simulink model "ModeAdjust"  (R2018b)
settings: Solver=FixedStepDiscrete  StartTime=0.0  StopTime=inf  FixedStep=0.01  RelTol=1e-3
undefined symbols (not defined in the file or in its folder): IfKeSMSbSeatMovBkRclnEnable_Val, IfKeSMSbSeatMovFrwdBkwdEnable_Val, IfKeSMSbSeatMovFtrstEnable_Val, IfKeSMSbSeatMovHdrstFrwdBkwdEnable_Val, IfKeSMSbSeatMovHdUpwdDnwdEnable_Val, IfKeSMSbSeatMovLgrstEnable_Val, IfKeSMSbSeatMovLtwdRtwdEnable_Val, IfVeSMSeStNumConfig, KeSMSbArmscreenMovEnable_Val, KeSMSbSeatMovLgrstExpdEnable_Val, KeSMSuFirstRwStBackPosDelta_Val, KeSMSuFirstRwStBackPosTolr_Val, KeSMSuFirstRwStCushFrntPosDelta_Val, KeSMSuFirstRwStCushFrntPosTolr_Val, KeSMSuFirstRwStCushRePosDelta_Val, KeSMSuFirstRwStCushRePosTolr_Val, KeSMSuFirstRwStFootrestPosDelta_Val, KeSMSuFirstRwStFootrestPosTolr_Val, KeSMSuFirstRwStFwdBkwdPosDelta_Val, KeSMSuFirstRwStFwdBkwdPosTolr_Val, KeSMSuMdMotFinshdTm_Val, KeSMSuMdRetryTm1_Val, KeSMSuModeReqDurgTm_Val, KeSMSuSecRwStArmTochPosDelta_Val, KeSMSuSecRwStArmTochPosTolr_Val, KeSMSuSecRwStBackPosDelta_Val, KeSMSuSecRwStBackPosTolr_Val, KeSMSuSecRwStFtrstUpwdDnwdPosDelta_Val, KeSMSuSecRwStFtrstUpwdDnwdPosTolr_Val, KeSMSuSecRwStFwdBkwdPosDelta_Val, KeSMSuSecRwStFwdBkwdPosTolr_Val, KeSMSuSecRwStHeadrestFwdBkwdPosDelta_Val, KeSMSuSecRwStHeadrestFwdBkwdPosTolr_Val, KeSMSuSecRwStHeadrestUpwdDwnwdPosDelta_Val, KeSMSuSecRwStHeadrestUpwdDwnwdPosTolr_Val, KeSMSuSecRwStLegrestInOutPosDelta_Val, KeSMSuSecRwStLegrestInOutPosTolr_Val, KeSMSuSecRwStLegrestUpwdDwnwdPosDelta_Val, KeSMSuSecRwStLegrestUpwdDwnwdPosTolr_Val, KeSMSuSecRwStLwdRwdPosDelta_Val, KeSMSuSecRwStLwdRwdPosTolr_Val, KeSMSuSecRwStVIPFtrstRefAngle_Val, KeSMSuThirdRwStFwdBkwdPosDelta_Val, KeSMSuThirdRwStFwdBkwdPosTolr_Val, KeSMSuThrdRwCushFoldPosDelta_Val, KeSMSuThrdRwCushFoldPosTolr_Val, KeSMSuThrdRwStBackPosDelta_Val, KeSMSuThrdRwStBackPosTolr_Val, KeSMSw4SLegrstCloseMdSecRwLtStFtrstUpwdDnwdPos_Val, KeSMSw4SLegrstCloseMdSecRwLtStFtrstUpwdDnwdPosMax_Val, KeSMSw4SLegrstCloseMdSecRwLtStFtrstUpwdDnwdPosMin_Val, KeSMSw4SLegrstCloseMdSecRwLtStLgrstOtwdInwdPos_Val, KeSMSw4SLegrstCloseMdSecRwLtStLgrstOtwdInwdPosMax_Val, KeSMSw4SLegrstCloseMdSecRwLtStLgrstOtwdInwdPosMin_Val, KeSMSw4SLegrstCloseMdSecRwLtStLgrstUpwdDnwdPos_Val, KeSMSw4SLegrstCloseMdSecRwLtStLgrstUpwdDnwdPosMax_Val, KeSMSw4SLegrstCloseMdSecRwLtStLgrstUpwdDnwdPosMin_Val, KeSMSw4SLegrstCloseMdSecRwRtStFtrstUpwdDnwdPos_Val, KeSMSw4SLegrstCloseMdSecRwRtStFtrstUpwdDnwdPosMax_Val, KeSMSw4SLegrstCloseMdSecRwRtStFtrstUpwdDnwdPosMin_Val ... (+1138)
libraries: Lib x401
(part 5 of 35)

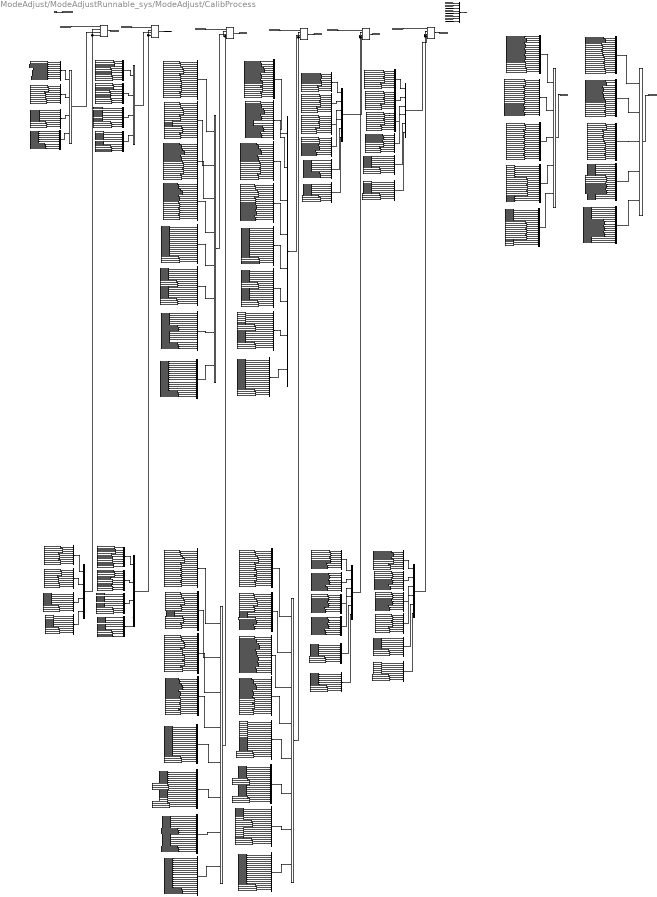
== system ModeAdjust/ModeAdjustRunnable_sys/ModeAdjust/CalibProcess ==
  note: 7S
  StNumConfig : Inport
  Bus Creator{,2..4,16..18,20..24,27..28,30..31,43..46,48..51,53..56,63..64,71..72,81..88} (40 alike) : BusCreator  Inputs=9
  Bus Creator{1,5,29,32} (4 alike) : BusCreator  Inputs=4
  Bus Creator{6..13,33..36,38..41,57..62,65..66,73..78,89..100} (42 alike) : BusCreator  Inputs=18
  Bus Creator{14..15,26,37,42} (5 alike) : BusCreator  Inputs=8
  Bus Creator{19,25,47,52} (4 alike) : BusCreator  Inputs=6
  Bus Creator79 : BusCreator  Inputs=5
  Bus Creator80 : BusCreator  Inputs=5
  Multiport Switch{1..4,6..7} (6 alike) : MultiPortSwitch  DataPortOrder=Specify indices  DataPortIndices={IfVeSMSeStNumConfig.SeatNum4Config,IfVeSMSeStNumConfig.SeatNum6Config,IfVeSMSeStNumConfig.SeatNum7Config}  DiagnosticForDefault=None
  PA_KeSMSw4SLegrstCloseMdSecRwLtStFtrstUpwdDnwdPosMax_Val : Constant  Value=KeSMSw4SLegrstCloseMdSecRwLtStFtrstUpwdDnwdPosMax_Val
  PA_KeSMSw4SLegrstCloseMdSecRwLtStFtrstUpwdDnwdPosMin_Val : Constant  Value=KeSMSw4SLegrstCloseMdSecRwLtStFtrstUpwdDnwdPosMin_Val
  PA_KeSMSw4SLegrstCloseMdSecRwLtStFtrstUpwdDnwdPos_Val : Constant  Value=KeSMSw4SLegrstCloseMdSecRwLtStFtrstUpwdDnwdPos_Val
  PA_KeSMSw4SLegrstCloseMdSecRwLtStLgrstOtwdInwdPosMax_Val : Constant  Value=KeSMSw4SLegrstCloseMdSecRwLtStLgrstOtwdInwdPosMax_Val
  PA_KeSMSw4SLegrstCloseMdSecRwLtStLgrstOtwdInwdPosMin_Val : Constant  Value=KeSMSw4SLegrstCloseMdSecRwLtStLgrstOtwdInwdPosMin_Val
  PA_KeSMSw4SLegrstCloseMdSecRwLtStLgrstOtwdInwdPos_Val : Constant  Value=KeSMSw4SLegrstCloseMdSecRwLtStLgrstOtwdInwdPos_Val
  PA_KeSMSw4SLegrstCloseMdSecRwLtStLgrstUpwdDnwdPosMax_Val : Constant  Value=KeSMSw4SLegrstCloseMdSecRwLtStLgrstUpwdDnwdPosMax_Val
  PA_KeSMSw4SLegrstCloseMdSecRwLtStLgrstUpwdDnwdPosMin_Val : Constant  Value=KeSMSw4SLegrstCloseMdSecRwLtStLgrstUpwdDnwdPosMin_Val
  PA_KeSMSw4SLegrstCloseMdSecRwLtStLgrstUpwdDnwdPos_Val : Constant  Value=KeSMSw4SLegrstCloseMdSecRwLtStLgrstUpwdDnwdPos_Val
  PA_KeSMSw4SLegrstCloseMdSecRwRtStFtrstUpwdDnwdPosMax_Val : Constant  Value=KeSMSw4SLegrstCloseMdSecRwRtStFtrstUpwdDnwdPosMax_Val
  PA_KeSMSw4SLegrstCloseMdSecRwRtStFtrstUpwdDnwdPosMin_Val : Constant  Value=KeSMSw4SLegrstCloseMdSecRwRtStFtrstUpwdDnwdPosMin_Val
  PA_KeSMSw4SLegrstCloseMdSecRwRtStFtrstUpwdDnwdPos_Val : Constant  Value=KeSMSw4SLegrstCloseMdSecRwRtStFtrstUpwdDnwdPos_Val
  PA_KeSMSw4SLegrstCloseMdSecRwRtStLgrstOtwdInwdPosMax_Val : Constant  Value=KeSMSw4SLegrstCloseMdSecRwRtStLgrstOtwdInwdPosMax_Val
  PA_KeSMSw4SLegrstCloseMdSecRwRtStLgrstOtwdInwdPosMin_Val : Constant  Value=KeSMSw4SLegrstCloseMdSecRwRtStLgrstOtwdInwdPosMin_Val
  PA_KeSMSw4SLegrstCloseMdSecRwRtStLgrstOtwdInwdPos_Val : Constant  Value=KeSMSw4SLegrstCloseMdSecRwRtStLgrstOtwdInwdPos_Val
  PA_KeSMSw4SLegrstCloseMdSecRwRtStLgrstUpwdDnwdPosMax_Val : Constant  Value=KeSMSw4SLegrstCloseMdSecRwRtStLgrstUpwdDnwdPosMax_Val
  PA_KeSMSw4SLegrstCloseMdSecRwRtStLgrstUpwdDnwdPosMin_Val : Constant  Value=KeSMSw4SLegrstCloseMdSecRwRtStLgrstUpwdDnwdPosMin_Val
  PA_KeSMSw4SLegrstCloseMdSecRwRtStLgrstUpwdDnwdPos_Val : Constant  Value=KeSMSw4SLegrstCloseMdSecRwRtStLgrstUpwdDnwdPos_Val
  PA_KeSMSw4SLegrstOpenMdSecRwLtStFtrstUpwdDnwdPosMax_Val : Constant  Value=KeSMSw4SLegrstOpenMdSecRwLtStFtrstUpwdDnwdPosMax_Val
  PA_KeSMSw4SLegrstOpenMdSecRwLtStFtrstUpwdDnwdPosMin_Val : Constant  Value=KeSMSw4SLegrstOpenMdSecRwLtStFtrstUpwdDnwdPosMin_Val
  PA_KeSMSw4SLegrstOpenMdSecRwLtStFtrstUpwdDnwdPos_Val : Constant  Value=KeSMSw4SLegrstOpenMdSecRwLtStFtrstUpwdDnwdPos_Val
  PA_KeSMSw4SLegrstOpenMdSecRwLtStLgrstOtwdInwdPosMax_Val : Constant  Value=KeSMSw4SLegrstOpenMdSecRwLtStLgrstOtwdInwdPosMax_Val
  PA_KeSMSw4SLegrstOpenMdSecRwLtStLgrstOtwdInwdPosMin_Val : Constant  Value=KeSMSw4SLegrstOpenMdSecRwLtStLgrstOtwdInwdPosMin_Val
  PA_KeSMSw4SLegrstOpenMdSecRwLtStLgrstOtwdInwdPos_Val : Constant  Value=KeSMSw4SLegrstOpenMdSecRwLtStLgrstOtwdInwdPos_Val
  PA_KeSMSw4SLegrstOpenMdSecRwLtStLgrstUpwdDnwdPosMax_Val : Constant  Value=KeSMSw4SLegrstOpenMdSecRwLtStLgrstUpwdDnwdPosMax_Val
  PA_KeSMSw4SLegrstOpenMdSecRwLtStLgrstUpwdDnwdPosMin_Val : Constant  Value=KeSMSw4SLegrstOpenMdSecRwLtStLgrstUpwdDnwdPosMin_Val
  PA_KeSMSw4SLegrstOpenMdSecRwLtStLgrstUpwdDnwdPos_Val : Constant  Value=KeSMSw4SLegrstOpenMdSecRwLtStLgrstUpwdDnwdPos_Val
  PA_KeSMSw4SLegrstOpenMdSecRwRtStFtrstUpwdDnwdPosMax_Val : Constant  Value=KeSMSw4SLegrstOpenMdSecRwRtStFtrstUpwdDnwdPosMax_Val
  PA_KeSMSw4SLegrstOpenMdSecRwRtStFtrstUpwdDnwdPosMin_Val : Constant  Value=KeSMSw4SLegrstOpenMdSecRwRtStFtrstUpwdDnwdPosMin_Val
  PA_KeSMSw4SLegrstOpenMdSecRwRtStFtrstUpwdDnwdPos_Val : Constant  Value=KeSMSw4SLegrstOpenMdSecRwRtStFtrstUpwdDnwdPos_Val
  PA_KeSMSw4SLegrstOpenMdSecRwRtStLgrstOtwdInwdPosMax_Val : Constant  Value=KeSMSw4SLegrstOpenMdSecRwRtStLgrstOtwdInwdPosMax_Val
  PA_KeSMSw4SLegrstOpenMdSecRwRtStLgrstOtwdInwdPosMin_Val : Constant  Value=KeSMSw4SLegrstOpenMdSecRwRtStLgrstOtwdInwdPosMin_Val
  PA_KeSMSw4SLegrstOpenMdSecRwRtStLgrstOtwdInwdPos_Val : Constant  Value=KeSMSw4SLegrstOpenMdSecRwRtStLgrstOtwdInwdPos_Val
  PA_KeSMSw4SLegrstOpenMdSecRwRtStLgrstUpwdDnwdPosMax_Val : Constant  Value=KeSMSw4SLegrstOpenMdSecRwRtStLgrstUpwdDnwdPosMax_Val
  PA_KeSMSw4SLegrstOpenMdSecRwRtStLgrstUpwdDnwdPosMin_Val : Constant  Value=KeSMSw4SLegrstOpenMdSecRwRtStLgrstUpwdDnwdPosMin_Val
  PA_KeSMSw4SLegrstOpenMdSecRwRtStLgrstUpwdDnwdPos_Val : Constant  Value=KeSMSw4SLegrstOpenMdSecRwRtStLgrstUpwdDnwdPos_Val
  PA_KeSMSw4sLyingMDSecRwLtStBkReclnUpwdDnwdPosMax_Val : Constant  Value=KeSMSw4sLyingMDSecRwLtStBkReclnUpwdDnwdPosMax_Val
  PA_KeSMSw4sLyingMDSecRwLtStBkReclnUpwdDnwdPosMin_Val : Constant  Value=KeSMSw4sLyingMDSecRwLtStBkReclnUpwdDnwdPosMin_Val
  PA_KeSMSw4sLyingMDSecRwLtStBkReclnUpwdDnwdPos_Val : Constant  Value=KeSMSw4sLyingMDSecRwLtStBkReclnUpwdDnwdPos_Val
  PA_KeSMSw4sLyingMDSecRwLtStFtrstUpwdDnwdPosMax_Val : Constant  Value=KeSMSw4sLyingMDSecRwLtStFtrstUpwdDnwdPosMax_Val
  PA_KeSMSw4sLyingMDSecRwLtStFtrstUpwdDnwdPosMin_Val : Constant  Value=KeSMSw4sLyingMDSecRwLtStFtrstUpwdDnwdPosMin_Val
  PA_KeSMSw4sLyingMDSecRwLtStFtrstUpwdDnwdPos_Val : Constant  Value=KeSMSw4sLyingMDSecRwLtStFtrstUpwdDnwdPos_Val
  PA_KeSMSw4sLyingMDSecRwLtStHdrstFrwdBkwdnwdPosMax_Val : Constant  Value=KeSMSw4sLyingMDSecRwLtStHdrstFrwdBkwdnwdPosMax_Val
  PA_KeSMSw4sLyingMDSecRwLtStHdrstFrwdBkwdnwdPosMin_Val : Constant  Value=KeSMSw4sLyingMDSecRwLtStHdrstFrwdBkwdnwdPosMin_Val
  PA_KeSMSw4sLyingMDSecRwLtStHdrstFrwdBkwdnwdPos_Val : Constant  Value=KeSMSw4sLyingMDSecRwLtStHdrstFrwdBkwdnwdPos_Val
  PA_KeSMSw4sLyingMDSecRwLtStHdrstUpwdDnwdPosMax_Val : Constant  Value=KeSMSw4sLyingMDSecRwLtStHdrstUpwdDnwdPosMax_Val
  PA_KeSMSw4sLyingMDSecRwLtStHdrstUpwdDnwdPosMin_Val : Constant  Value=KeSMSw4sLyingMDSecRwLtStHdrstUpwdDnwdPosMin_Val
  PA_KeSMSw4sLyingMDSecRwLtStHdrstUpwdDnwdPos_Val : Constant  Value=KeSMSw4sLyingMDSecRwLtStHdrstUpwdDnwdPos_Val
  PA_KeSMSw4sLyingMDSecRwLtStLgrstOtwdInwdPosMax_Val : Constant  Value=KeSMSw4sLyingMDSecRwLtStLgrstOtwdInwdPosMax_Val
  PA_KeSMSw4sLyingMDSecRwLtStLgrstOtwdInwdPosMin_Val : Constant  Value=KeSMSw4sLyingMDSecRwLtStLgrstOtwdInwdPosMin_Val
  PA_KeSMSw4sLyingMDSecRwLtStLgrstOtwdInwdPos_Val : Constant  Value=KeSMSw4sLyingMDSecRwLtStLgrstOtwdInwdPos_Val
  PA_KeSMSw4sLyingMDSecRwLtStLgrstUpwdDnwdPosMax_Val : Constant  Value=KeSMSw4sLyingMDSecRwLtStLgrstUpwdDnwdPosMax_Val
  PA_KeSMSw4sLyingMDSecRwLtStLgrstUpwdDnwdPosMin_Val : Constant  Value=KeSMSw4sLyingMDSecRwLtStLgrstUpwdDnwdPosMin_Val
  PA_KeSMSw4sLyingMDSecRwLtStLgrstUpwdDnwdPos_Val : Constant  Value=KeSMSw4sLyingMDSecRwLtStLgrstUpwdDnwdPos_Val
  PA_KeSMSw4sLyingMDSecRwRtStBkReclnUpwdDnwdPosMax_Val : Constant  Value=KeSMSw4sLyingMDSecRwRtStBkReclnUpwdDnwdPosMax_Val
  PA_KeSMSw4sLyingMDSecRwRtStBkReclnUpwdDnwdPosMin_Val : Constant  Value=KeSMSw4sLyingMDSecRwRtStBkReclnUpwdDnwdPosMin_Val
  PA_KeSMSw4sLyingMDSecRwRtStBkReclnUpwdDnwdPos_Val : Constant  Value=KeSMSw4sLyingMDSecRwRtStBkReclnUpwdDnwdPos_Val
  PA_KeSMSw4sLyingMDSecRwRtStFtrstUpwdDnwdPosMax_Val : Constant  Value=KeSMSw4sLyingMDSecRwRtStFtrstUpwdDnwdPosMax_Val
  PA_KeSMSw4sLyingMDSecRwRtStFtrstUpwdDnwdPosMin_Val : Constant  Value=KeSMSw4sLyingMDSecRwRtStFtrstUpwdDnwdPosMin_Val
  PA_KeSMSw4sLyingMDSecRwRtStFtrstUpwdDnwdPos_Val : Constant  Value=KeSMSw4sLyingMDSecRwRtStFtrstUpwdDnwdPos_Val
  PA_KeSMSw4sLyingMDSecRwRtStHdrstFrwdBkwdnwdPosMax_Val : Constant  Value=KeSMSw4sLyingMDSecRwRtStHdrstFrwdBkwdnwdPosMax_Val
  PA_KeSMSw4sLyingMDSecRwRtStHdrstFrwdBkwdnwdPosMin_Val : Constant  Value=KeSMSw4sLyingMDSecRwRtStHdrstFrwdBkwdnwdPosMin_Val
  PA_KeSMSw4sLyingMDSecRwRtStHdrstFrwdBkwdnwdPos_Val : Constant  Value=KeSMSw4sLyingMDSecRwRtStHdrstFrwdBkwdnwdPos_Val
  PA_KeSMSw4sLyingMDSecRwRtStHdrstUpwdPosMax_Val : Constant  Value=KeSMSw4sLyingMDSecRwRtStHdrstUpwdPosMax_Val
  PA_KeSMSw4sLyingMDSecRwRtStHdrstUpwdPosMin_Val : Constant  Value=KeSMSw4sLyingMDSecRwRtStHdrstUpwdPosMin_Val
  PA_KeSMSw4sLyingMDSecRwRtStHdrstUpwdPos_Val : Constant  Value=KeSMSw4sLyingMDSecRwRtStHdrstUpwdPos_Val
  PA_KeSMSw4sLyingMDSecRwRtStLgrstOtwdInwdPosMax_Val : Constant  Value=KeSMSw4sLyingMDSecRwRtStLgrstOtwdInwdPosMax_Val
  PA_KeSMSw4sLyingMDSecRwRtStLgrstOtwdInwdPosMin_Val : Constant  Value=KeSMSw4sLyingMDSecRwRtStLgrstOtwdInwdPosMin_Val
  PA_KeSMSw4sLyingMDSecRwRtStLgrstOtwdInwdPos_Val : Constant  Value=KeSMSw4sLyingMDSecRwRtStLgrstOtwdInwdPos_Val
  PA_KeSMSw4sLyingMDSecRwRtStLgrstUpwdPosMax_Val : Constant  Value=KeSMSw4sLyingMDSecRwRtStLgrstUpwdPosMax_Val
  PA_KeSMSw4sLyingMDSecRwRtStLgrstUpwdPosMin_Val : Constant  Value=KeSMSw4sLyingMDSecRwRtStLgrstUpwdPosMin_Val
  PA_KeSMSw4sLyingMDSecRwRtStLgrstUpwdPos_Val : Constant  Value=KeSMSw4sLyingMDSecRwRtStLgrstUpwdPos_Val
  PA_KeSMSw4sRecoveryMDSecRwLtStBkReclnUpwdDnwdPosMax_Val : Constant  Value=KeSMSw4sRecoveryMDSecRwLtStBkReclnUpwdDnwdPosMax_Val
  PA_KeSMSw4sRecoveryMDSecRwLtStBkReclnUpwdDnwdPosMin_Val : Constant  Value=KeSMSw4sRecoveryMDSecRwLtStBkReclnUpwdDnwdPosMin_Val
  PA_KeSMSw4sRecoveryMDSecRwLtStBkReclnUpwdDnwdPos_Val : Constant  Value=KeSMSw4sRecoveryMDSecRwLtStBkReclnUpwdDnwdPos_Val
  PA_KeSMSw4sRecoveryMDSecRwLtStFtrstUpwdDnwdPosMax_Val : Constant  Value=KeSMSw4sRecoveryMDSecRwLtStFtrstUpwdDnwdPosMax_Val
  PA_KeSMSw4sRecoveryMDSecRwLtStFtrstUpwdDnwdPosMin_Val : Constant  Value=KeSMSw4sRecoveryMDSecRwLtStFtrstUpwdDnwdPosMin_Val
  PA_KeSMSw4sRecoveryMDSecRwLtStFtrstUpwdDnwdPos_Val : Constant  Value=KeSMSw4sRecoveryMDSecRwLtStFtrstUpwdDnwdPos_Val
  PA_KeSMSw4sRecoveryMDSecRwLtStHdrstFrwdBkwdPosMax_Val : Constant  Value=KeSMSw4sRecoveryMDSecRwLtStHdrstFrwdBkwdPosMax_Val
  PA_KeSMSw4sRecoveryMDSecRwLtStHdrstFrwdBkwdPosMin_Val : Constant  Value=KeSMSw4sRecoveryMDSecRwLtStHdrstFrwdBkwdPosMin_Val
  PA_KeSMSw4sRecoveryMDSecRwLtStHdrstFrwdBkwdPos_Val : Constant  Value=KeSMSw4sRecoveryMDSecRwLtStHdrstFrwdBkwdPos_Val
  PA_KeSMSw4sRecoveryMDSecRwLtStHdrstUpwdDnwdPosMax_Val : Constant  Value=KeSMSw4sRecoveryMDSecRwLtStHdrstUpwdDnwdPosMax_Val
  PA_KeSMSw4sRecoveryMDSecRwLtStHdrstUpwdDnwdPosMin_Val : Constant  Value=KeSMSw4sRecoveryMDSecRwLtStHdrstUpwdDnwdPosMin_Val
  PA_KeSMSw4sRecoveryMDSecRwLtStHdrstUpwdDnwdPos_Val : Constant  Value=KeSMSw4sRecoveryMDSecRwLtStHdrstUpwdDnwdPos_Val
  PA_KeSMSw4sRecoveryMDSecRwLtStLgrstOtwdInwdPosMax_Val : Constant  Value=KeSMSw4sRecoveryMDSecRwLtStLgrstOtwdInwdPosMax_Val
  PA_KeSMSw4sRecoveryMDSecRwLtStLgrstOtwdInwdPosMin_Val : Constant  Value=KeSMSw4sRecoveryMDSecRwLtStLgrstOtwdInwdPosMin_Val
  PA_KeSMSw4sRecoveryMDSecRwLtStLgrstOtwdInwdPos_Val : Constant  Value=KeSMSw4sRecoveryMDSecRwLtStLgrstOtwdInwdPos_Val
  PA_KeSMSw4sRecoveryMDSecRwLtStLgrstUpwdDnwdPosMax_Val : Constant  Value=KeSMSw4sRecoveryMDSecRwLtStLgrstUpwdDnwdPosMax_Val
  PA_KeSMSw4sRecoveryMDSecRwLtStLgrstUpwdDnwdPosMin_Val : Constant  Value=KeSMSw4sRecoveryMDSecRwLtStLgrstUpwdDnwdPosMin_Val
  PA_KeSMSw4sRecoveryMDSecRwLtStLgrstUpwdDnwdPos_Val : Constant  Value=KeSMSw4sRecoveryMDSecRwLtStLgrstUpwdDnwdPos_Val
  PA_KeSMSw4sRecoveryMDSecRwRtStBkReclnUpwdDnwdPosMax_Val : Constant  Value=KeSMSw4sRecoveryMDSecRwRtStBkReclnUpwdDnwdPosMax_Val
  PA_KeSMSw4sRecoveryMDSecRwRtStBkReclnUpwdDnwdPosMin_Val : Constant  Value=KeSMSw4sRecoveryMDSecRwRtStBkReclnUpwdDnwdPosMin_Val
  PA_KeSMSw4sRecoveryMDSecRwRtStBkReclnUpwdDnwdPos_Val : Constant  Value=KeSMSw4sRecoveryMDSecRwRtStBkReclnUpwdDnwdPos_Val
  PA_KeSMSw4sRecoveryMDSecRwRtStFtrstUpwdDnwdPosMax_Val : Constant  Value=KeSMSw4sRecoveryMDSecRwRtStFtrstUpwdDnwdPosMax_Val
  PA_KeSMSw4sRecoveryMDSecRwRtStFtrstUpwdDnwdPosMin_Val : Constant  Value=KeSMSw4sRecoveryMDSecRwRtStFtrstUpwdDnwdPosMin_Val
  PA_KeSMSw4sRecoveryMDSecRwRtStFtrstUpwdDnwdPos_Val : Constant  Value=KeSMSw4sRecoveryMDSecRwRtStFtrstUpwdDnwdPos_Val
  PA_KeSMSw4sRecoveryMDSecRwRtStHdrstFrwdBkwdPosMax_Val : Constant  Value=KeSMSw4sRecoveryMDSecRwRtStHdrstFrwdBkwdPosMax_Val
  PA_KeSMSw4sRecoveryMDSecRwRtStHdrstFrwdBkwdPosMin_Val : Constant  Value=KeSMSw4sRecoveryMDSecRwRtStHdrstFrwdBkwdPosMin_Val
  PA_KeSMSw4sRecoveryMDSecRwRtStHdrstFrwdBkwdPos_Val : Constant  Value=KeSMSw4sRecoveryMDSecRwRtStHdrstFrwdBkwdPos_Val
  PA_KeSMSw4sRecoveryMDSecRwRtStHdrstUpwdPosMax_Val : Constant  Value=KeSMSw4sRecoveryMDSecRwRtStHdrstUpwdPosMax_Val
  PA_KeSMSw4sRecoveryMDSecRwRtStHdrstUpwdPosMin_Val : Constant  Value=KeSMSw4sRecoveryMDSecRwRtStHdrstUpwdPosMin_Val
  PA_KeSMSw4sRecoveryMDSecRwRtStHdrstUpwdPos_Val : Constant  Value=KeSMSw4sRecoveryMDSecRwRtStHdrstUpwdPos_Val
  PA_KeSMSw4sRecoveryMDSecRwRtStLgrstOtwdInwdPosMax_Val : Constant  Value=KeSMSw4sRecoveryMDSecRwRtStLgrstOtwdInwdPosMax_Val
  PA_KeSMSw4sRecoveryMDSecRwRtStLgrstOtwdInwdPosMin_Val : Constant  Value=KeSMSw4sRecoveryMDSecRwRtStLgrstOtwdInwdPosMin_Val
  PA_KeSMSw4sRecoveryMDSecRwRtStLgrstOtwdInwdPos_Val : Constant  Value=KeSMSw4sRecoveryMDSecRwRtStLgrstOtwdInwdPos_Val
  PA_KeSMSw4sRecoveryMDSecRwRtStLgrstUpwdPosMax_Val : Constant  Value=KeSMSw4sRecoveryMDSecRwRtStLgrstUpwdPosMax_Val
  PA_KeSMSw4sRecoveryMDSecRwRtStLgrstUpwdPosMin_Val : Constant  Value=KeSMSw4sRecoveryMDSecRwRtStLgrstUpwdPosMin_Val
  PA_KeSMSw4sRecoveryMDSecRwRtStLgrstUpwdPos_Val : Constant  Value=KeSMSw4sRecoveryMDSecRwRtStLgrstUpwdPos_Val
  PA_KeSMSw4sVIPMDSecRwLtStBkReclnUpwdDnwdPosMax_Val : Constant  Value=KeSMSw4sVIPMDSecRwLtStBkReclnUpwdDnwdPosMax_Val
  PA_KeSMSw4sVIPMDSecRwLtStBkReclnUpwdDnwdPosMin_Val : Constant  Value=KeSMSw4sVIPMDSecRwLtStBkReclnUpwdDnwdPosMin_Val
  PA_KeSMSw4sVIPMDSecRwLtStBkReclnUpwdDnwdPos_Val : Constant  Value=KeSMSw4sVIPMDSecRwLtStBkReclnUpwdDnwdPos_Val
  PA_KeSMSw4sVIPMDSecRwLtStFtrstUpwdDnwdPosMax_Val : Constant  Value=KeSMSw4sVIPMDSecRwLtStFtrstUpwdDnwdPosMax_Val
  PA_KeSMSw4sVIPMDSecRwLtStFtrstUpwdDnwdPosMin_Val : Constant  Value=KeSMSw4sVIPMDSecRwLtStFtrstUpwdDnwdPosMin_Val
  PA_KeSMSw4sVIPMDSecRwLtStFtrstUpwdDnwdPos_Val : Constant  Value=KeSMSw4sVIPMDSecRwLtStFtrstUpwdDnwdPos_Val
  PA_KeSMSw4sVIPMDSecRwLtStHdrstFrwdBkwdPosMax_Val : Constant  Value=KeSMSw4sVIPMDSecRwLtStHdrstFrwdBkwdPosMax_Val
  PA_KeSMSw4sVIPMDSecRwLtStHdrstFrwdBkwdPosMin_Val : Constant  Value=KeSMSw4sVIPMDSecRwLtStHdrstFrwdBkwdPosMin_Val
  PA_KeSMSw4sVIPMDSecRwLtStHdrstFrwdBkwdPos_Val : Constant  Value=KeSMSw4sVIPMDSecRwLtStHdrstFrwdBkwdPos_Val
  PA_KeSMSw4sVIPMDSecRwLtStHdrstUpwdDnwdPosMax_Val : Constant  Value=KeSMSw4sVIPMDSecRwLtStHdrstUpwdDnwdPosMax_Val
  PA_KeSMSw4sVIPMDSecRwLtStHdrstUpwdDnwdPosMin_Val : Constant  Value=KeSMSw4sVIPMDSecRwLtStHdrstUpwdDnwdPosMin_Val
  PA_KeSMSw4sVIPMDSecRwLtStHdrstUpwdDnwdPos_Val : Constant  Value=KeSMSw4sVIPMDSecRwLtStHdrstUpwdDnwdPos_Val
  PA_KeSMSw4sVIPMDSecRwLtStLgrstOtwdInwdPosMax_Val : Constant  Value=KeSMSw4sVIPMDSecRwLtStLgrstOtwdInwdPosMax_Val
  PA_KeSMSw4sVIPMDSecRwLtStLgrstOtwdInwdPosMin_Val : Constant  Value=KeSMSw4sVIPMDSecRwLtStLgrstOtwdInwdPosMin_Val
  PA_KeSMSw4sVIPMDSecRwLtStLgrstOtwdInwdPos_Val : Constant  Value=KeSMSw4sVIPMDSecRwLtStLgrstOtwdInwdPos_Val
  PA_KeSMSw4sVIPMDSecRwLtStLgrstUpwdDnwdPosMax_Val : Constant  Value=KeSMSw4sVIPMDSecRwLtStLgrstUpwdDnwdPosMax_Val
  PA_KeSMSw4sVIPMDSecRwLtStLgrstUpwdDnwdPosMin_Val : Constant  Value=KeSMSw4sVIPMDSecRwLtStLgrstUpwdDnwdPosMin_Val
  PA_KeSMSw4sVIPMDSecRwLtStLgrstUpwdDnwdPos_Val : Constant  Value=KeSMSw4sVIPMDSecRwLtStLgrstUpwdDnwdPos_Val
  PA_KeSMSw4sVIPMDSecRwRtStBkReclnUpwdDnwdPosMax_Val : Constant  Value=KeSMSw4sVIPMDSecRwRtStBkReclnUpwdDnwdPosMax_Val
  PA_KeSMSw4sVIPMDSecRwRtStBkReclnUpwdDnwdPosMin_Val : Constant  Value=KeSMSw4sVIPMDSecRwRtStBkReclnUpwdDnwdPosMin_Val
  PA_KeSMSw4sVIPMDSecRwRtStBkReclnUpwdDnwdPos_Val : Constant  Value=KeSMSw4sVIPMDSecRwRtStBkReclnUpwdDnwdPos_Val
  PA_KeSMSw4sVIPMDSecRwRtStFtrstUpwdDnwdPosMax_Val : Constant  Value=KeSMSw4sVIPMDSecRwRtStFtrstUpwdDnwdPosMax_Val
  PA_KeSMSw4sVIPMDSecRwRtStFtrstUpwdDnwdPosMin_Val : Constant  Value=KeSMSw4sVIPMDSecRwRtStFtrstUpwdDnwdPosMin_Val
  PA_KeSMSw4sVIPMDSecRwRtStFtrstUpwdDnwdPos_Val : Constant  Value=KeSMSw4sVIPMDSecRwRtStFtrstUpwdDnwdPos_Val
  PA_KeSMSw4sVIPMDSecRwRtStHdrstFrwdBkwdPosMax_Val : Constant  Value=KeSMSw4sVIPMDSecRwRtStHdrstFrwdBkwdPosMax_Val
  PA_KeSMSw4sVIPMDSecRwRtStHdrstFrwdBkwdPosMin_Val : Constant  Value=KeSMSw4sVIPMDSecRwRtStHdrstFrwdBkwdPosMin_Val
  PA_KeSMSw4sVIPMDSecRwRtStHdrstFrwdBkwdPos_Val : Constant  Value=KeSMSw4sVIPMDSecRwRtStHdrstFrwdBkwdPos_Val
  PA_KeSMSw4sVIPMDSecRwRtStHdrstUpwdPosMax_Val : Constant  Value=KeSMSw4sVIPMDSecRwRtStHdrstUpwdPosMax_Val
  PA_KeSMSw4sVIPMDSecRwRtStHdrstUpwdPosMin_Val : Constant  Value=KeSMSw4sVIPMDSecRwRtStHdrstUpwdPosMin_Val
  PA_KeSMSw4sVIPMDSecRwRtStHdrstUpwdPos_Val : Constant  Value=KeSMSw4sVIPMDSecRwRtStHdrstUpwdPos_Val
  PA_KeSMSw4sVIPMDSecRwRtStLgrstOtwdInwdPosMax_Val : Constant  Value=KeSMSw4sVIPMDSecRwRtStLgrstOtwdInwdPosMax_Val
  PA_KeSMSw4sVIPMDSecRwRtStLgrstOtwdInwdPosMin_Val : Constant  Value=KeSMSw4sVIPMDSecRwRtStLgrstOtwdInwdPosMin_Val
  PA_KeSMSw4sVIPMDSecRwRtStLgrstOtwdInwdPos_Val : Constant  Value=KeSMSw4sVIPMDSecRwRtStLgrstOtwdInwdPos_Val
  PA_KeSMSw4sVIPMDSecRwRtStLgrstUpwdPosMax_Val : Constant  Value=KeSMSw4sVIPMDSecRwRtStLgrstUpwdPosMax_Val
  PA_KeSMSw4sVIPMDSecRwRtStLgrstUpwdPosMin_Val : Constant  Value=KeSMSw4sVIPMDSecRwRtStLgrstUpwdPosMin_Val
  PA_KeSMSw4sVIPMDSecRwRtStLgrstUpwdPos_Val : Constant  Value=KeSMSw4sVIPMDSecRwRtStLgrstUpwdPos_Val
  PA_KeSMSw6sAcsEntryDrvStBkReclnUpwdDnwdPosMax_Val : Constant  Value=KeSMSw6sAcsEntryDrvStBkReclnUpwdDnwdPosMax_Val
  PA_KeSMSw6sAcsEntryDrvStBkReclnUpwdDnwdPosMin_Val : Constant  Value=KeSMSw6sAcsEntryDrvStBkReclnUpwdDnwdPosMin_Val
  PA_KeSMSw6sAcsEntryDrvStBkReclnUpwdDnwdPos_Val : Constant  Value=KeSMSw6sAcsEntryDrvStBkReclnUpwdDnwdPos_Val
  PA_KeSMSw6sAcsEntryDrvStFrwdBkwdPosMax_Val : Constant  Value=KeSMSw6sAcsEntryDrvStFrwdBkwdPosMax_Val
  PA_KeSMSw6sAcsEntryDrvStFrwdBkwdPosMin_Val : Constant  Value=KeSMSw6sAcsEntryDrvStFrwdBkwdPosMin_Val
  PA_KeSMSw6sAcsEntryDrvStFrwdBkwdPos_Val : Constant  Value=KeSMSw6sAcsEntryDrvStFrwdBkwdPos_Val
  PA_KeSMSw6sAcsEntryDrvStFtUpwdDnwdPosMax_Val : Constant  Value=KeSMSw6sAcsEntryDrvStFtUpwdDnwdPosMax_Val
  PA_KeSMSw6sAcsEntryDrvStFtUpwdDnwdPosMin_Val : Constant  Value=KeSMSw6sAcsEntryDrvStFtUpwdDnwdPosMin_Val
  PA_KeSMSw6sAcsEntryDrvStFtUpwdDnwdPos_Val : Constant  Value=KeSMSw6sAcsEntryDrvStFtUpwdDnwdPos_Val
  PA_KeSMSw6sAcsEntryPassStBkReclnUpwdDnwdPosMax_Val : Constant  Value=KeSMSw6sAcsEntryPassStBkReclnUpwdDnwdPosMax_Val
  PA_KeSMSw6sAcsEntryPassStBkReclnUpwdDnwdPosMin_Val : Constant  Value=KeSMSw6sAcsEntryPassStBkReclnUpwdDnwdPosMin_Val
  PA_KeSMSw6sAcsEntryPassStBkReclnUpwdDnwdPos_Val : Constant  Value=KeSMSw6sAcsEntryPassStBkReclnUpwdDnwdPos_Val
  PA_KeSMSw6sAcsEntryPassStFrwdBkwdPosMax_Val : Constant  Value=KeSMSw6sAcsEntryPassStFrwdBkwdPosMax_Val
  PA_KeSMSw6sAcsEntryPassStFrwdBkwdPosMin_Val : Constant  Value=KeSMSw6sAcsEntryPassStFrwdBkwdPosMin_Val
  PA_KeSMSw6sAcsEntryPassStFrwdBkwdPos_Val : Constant  Value=KeSMSw6sAcsEntryPassStFrwdBkwdPos_Val
  PA_KeSMSw6sAcsEntryPassStFtUpwdDnwdPosMiax_Val : Constant  Value=KeSMSw6sAcsEntryPassStFtUpwdDnwdPosMiax_Val
  PA_KeSMSw6sAcsEntryPassStFtUpwdDnwdPosMin_Val : Constant  Value=KeSMSw6sAcsEntryPassStFtUpwdDnwdPosMin_Val
  PA_KeSMSw6sAcsEntryPassStFtUpwdDnwdPos_Val : Constant  Value=KeSMSw6sAcsEntryPassStFtUpwdDnwdPos_Val
  PA_KeSMSw6sAcsEntrySecRwLtStArmScrnPosMax_Val : Constant  Value=KeSMSw6sAcsEntrySecRwLtStArmScrnPosMax_Val
  PA_KeSMSw6sAcsEntrySecRwLtStArmScrnPosMin_Val : Constant  Value=KeSMSw6sAcsEntrySecRwLtStArmScrnPosMin_Val
  PA_KeSMSw6sAcsEntrySecRwLtStArmScrnPos_Val : Constant  Value=KeSMSw6sAcsEntrySecRwLtStArmScrnPos_Val
  PA_KeSMSw6sAcsEntrySecRwLtStBkReclnUpwdDnwdPosMax_Val : Constant  Value=KeSMSw6sAcsEntrySecRwLtStBkReclnUpwdDnwdPosMax_Val
  PA_KeSMSw6sAcsEntrySecRwLtStBkReclnUpwdDnwdPosMin_Val : Constant  Value=KeSMSw6sAcsEntrySecRwLtStBkReclnUpwdDnwdPosMin_Val
  PA_KeSMSw6sAcsEntrySecRwLtStBkReclnUpwdDnwdPos_Val : Constant  Value=KeSMSw6sAcsEntrySecRwLtStBkReclnUpwdDnwdPos_Val
  PA_KeSMSw6sAcsEntrySecRwLtStFrwdBkwdPosMax_Val : Constant  Value=KeSMSw6sAcsEntrySecRwLtStFrwdBkwdPosMax_Val
  PA_KeSMSw6sAcsEntrySecRwLtStFrwdBkwdPosMin_Val : Constant  Value=KeSMSw6sAcsEntrySecRwLtStFrwdBkwdPosMin_Val
  PA_KeSMSw6sAcsEntrySecRwLtStFrwdBkwdPos_Val : Constant  Value=KeSMSw6sAcsEntrySecRwLtStFrwdBkwdPos_Val
  PA_KeSMSw6sAcsEntrySecRwLtStHdrstUpwdPosMax_Val : Constant  Value=KeSMSw6sAcsEntrySecRwLtStHdrstUpwdPosMax_Val
  PA_KeSMSw6sAcsEntrySecRwLtStHdrstUpwdPosMin_Val : Constant  Value=KeSMSw6sAcsEntrySecRwLtStHdrstUpwdPosMin_Val
  PA_KeSMSw6sAcsEntrySecRwLtStHdrstUpwdPos_Val : Constant  Value=KeSMSw6sAcsEntrySecRwLtStHdrstUpwdPos_Val
  PA_KeSMSw6sAcsEntrySecRwLtStLgrstUpwdPosMax_Val : Constant  Value=KeSMSw6sAcsEntrySecRwLtStLgrstUpwdPosMax_Val
  PA_KeSMSw6sAcsEntrySecRwLtStLgrstUpwdPosMin_Val : Constant  Value=KeSMSw6sAcsEntrySecRwLtStLgrstUpwdPosMin_Val
  PA_KeSMSw6sAcsEntrySecRwLtStLgrstUpwdPos_Val : Constant  Value=KeSMSw6sAcsEntrySecRwLtStLgrstUpwdPos_Val
  PA_KeSMSw6sAcsEntrySecRwLtStLtwdRtwdPosMax_Val : Constant  Value=KeSMSw6sAcsEntrySecRwLtStLtwdRtwdPosMax_Val
  PA_KeSMSw6sAcsEntrySecRwLtStLtwdRtwdPosMin_Val : Constant  Value=KeSMSw6sAcsEntrySecRwLtStLtwdRtwdPosMin_Val
  PA_KeSMSw6sAcsEntrySecRwLtStLtwdRtwdPos_Val : Constant  Value=KeSMSw6sAcsEntrySecRwLtStLtwdRtwdPos_Val
  PA_KeSMSw6sAcsEntrySecRwRtStArmScrnPosMax_Val : Constant  Value=KeSMSw6sAcsEntrySecRwRtStArmScrnPosMax_Val
  PA_KeSMSw6sAcsEntrySecRwRtStArmScrnPosMin_Val : Constant  Value=KeSMSw6sAcsEntrySecRwRtStArmScrnPosMin_Val
  PA_KeSMSw6sAcsEntrySecRwRtStArmScrnPos_Val : Constant  Value=KeSMSw6sAcsEntrySecRwRtStArmScrnPos_Val
  PA_KeSMSw6sAcsEntrySecRwRtStBkReclnUpwdDnwdPosMax_Val : Constant  Value=KeSMSw6sAcsEntrySecRwRtStBkReclnUpwdDnwdPosMax_Val
  PA_KeSMSw6sAcsEntrySecRwRtStBkReclnUpwdDnwdPosMin_Val : Constant  Value=KeSMSw6sAcsEntrySecRwRtStBkReclnUpwdDnwdPosMin_Val
  PA_KeSMSw6sAcsEntrySecRwRtStBkReclnUpwdDnwdPos_Val : Constant  Value=KeSMSw6sAcsEntrySecRwRtStBkReclnUpwdDnwdPos_Val
  PA_KeSMSw6sAcsEntrySecRwRtStFrwdBkwdPosMax_Val : Constant  Value=KeSMSw6sAcsEntrySecRwRtStFrwdBkwdPosMax_Val
  PA_KeSMSw6sAcsEntrySecRwRtStFrwdBkwdPosMin_Val : Constant  Value=KeSMSw6sAcsEntrySecRwRtStFrwdBkwdPosMin_Val
  PA_KeSMSw6sAcsEntrySecRwRtStFrwdBkwdPos_Val : Constant  Value=KeSMSw6sAcsEntrySecRwRtStFrwdBkwdPos_Val
  PA_KeSMSw6sAcsEntrySecRwRtStHdrstUpwdPosMax_Val : Constant  Value=KeSMSw6sAcsEntrySecRwRtStHdrstUpwdPosMax_Val
  PA_KeSMSw6sAcsEntrySecRwRtStHdrstUpwdPosMin_Val : Constant  Value=KeSMSw6sAcsEntrySecRwRtStHdrstUpwdPosMin_Val
  PA_KeSMSw6sAcsEntrySecRwRtStHdrstUpwdPos_Val : Constant  Value=KeSMSw6sAcsEntrySecRwRtStHdrstUpwdPos_Val
  PA_KeSMSw6sAcsEntrySecRwRtStLgrstUpwdPosMax_Val : Constant  Value=KeSMSw6sAcsEntrySecRwRtStLgrstUpwdPosMax_Val
  PA_KeSMSw6sAcsEntrySecRwRtStLgrstUpwdPosMin_Val : Constant  Value=KeSMSw6sAcsEntrySecRwRtStLgrstUpwdPosMin_Val
  PA_KeSMSw6sAcsEntrySecRwRtStLgrstUpwdPos_Val : Constant  Value=KeSMSw6sAcsEntrySecRwRtStLgrstUpwdPos_Val
  PA_KeSMSw6sAcsEntrySecRwRtStLtwdRtwdPosMax_Val : Constant  Value=KeSMSw6sAcsEntrySecRwRtStLtwdRtwdPosMax_Val
  PA_KeSMSw6sAcsEntrySecRwRtStLtwdRtwdPosMin_Val : Constant  Value=KeSMSw6sAcsEntrySecRwRtStLtwdRtwdPosMin_Val
  PA_KeSMSw6sAcsEntrySecRwRtStLtwdRtwdPos_Val : Constant  Value=KeSMSw6sAcsEntrySecRwRtStLtwdRtwdPos_Val
  PA_KeSMSw6sAcsEntryThdRwLtStBkReclnUpwdDnwdPosMax_Val : Constant  Value=KeSMSw6sAcsEntryThdRwLtStBkReclnUpwdDnwdPosMax_Val
  PA_KeSMSw6sAcsEntryThdRwLtStBkReclnUpwdDnwdPosMin_Val : Constant  Value=KeSMSw6sAcsEntryThdRwLtStBkReclnUpwdDnwdPosMin_Val
  PA_KeSMSw6sAcsEntryThdRwLtStBkReclnUpwdDnwdPos_Val : Constant  Value=KeSMSw6sAcsEntryThdRwLtStBkReclnUpwdDnwdPos_Val
  PA_KeSMSw6sAcsEntryThdRwLtStCshnFldUpwdDnwdPosMax_Val : Constant  Value=KeSMSw6sAcsEntryThdRwLtStCshnFldUpwdDnwdPosMax_Val
  PA_KeSMSw6sAcsEntryThdRwLtStCshnFldUpwdDnwdPosMin_Val : Constant  Value=KeSMSw6sAcsEntryThdRwLtStCshnFldUpwdDnwdPosMin_Val
  PA_KeSMSw6sAcsEntryThdRwLtStCshnFldUpwdDnwdPos_Val : Constant  Value=KeSMSw6sAcsEntryThdRwLtStCshnFldUpwdDnwdPos_Val
  PA_KeSMSw6sAcsEntryThdRwLtStFrwdBkwdPosMax_Val : Constant  Value=KeSMSw6sAcsEntryThdRwLtStFrwdBkwdPosMax_Val
  PA_KeSMSw6sAcsEntryThdRwLtStFrwdBkwdPosMin_Val : Constant  Value=KeSMSw6sAcsEntryThdRwLtStFrwdBkwdPosMin_Val
  PA_KeSMSw6sAcsEntryThdRwLtStFrwdBkwdPos_Val : Constant  Value=KeSMSw6sAcsEntryThdRwLtStFrwdBkwdPos_Val
  PA_KeSMSw6sAcsEntryThdRwRtStBkReclnUpwdDnwdPosMax_Val : Constant  Value=KeSMSw6sAcsEntryThdRwRtStBkReclnUpwdDnwdPosMax_Val
  PA_KeSMSw6sAcsEntryThdRwRtStBkReclnUpwdDnwdPosMin_Val : Constant  Value=KeSMSw6sAcsEntryThdRwRtStBkReclnUpwdDnwdPosMin_Val
  PA_KeSMSw6sAcsEntryThdRwRtStBkReclnUpwdDnwdPos_Val : Constant  Value=KeSMSw6sAcsEntryThdRwRtStBkReclnUpwdDnwdPos_Val
  PA_KeSMSw6sAcsEntryThdRwRtStCshnFldUpwdDnwdPosMax_Val : Constant  Value=KeSMSw6sAcsEntryThdRwRtStCshnFldUpwdDnwdPosMax_Val
  PA_KeSMSw6sAcsEntryThdRwRtStCshnFldUpwdDnwdPosMin_Val : Constant  Value=KeSMSw6sAcsEntryThdRwRtStCshnFldUpwdDnwdPosMin_Val
  PA_KeSMSw6sAcsEntryThdRwRtStCshnFldUpwdDnwdPos_Val : Constant  Value=KeSMSw6sAcsEntryThdRwRtStCshnFldUpwdDnwdPos_Val
  PA_KeSMSw6sAcsEntryThdRwRtStFrwdBkwdPosMax_Val : Constant  Value=KeSMSw6sAcsEntryThdRwRtStFrwdBkwdPosMax_Val
  PA_KeSMSw6sAcsEntryThdRwRtStFrwdBkwdPosMin_Val : Constant  Value=KeSMSw6sAcsEntryThdRwRtStFrwdBkwdPosMin_Val
  PA_KeSMSw6sAcsEntryThdRwRtStFrwdBkwdPos_Val : Constant  Value=KeSMSw6sAcsEntryThdRwRtStFrwdBkwdPos_Val
  PA_KeSMSw6sAcsExtDrvStBkReclnUpwdDnwdPosMax_Val : Constant  Value=KeSMSw6sAcsExtDrvStBkReclnUpwdDnwdPosMax_Val
  PA_KeSMSw6sAcsExtDrvStBkReclnUpwdDnwdPosMin_Val : Constant  Value=KeSMSw6sAcsExtDrvStBkReclnUpwdDnwdPosMin_Val
  PA_KeSMSw6sAcsExtDrvStBkReclnUpwdDnwdPos_Val : Constant  Value=KeSMSw6sAcsExtDrvStBkReclnUpwdDnwdPos_Val
  PA_KeSMSw6sAcsExtDrvStFrwdBkwdPosMax_Val : Constant  Value=KeSMSw6sAcsExtDrvStFrwdBkwdPosMax_Val
  PA_KeSMSw6sAcsExtDrvStFrwdBkwdPosMin_Val : Constant  Value=KeSMSw6sAcsExtDrvStFrwdBkwdPosMin_Val
  PA_KeSMSw6sAcsExtDrvStFrwdBkwdPos_Val : Constant  Value=KeSMSw6sAcsExtDrvStFrwdBkwdPos_Val
  PA_KeSMSw6sAcsExtDrvStFtUpwdDnwdPosMax_Val : Constant  Value=KeSMSw6sAcsExtDrvStFtUpwdDnwdPosMax_Val
  PA_KeSMSw6sAcsExtDrvStFtUpwdDnwdPosMin_Val : Constant  Value=KeSMSw6sAcsExtDrvStFtUpwdDnwdPosMin_Val
  PA_KeSMSw6sAcsExtDrvStFtUpwdDnwdPos_Val : Constant  Value=KeSMSw6sAcsExtDrvStFtUpwdDnwdPos_Val
  PA_KeSMSw6sAcsExtPassStBkReclnUpwdDnwdPosMax_Val : Constant  Value=KeSMSw6sAcsExtPassStBkReclnUpwdDnwdPosMax_Val
  PA_KeSMSw6sAcsExtPassStBkReclnUpwdDnwdPosMin_Val : Constant  Value=KeSMSw6sAcsExtPassStBkReclnUpwdDnwdPosMin_Val
  PA_KeSMSw6sAcsExtPassStBkReclnUpwdDnwdPos_Val : Constant  Value=KeSMSw6sAcsExtPassStBkReclnUpwdDnwdPos_Val
  PA_KeSMSw6sAcsExtPassStFrwdBkwdPosMax_Val : Constant  Value=KeSMSw6sAcsExtPassStFrwdBkwdPosMax_Val
  PA_KeSMSw6sAcsExtPassStFrwdBkwdPosMin_Val : Constant  Value=KeSMSw6sAcsExtPassStFrwdBkwdPosMin_Val
  PA_KeSMSw6sAcsExtPassStFrwdBkwdPos_Val : Constant  Value=KeSMSw6sAcsExtPassStFrwdBkwdPos_Val
  PA_KeSMSw6sAcsExtPassStFtUpwdDnwdPosMax_Val : Constant  Value=KeSMSw6sAcsExtPassStFtUpwdDnwdPosMax_Val
  PA_KeSMSw6sAcsExtPassStFtUpwdDnwdPosMin_Val : Constant  Value=KeSMSw6sAcsExtPassStFtUpwdDnwdPosMin_Val
  PA_KeSMSw6sAcsExtPassStFtUpwdDnwdPos_Val : Constant  Value=KeSMSw6sAcsExtPassStFtUpwdDnwdPos_Val
  PA_KeSMSw6sAcsExtSecRwLtStArmScrnPosMax_Val : Constant  Value=KeSMSw6sAcsExtSecRwLtStArmScrnPosMax_Val
  PA_KeSMSw6sAcsExtSecRwLtStArmScrnPosMin_Val : Constant  Value=KeSMSw6sAcsExtSecRwLtStArmScrnPosMin_Val
  PA_KeSMSw6sAcsExtSecRwLtStArmScrnPos_Val : Constant  Value=KeSMSw6sAcsExtSecRwLtStArmScrnPos_Val
  PA_KeSMSw6sAcsExtSecRwLtStBkReclnUpwdDnwdPosMax_Val : Constant  Value=KeSMSw6sAcsExtSecRwLtStBkReclnUpwdDnwdPosMax_Val
  PA_KeSMSw6sAcsExtSecRwLtStBkReclnUpwdDnwdPosMin_Val : Constant  Value=KeSMSw6sAcsExtSecRwLtStBkReclnUpwdDnwdPosMin_Val
  PA_KeSMSw6sAcsExtSecRwLtStBkReclnUpwdDnwdPos_Val : Constant  Value=KeSMSw6sAcsExtSecRwLtStBkReclnUpwdDnwdPos_Val
  PA_KeSMSw6sAcsExtSecRwLtStFrwdBkwdPosMax_Val : Constant  Value=KeSMSw6sAcsExtSecRwLtStFrwdBkwdPosMax_Val
  PA_KeSMSw6sAcsExtSecRwLtStFrwdBkwdPosMin_Val : Constant  Value=KeSMSw6sAcsExtSecRwLtStFrwdBkwdPosMin_Val
  PA_KeSMSw6sAcsExtSecRwLtStFrwdBkwdPos_Val : Constant  Value=KeSMSw6sAcsExtSecRwLtStFrwdBkwdPos_Val
  PA_KeSMSw6sAcsExtSecRwLtStLgrstUpwdDnwdPosMax_Val : Constant  Value=KeSMSw6sAcsExtSecRwLtStLgrstUpwdDnwdPosMax_Val
  PA_KeSMSw6sAcsExtSecRwLtStLgrstUpwdDnwdPosMin_Val : Constant  Value=KeSMSw6sAcsExtSecRwLtStLgrstUpwdDnwdPosMin_Val
  PA_KeSMSw6sAcsExtSecRwLtStLgrstUpwdDnwdPos_Val : Constant  Value=KeSMSw6sAcsExtSecRwLtStLgrstUpwdDnwdPos_Val
  PA_KeSMSw6sAcsExtSecRwLtStLtwdRtwdPosMax_Val : Constant  Value=KeSMSw6sAcsExtSecRwLtStLtwdRtwdPosMax_Val
  PA_KeSMSw6sAcsExtSecRwLtStLtwdRtwdPosMin_Val : Constant  Value=KeSMSw6sAcsExtSecRwLtStLtwdRtwdPosMin_Val
  PA_KeSMSw6sAcsExtSecRwLtStLtwdRtwdPos_Val : Constant  Value=KeSMSw6sAcsExtSecRwLtStLtwdRtwdPos_Val
  PA_KeSMSw6sAcsExtSecRwRtStArmScrnPosMax_Val : Constant  Value=KeSMSw6sAcsExtSecRwRtStArmScrnPosMax_Val
  PA_KeSMSw6sAcsExtSecRwRtStArmScrnPosMin_Val : Constant  Value=KeSMSw6sAcsExtSecRwRtStArmScrnPosMin_Val
  PA_KeSMSw6sAcsExtSecRwRtStArmScrnPos_Val : Constant  Value=KeSMSw6sAcsExtSecRwRtStArmScrnPos_Val
  PA_KeSMSw6sAcsExtSecRwRtStBkReclnUpwdDnwdPosMax_Val : Constant  Value=KeSMSw6sAcsExtSecRwRtStBkReclnUpwdDnwdPosMax_Val
  PA_KeSMSw6sAcsExtSecRwRtStBkReclnUpwdDnwdPosMin_Val : Constant  Value=KeSMSw6sAcsExtSecRwRtStBkReclnUpwdDnwdPosMin_Val
  PA_KeSMSw6sAcsExtSecRwRtStBkReclnUpwdDnwdPos_Val : Constant  Value=KeSMSw6sAcsExtSecRwRtStBkReclnUpwdDnwdPos_Val
  PA_KeSMSw6sAcsExtSecRwRtStFrwdBkwdPosMax_Val : Constant  Value=KeSMSw6sAcsExtSecRwRtStFrwdBkwdPosMax_Val
  PA_KeSMSw6sAcsExtSecRwRtStFrwdBkwdPosMin_Val : Constant  Value=KeSMSw6sAcsExtSecRwRtStFrwdBkwdPosMin_Val
  PA_KeSMSw6sAcsExtSecRwRtStFrwdBkwdPos_Val : Constant  Value=KeSMSw6sAcsExtSecRwRtStFrwdBkwdPos_Val
  PA_KeSMSw6sAcsExtSecRwRtStLgrstUpwdDnwdPosMax_Val : Constant  Value=KeSMSw6sAcsExtSecRwRtStLgrstUpwdDnwdPosMax_Val
  PA_KeSMSw6sAcsExtSecRwRtStLgrstUpwdDnwdPosMin_Val : Constant  Value=KeSMSw6sAcsExtSecRwRtStLgrstUpwdDnwdPosMin_Val
  PA_KeSMSw6sAcsExtSecRwRtStLgrstUpwdDnwdPos_Val : Constant  Value=KeSMSw6sAcsExtSecRwRtStLgrstUpwdDnwdPos_Val
  PA_KeSMSw6sAcsExtSecRwRtStLtwdRtwdPosMax_Val : Constant  Value=KeSMSw6sAcsExtSecRwRtStLtwdRtwdPosMax_Val
  PA_KeSMSw6sAcsExtSecRwRtStLtwdRtwdPosMin_Val : Constant  Value=KeSMSw6sAcsExtSecRwRtStLtwdRtwdPosMin_Val
  PA_KeSMSw6sAcsExtSecRwRtStLtwdRtwdPos_Val : Constant  Value=KeSMSw6sAcsExtSecRwRtStLtwdRtwdPos_Val
  PA_KeSMSw6sAcsExtThdRwLtStBkReclnUpwdDnwdPosMax_Val : Constant  Value=KeSMSw6sAcsExtThdRwLtStBkReclnUpwdDnwdPosMax_Val
  PA_KeSMSw6sAcsExtThdRwLtStBkReclnUpwdDnwdPosMin_Val : Constant  Value=KeSMSw6sAcsExtThdRwLtStBkReclnUpwdDnwdPosMin_Val
  PA_KeSMSw6sAcsExtThdRwLtStBkReclnUpwdDnwdPos_Val : Constant  Value=KeSMSw6sAcsExtThdRwLtStBkReclnUpwdDnwdPos_Val
  PA_KeSMSw6sAcsExtThdRwLtStCshnFldUpwdDnwdPosMax_Val : Constant  Value=KeSMSw6sAcsExtThdRwLtStCshnFldUpwdDnwdPosMax_Val
  PA_KeSMSw6sAcsExtThdRwLtStCshnFldUpwdDnwdPosMin_Val : Constant  Value=KeSMSw6sAcsExtThdRwLtStCshnFldUpwdDnwdPosMin_Val
  PA_KeSMSw6sAcsExtThdRwLtStCshnFldUpwdDnwdPos_Val : Constant  Value=KeSMSw6sAcsExtThdRwLtStCshnFldUpwdDnwdPos_Val
  PA_KeSMSw6sAcsExtThdRwLtStFrwdBkwdPosMax_Val : Constant  Value=KeSMSw6sAcsExtThdRwLtStFrwdBkwdPosMax_Val
  PA_KeSMSw6sAcsExtThdRwLtStFrwdBkwdPosMin_Val : Constant  Value=KeSMSw6sAcsExtThdRwLtStFrwdBkwdPosMin_Val
  PA_KeSMSw6sAcsExtThdRwLtStFrwdBkwdPos_Val : Constant  Value=KeSMSw6sAcsExtThdRwLtStFrwdBkwdPos_Val
  PA_KeSMSw6sAcsExtThdRwRtStBkReclnUpwdDnwdPosMax_Val : Constant  Value=KeSMSw6sAcsExtThdRwRtStBkReclnUpwdDnwdPosMax_Val
  PA_KeSMSw6sAcsExtThdRwRtStBkReclnUpwdDnwdPosMin_Val : Constant  Value=KeSMSw6sAcsExtThdRwRtStBkReclnUpwdDnwdPosMin_Val
  PA_KeSMSw6sAcsExtThdRwRtStBkReclnUpwdDnwdPos_Val : Constant  Value=KeSMSw6sAcsExtThdRwRtStBkReclnUpwdDnwdPos_Val
  PA_KeSMSw6sAcsExtThdRwRtStCshnFldUpwdDnwdPosMax_Val : Constant  Value=KeSMSw6sAcsExtThdRwRtStCshnFldUpwdDnwdPosMax_Val
  PA_KeSMSw6sAcsExtThdRwRtStCshnFldUpwdDnwdPosMin_Val : Constant  Value=KeSMSw6sAcsExtThdRwRtStCshnFldUpwdDnwdPosMin_Val
  PA_KeSMSw6sAcsExtThdRwRtStCshnFldUpwdDnwdPos_Val : Constant  Value=KeSMSw6sAcsExtThdRwRtStCshnFldUpwdDnwdPos_Val
  PA_KeSMSw6sAcsExtThdRwRtStFrwdBkwdPosMax_Val : Constant  Value=KeSMSw6sAcsExtThdRwRtStFrwdBkwdPosMax_Val
  PA_KeSMSw6sAcsExtThdRwRtStFrwdBkwdPosMin_Val : Constant  Value=KeSMSw6sAcsExtThdRwRtStFrwdBkwdPosMin_Val
  PA_KeSMSw6sAcsExtThdRwRtStFrwdBkwdPos_Val : Constant  Value=KeSMSw6sAcsExtThdRwRtStFrwdBkwdPos_Val
  PA_KeSMSw6sFamilyLMdThdRwLtStFrwdBkwdPosMax_Val : Constant  Value=KeSMSw6sFamilyLMdThdRwLtStFrwdBkwdPosMax_Val
  PA_KeSMSw6sFamilyLMdThdRwLtStFrwdBkwdPosMin_Val : Constant  Value=KeSMSw6sFamilyLMdThdRwLtStFrwdBkwdPosMin_Val
  PA_KeSMSw6sFamilyLMdThdRwLtStFrwdBkwdPos_Val : Constant  Value=KeSMSw6sFamilyLMdThdRwLtStFrwdBkwdPos_Val
  PA_KeSMSw6sFamilyMdSecRwLtStFrwdBkwdPosMax_Val : Constant  Value=KeSMSw6sFamilyMdSecRwLtStFrwdBkwdPosMax_Val
  PA_KeSMSw6sFamilyMdSecRwLtStFrwdBkwdPosMin_Val : Constant  Value=KeSMSw6sFamilyMdSecRwLtStFrwdBkwdPosMin_Val
  PA_KeSMSw6sFamilyMdSecRwLtStFrwdBkwdPos_Val : Constant  Value=KeSMSw6sFamilyMdSecRwLtStFrwdBkwdPos_Val
  PA_KeSMSw6sFamilyMdSecRwLtStLtwdRtwdPosMax_Val : Constant  Value=KeSMSw6sFamilyMdSecRwLtStLtwdRtwdPosMax_Val
  PA_KeSMSw6sFamilyMdSecRwLtStLtwdRtwdPosMin_Val : Constant  Value=KeSMSw6sFamilyMdSecRwLtStLtwdRtwdPosMin_Val
  PA_KeSMSw6sFamilyMdSecRwLtStLtwdRtwdPos_Val : Constant  Value=KeSMSw6sFamilyMdSecRwLtStLtwdRtwdPos_Val
  PA_KeSMSw6sFamilyMdSecRwRtStFrwdBkwdPosMax_Val : Constant  Value=KeSMSw6sFamilyMdSecRwRtStFrwdBkwdPosMax_Val
  PA_KeSMSw6sFamilyMdSecRwRtStFrwdBkwdPosMin_Val : Constant  Value=KeSMSw6sFamilyMdSecRwRtStFrwdBkwdPosMin_Val
  PA_KeSMSw6sFamilyMdSecRwRtStFrwdBkwdPos_Val : Constant  Value=KeSMSw6sFamilyMdSecRwRtStFrwdBkwdPos_Val
  PA_KeSMSw6sFamilyMdSecRwRtStLtwdRtwdPosMax_Val : Constant  Value=KeSMSw6sFamilyMdSecRwRtStLtwdRtwdPosMax_Val
  PA_KeSMSw6sFamilyMdSecRwRtStLtwdRtwdPosMin_Val : Constant  Value=KeSMSw6sFamilyMdSecRwRtStLtwdRtwdPosMin_Val
  PA_KeSMSw6sFamilyMdSecRwRtStLtwdRtwdPos_Val : Constant  Value=KeSMSw6sFamilyMdSecRwRtStLtwdRtwdPos_Val
  PA_KeSMSw6sFamilyMdThdRwLtStFrwdBkwdPosMax_Val : Constant  Value=KeSMSw6sFamilyMdThdRwLtStFrwdBkwdPosMax_Val
  PA_KeSMSw6sFamilyMdThdRwLtStFrwdBkwdPosMin_Val : Constant  Value=KeSMSw6sFamilyMdThdRwLtStFrwdBkwdPosMin_Val
  PA_KeSMSw6sFamilyMdThdRwLtStFrwdBkwdPos_Val : Constant  Value=KeSMSw6sFamilyMdThdRwLtStFrwdBkwdPos_Val
  PA_KeSMSw6sFamilyMdThdRwRtStFrwdBkwdPosMax_Val : Constant  Value=KeSMSw6sFamilyMdThdRwRtStFrwdBkwdPosMax_Val
  PA_KeSMSw6sFamilyMdThdRwRtStFrwdBkwdPosMin_Val : Constant  Value=KeSMSw6sFamilyMdThdRwRtStFrwdBkwdPosMin_Val
  PA_KeSMSw6sFamilyMdThdRwRtStFrwdBkwdPos_Val : Constant  Value=KeSMSw6sFamilyMdThdRwRtStFrwdBkwdPos_Val
  PA_KeSMSw6sFamilyRMdSecRwLtStFrwdBkwdPosMax_Val : Constant  Value=KeSMSw6sFamilyRMdSecRwLtStFrwdBkwdPosMax_Val
  PA_KeSMSw6sFamilyRMdSecRwLtStFrwdBkwdPosMin_Val : Constant  Value=KeSMSw6sFamilyRMdSecRwLtStFrwdBkwdPosMin_Val
  PA_KeSMSw6sFamilyRMdSecRwLtStFrwdBkwdPos_Val : Constant  Value=KeSMSw6sFamilyRMdSecRwLtStFrwdBkwdPos_Val
  PA_KeSMSw6sFamilyRMdSecRwLtStLtwdRtwdPosMax_Val : Constant  Value=KeSMSw6sFamilyRMdSecRwLtStLtwdRtwdPosMax_Val
  PA_KeSMSw6sFamilyRMdSecRwLtStLtwdRtwdPosMin_Val : Constant  Value=KeSMSw6sFamilyRMdSecRwLtStLtwdRtwdPosMin_Val
  PA_KeSMSw6sFamilyRMdSecRwLtStLtwdRtwdPos_Val : Constant  Value=KeSMSw6sFamilyRMdSecRwLtStLtwdRtwdPos_Val
  PA_KeSMSw6sFamilyRMdSecRwRtStFrwdBkwdPosMax_Val : Constant  Value=KeSMSw6sFamilyRMdSecRwRtStFrwdBkwdPosMax_Val
  PA_KeSMSw6sFamilyRMdSecRwRtStFrwdBkwdPosMin_Val : Constant  Value=KeSMSw6sFamilyRMdSecRwRtStFrwdBkwdPosMin_Val
  PA_KeSMSw6sFamilyRMdSecRwRtStFrwdBkwdPos_Val : Constant  Value=KeSMSw6sFamilyRMdSecRwRtStFrwdBkwdPos_Val
  PA_KeSMSw6sFamilyRMdSecRwRtStLtwdRtwdPosMax_Val : Constant  Value=KeSMSw6sFamilyRMdSecRwRtStLtwdRtwdPosMax_Val
  PA_KeSMSw6sFamilyRMdSecRwRtStLtwdRtwdPosMin_Val : Constant  Value=KeSMSw6sFamilyRMdSecRwRtStLtwdRtwdPosMin_Val
  PA_KeSMSw6sFamilyRMdSecRwRtStLtwdRtwdPos_Val : Constant  Value=KeSMSw6sFamilyRMdSecRwRtStLtwdRtwdPos_Val
  PA_KeSMSw6sFamilyRMdThdRwRtStFrwdBkwdPosMax_Val : Constant  Value=KeSMSw6sFamilyRMdThdRwRtStFrwdBkwdPosMax_Val
  PA_KeSMSw6sFamilyRMdThdRwRtStFrwdBkwdPosMin_Val : Constant  Value=KeSMSw6sFamilyRMdThdRwRtStFrwdBkwdPosMin_Val
  PA_KeSMSw6sFamilyRMdThdRwRtStFrwdBkwdPos_Val : Constant  Value=KeSMSw6sFamilyRMdThdRwRtStFrwdBkwdPos_Val
  PA_KeSMSw6sIntimacyMdSecRwLtStLtwdRtwdPosMax_Val : Constant  Value=KeSMSw6sIntimacyMdSecRwLtStLtwdRtwdPosMax_Val
  PA_KeSMSw6sIntimacyMdSecRwLtStLtwdRtwdPosMin_Val : Constant  Value=KeSMSw6sIntimacyMdSecRwLtStLtwdRtwdPosMin_Val
  PA_KeSMSw6sIntimacyMdSecRwLtStLtwdRtwdPos_Val : Constant  Value=KeSMSw6sIntimacyMdSecRwLtStLtwdRtwdPos_Val
  PA_KeSMSw6sIntimacyMdSecRwRtStLtwdRtwdPosMax_Val : Constant  Value=KeSMSw6sIntimacyMdSecRwRtStLtwdRtwdPosMax_Val
  PA_KeSMSw6sIntimacyMdSecRwRtStLtwdRtwdPosMin_Val : Constant  Value=KeSMSw6sIntimacyMdSecRwRtStLtwdRtwdPosMin_Val
  PA_KeSMSw6sIntimacyMdSecRwRtStLtwdRtwdPos_Val : Constant  Value=KeSMSw6sIntimacyMdSecRwRtStLtwdRtwdPos_Val
  PA_KeSMSw6sIntimacyRMdSecRwLtStLtwdRtwdPosMax_Val : Constant  Value=KeSMSw6sIntimacyRMdSecRwLtStLtwdRtwdPosMax_Val
  PA_KeSMSw6sIntimacyRMdSecRwLtStLtwdRtwdPosMin_Val : Constant  Value=KeSMSw6sIntimacyRMdSecRwLtStLtwdRtwdPosMin_Val
  PA_KeSMSw6sIntimacyRMdSecRwLtStLtwdRtwdPos_Val : Constant  Value=KeSMSw6sIntimacyRMdSecRwLtStLtwdRtwdPos_Val
  PA_KeSMSw6sIntimacyRMdSecRwRtStLtwdRtwdPosMax_Val : Constant  Value=KeSMSw6sIntimacyRMdSecRwRtStLtwdRtwdPosMax_Val
  PA_KeSMSw6sIntimacyRMdSecRwRtStLtwdRtwdPosMin_Val : Constant  Value=KeSMSw6sIntimacyRMdSecRwRtStLtwdRtwdPosMin_Val
  PA_KeSMSw6sIntimacyRMdSecRwRtStLtwdRtwdPos_Val : Constant  Value=KeSMSw6sIntimacyRMdSecRwRtStLtwdRtwdPos_Val
  PA_KeSMSw6sLugThdRwLtStBkReclnUpwdDnwdPosMax_Val : Constant  Value=KeSMSw6sLugThdRwLtStBkReclnUpwdDnwdPosMax_Val
  PA_KeSMSw6sLugThdRwLtStBkReclnUpwdDnwdPosMin_Val : Constant  Value=KeSMSw6sLugThdRwLtStBkReclnUpwdDnwdPosMin_Val
  PA_KeSMSw6sLugThdRwLtStBkReclnUpwdDnwdPos_Val : Constant  Value=KeSMSw6sLugThdRwLtStBkReclnUpwdDnwdPos_Val
  PA_KeSMSw6sLugThdRwLtStCshnFldUpwdDnwdPosMax_Val : Constant  Value=KeSMSw6sLugThdRwLtStCshnFldUpwdDnwdPosMax_Val
  PA_KeSMSw6sLugThdRwLtStCshnFldUpwdDnwdPosMin_Val : Constant  Value=KeSMSw6sLugThdRwLtStCshnFldUpwdDnwdPosMin_Val
  PA_KeSMSw6sLugThdRwLtStCshnFldUpwdDnwdPos_Val : Constant  Value=KeSMSw6sLugThdRwLtStCshnFldUpwdDnwdPos_Val
  PA_KeSMSw6sLugThdRwLtStFrwdBkwdPosMax_Val : Constant  Value=KeSMSw6sLugThdRwLtStFrwdBkwdPosMax_Val
  PA_KeSMSw6sLugThdRwLtStFrwdBkwdPosMin_Val : Constant  Value=KeSMSw6sLugThdRwLtStFrwdBkwdPosMin_Val
  PA_KeSMSw6sLugThdRwLtStFrwdBkwdPos_Val : Constant  Value=KeSMSw6sLugThdRwLtStFrwdBkwdPos_Val
  PA_KeSMSw6sLugThdRwRtStBkReclnUpwdDnwdPosMax_Val : Constant  Value=KeSMSw6sLugThdRwRtStBkReclnUpwdDnwdPosMax_Val
  PA_KeSMSw6sLugThdRwRtStBkReclnUpwdDnwdPosMin_Val : Constant  Value=KeSMSw6sLugThdRwRtStBkReclnUpwdDnwdPosMin_Val
  PA_KeSMSw6sLugThdRwRtStBkReclnUpwdDnwdPos_Val : Constant  Value=KeSMSw6sLugThdRwRtStBkReclnUpwdDnwdPos_Val
  PA_KeSMSw6sLugThdRwRtStCshnFldUpwdDnwdPosMax_Val : Constant  Value=KeSMSw6sLugThdRwRtStCshnFldUpwdDnwdPosMax_Val
  PA_KeSMSw6sLugThdRwRtStCshnFldUpwdDnwdPosMin_Val : Constant  Value=KeSMSw6sLugThdRwRtStCshnFldUpwdDnwdPosMin_Val
  PA_KeSMSw6sLugThdRwRtStCshnFldUpwdDnwdPos_Val : Constant  Value=KeSMSw6sLugThdRwRtStCshnFldUpwdDnwdPos_Val
  PA_KeSMSw6sLugThdRwRtStFrwdBkwdPosMax_Val : Constant  Value=KeSMSw6sLugThdRwRtStFrwdBkwdPosMax_Val
  PA_KeSMSw6sLugThdRwRtStFrwdBkwdPosMin_Val : Constant  Value=KeSMSw6sLugThdRwRtStFrwdBkwdPosMin_Val
  PA_KeSMSw6sLugThdRwRtStFrwdBkwdPos_Val : Constant  Value=KeSMSw6sLugThdRwRtStFrwdBkwdPos_Val
  PA_KeSMSw6sRecoveryDrvStFtUpwdDnwdPosMax_Val : Constant  Value=KeSMSw6sRecoveryDrvStFtUpwdDnwdPosMax_Val
  PA_KeSMSw6sRecoveryDrvStFtUpwdDnwdPosMin_Val : Constant  Value=KeSMSw6sRecoveryDrvStFtUpwdDnwdPosMin_Val
  PA_KeSMSw6sRecoveryDrvStFtUpwdDnwdPos_Val : Constant  Value=KeSMSw6sRecoveryDrvStFtUpwdDnwdPos_Val
  PA_KeSMSw6sRecoveryMdSecRwLtStArmScrnPosMax_Val : Constant  Value=KeSMSw6sRecoveryMdSecRwLtStArmScrnPosMax_Val
  PA_KeSMSw6sRecoveryMdSecRwLtStArmScrnPosMin_Val : Constant  Value=KeSMSw6sRecoveryMdSecRwLtStArmScrnPosMin_Val
  PA_KeSMSw6sRecoveryMdSecRwLtStArmScrnPos_Val : Constant  Value=KeSMSw6sRecoveryMdSecRwLtStArmScrnPos_Val
  PA_KeSMSw6sRecoveryMdSecRwLtStBkReclnUpwdDnwdPosMax_Val : Constant  Value=KeSMSw6sRecoveryMdSecRwLtStBkReclnUpwdDnwdPosMax_Val
  PA_KeSMSw6sRecoveryMdSecRwLtStBkReclnUpwdDnwdPosMin_Val : Constant  Value=KeSMSw6sRecoveryMdSecRwLtStBkReclnUpwdDnwdPosMin_Val
  PA_KeSMSw6sRecoveryMdSecRwLtStBkReclnUpwdDnwdPos_Val : Constant  Value=KeSMSw6sRecoveryMdSecRwLtStBkReclnUpwdDnwdPos_Val
  PA_KeSMSw6sRecoveryMdSecRwLtStFrwdBkwdPosMax_Val : Constant  Value=KeSMSw6sRecoveryMdSecRwLtStFrwdBkwdPosMax_Val
  PA_KeSMSw6sRecoveryMdSecRwLtStFrwdBkwdPosMin_Val : Constant  Value=KeSMSw6sRecoveryMdSecRwLtStFrwdBkwdPosMin_Val
  PA_KeSMSw6sRecoveryMdSecRwLtStFrwdBkwdPos_Val : Constant  Value=KeSMSw6sRecoveryMdSecRwLtStFrwdBkwdPos_Val
  PA_KeSMSw6sRecoveryMdSecRwLtStHdrstUpwdDnwdPosMax_Val : Constant  Value=KeSMSw6sRecoveryMdSecRwLtStHdrstUpwdDnwdPosMax_Val
  PA_KeSMSw6sRecoveryMdSecRwLtStHdrstUpwdDnwdPosMin_Val : Constant  Value=KeSMSw6sRecoveryMdSecRwLtStHdrstUpwdDnwdPosMin_Val
  PA_KeSMSw6sRecoveryMdSecRwLtStHdrstUpwdDnwdPos_Val : Constant  Value=KeSMSw6sRecoveryMdSecRwLtStHdrstUpwdDnwdPos_Val
  PA_KeSMSw6sRecoveryMdSecRwLtStLgrstUpwdDnwdPosMax_Val : Constant  Value=KeSMSw6sRecoveryMdSecRwLtStLgrstUpwdDnwdPosMax_Val
  PA_KeSMSw6sRecoveryMdSecRwLtStLgrstUpwdDnwdPosMin_Val : Constant  Value=KeSMSw6sRecoveryMdSecRwLtStLgrstUpwdDnwdPosMin_Val
  PA_KeSMSw6sRecoveryMdSecRwLtStLgrstUpwdDnwdPos_Val : Constant  Value=KeSMSw6sRecoveryMdSecRwLtStLgrstUpwdDnwdPos_Val
  PA_KeSMSw6sRecoveryMdSecRwLtStLtwdRtwdPosMax_Val : Constant  Value=KeSMSw6sRecoveryMdSecRwLtStLtwdRtwdPosMax_Val
  PA_KeSMSw6sRecoveryMdSecRwLtStLtwdRtwdPosMin_Val : Constant  Value=KeSMSw6sRecoveryMdSecRwLtStLtwdRtwdPosMin_Val
  PA_KeSMSw6sRecoveryMdSecRwLtStLtwdRtwdPos_Val : Constant  Value=KeSMSw6sRecoveryMdSecRwLtStLtwdRtwdPos_Val
  PA_KeSMSw6sRecoveryMdSecRwRtStArmScrnPosMax_Val : Constant  Value=KeSMSw6sRecoveryMdSecRwRtStArmScrnPosMax_Val
  PA_KeSMSw6sRecoveryMdSecRwRtStArmScrnPosMin_Val : Constant  Value=KeSMSw6sRecoveryMdSecRwRtStArmScrnPosMin_Val
  PA_KeSMSw6sRecoveryMdSecRwRtStArmScrnPos_Val : Constant  Value=KeSMSw6sRecoveryMdSecRwRtStArmScrnPos_Val
  PA_KeSMSw6sRecoveryMdSecRwRtStBkReclnUpwdDnwdPosMax_Val : Constant  Value=KeSMSw6sRecoveryMdSecRwRtStBkReclnUpwdDnwdPosMax_Val
  PA_KeSMSw6sRecoveryMdSecRwRtStBkReclnUpwdDnwdPosMin_Val : Constant  Value=KeSMSw6sRecoveryMdSecRwRtStBkReclnUpwdDnwdPosMin_Val
  PA_KeSMSw6sRecoveryMdSecRwRtStBkReclnUpwdDnwdPos_Val : Constant  Value=KeSMSw6sRecoveryMdSecRwRtStBkReclnUpwdDnwdPos_Val
  PA_KeSMSw6sRecoveryMdSecRwRtStFrwdBkwdPosMax_Val : Constant  Value=KeSMSw6sRecoveryMdSecRwRtStFrwdBkwdPosMax_Val
  PA_KeSMSw6sRecoveryMdSecRwRtStFrwdBkwdPosMin_Val : Constant  Value=KeSMSw6sRecoveryMdSecRwRtStFrwdBkwdPosMin_Val
  PA_KeSMSw6sRecoveryMdSecRwRtStFrwdBkwdPos_Val : Constant  Value=KeSMSw6sRecoveryMdSecRwRtStFrwdBkwdPos_Val
  PA_KeSMSw6sRecoveryMdSecRwRtStHdrstUpwdDnwdPosMax_Val : Constant  Value=KeSMSw6sRecoveryMdSecRwRtStHdrstUpwdDnwdPosMax_Val
  PA_KeSMSw6sRecoveryMdSecRwRtStHdrstUpwdDnwdPosMin_Val : Constant  Value=KeSMSw6sRecoveryMdSecRwRtStHdrstUpwdDnwdPosMin_Val
  PA_KeSMSw6sRecoveryMdSecRwRtStHdrstUpwdDnwdPos_Val : Constant  Value=KeSMSw6sRecoveryMdSecRwRtStHdrstUpwdDnwdPos_Val
  PA_KeSMSw6sRecoveryMdSecRwRtStLgrstUpwdDnwdPosMax_Val : Constant  Value=KeSMSw6sRecoveryMdSecRwRtStLgrstUpwdDnwdPosMax_Val
  PA_KeSMSw6sRecoveryMdSecRwRtStLgrstUpwdDnwdPosMin_Val : Constant  Value=KeSMSw6sRecoveryMdSecRwRtStLgrstUpwdDnwdPosMin_Val
  PA_KeSMSw6sRecoveryMdSecRwRtStLgrstUpwdDnwdPos_Val : Constant  Value=KeSMSw6sRecoveryMdSecRwRtStLgrstUpwdDnwdPos_Val
  PA_KeSMSw6sRecoveryMdSecRwRtStLtwdRtwdPosMax_Val : Constant  Value=KeSMSw6sRecoveryMdSecRwRtStLtwdRtwdPosMax_Val
  PA_KeSMSw6sRecoveryMdSecRwRtStLtwdRtwdPosMin_Val : Constant  Value=KeSMSw6sRecoveryMdSecRwRtStLtwdRtwdPosMin_Val
  PA_KeSMSw6sRecoveryMdSecRwRtStLtwdRtwdPos_Val : Constant  Value=KeSMSw6sRecoveryMdSecRwRtStLtwdRtwdPos_Val
  PA_KeSMSw6sRecoveryPassStStFtUpwdDnwdPosMax_Val : Constant  Value=KeSMSw6sRecoveryPassStStFtUpwdDnwdPosMax_Val
  PA_KeSMSw6sRecoveryPassStStFtUpwdDnwdPosMin_Val : Constant  Value=KeSMSw6sRecoveryPassStStFtUpwdDnwdPosMin_Val
  PA_KeSMSw6sRecoveryPassStStFtUpwdDnwdPos_Val : Constant  Value=KeSMSw6sRecoveryPassStStFtUpwdDnwdPos_Val
  PA_KeSMSw6sVIPMDDrvStFtUpwdDnwdPosMax_Val : Constant  Value=KeSMSw6sVIPMDDrvStFtUpwdDnwdPosMax_Val
  PA_KeSMSw6sVIPMDDrvStFtUpwdDnwdPosMin_Val : Constant  Value=KeSMSw6sVIPMDDrvStFtUpwdDnwdPosMin_Val
  PA_KeSMSw6sVIPMDDrvStFtUpwdDnwdPos_Val : Constant  Value=KeSMSw6sVIPMDDrvStFtUpwdDnwdPos_Val
  PA_KeSMSw6sVIPMDPassStStFtUpwdDnwdPosMax_Val : Constant  Value=KeSMSw6sVIPMDPassStStFtUpwdDnwdPosMax_Val
  PA_KeSMSw6sVIPMDPassStStFtUpwdDnwdPosMin_Val : Constant  Value=KeSMSw6sVIPMDPassStStFtUpwdDnwdPosMin_Val
  PA_KeSMSw6sVIPMDPassStStFtUpwdDnwdPos_Val : Constant  Value=KeSMSw6sVIPMDPassStStFtUpwdDnwdPos_Val
  PA_KeSMSw6sVIPSecRwLtStArmScrnPosMax_Val : Constant  Value=KeSMSw6sVIPSecRwLtStArmScrnPosMax_Val
  PA_KeSMSw6sVIPSecRwLtStArmScrnPosMin_Val : Constant  Value=KeSMSw6sVIPSecRwLtStArmScrnPosMin_Val
  PA_KeSMSw6sVIPSecRwLtStArmScrnPos_Val : Constant  Value=KeSMSw6sVIPSecRwLtStArmScrnPos_Val
  PA_KeSMSw6sVIPSecRwLtStBkReclnUpwdDnwdPosMax_Val : Constant  Value=KeSMSw6sVIPSecRwLtStBkReclnUpwdDnwdPosMax_Val
  PA_KeSMSw6sVIPSecRwLtStBkReclnUpwdDnwdPosMin_Val : Constant  Value=KeSMSw6sVIPSecRwLtStBkReclnUpwdDnwdPosMin_Val
  PA_KeSMSw6sVIPSecRwLtStBkReclnUpwdDnwdPos_Val : Constant  Value=KeSMSw6sVIPSecRwLtStBkReclnUpwdDnwdPos_Val
  PA_KeSMSw6sVIPSecRwLtStFrwdBkwdPosMax_Val : Constant  Value=KeSMSw6sVIPSecRwLtStFrwdBkwdPosMax_Val
  PA_KeSMSw6sVIPSecRwLtStFrwdBkwdPosMin_Val : Constant  Value=KeSMSw6sVIPSecRwLtStFrwdBkwdPosMin_Val
  PA_KeSMSw6sVIPSecRwLtStFrwdBkwdPos_Val : Constant  Value=KeSMSw6sVIPSecRwLtStFrwdBkwdPos_Val
  PA_KeSMSw6sVIPSecRwLtStHdrstUpwdPosMax_Val : Constant  Value=KeSMSw6sVIPSecRwLtStHdrstUpwdPosMax_Val
  PA_KeSMSw6sVIPSecRwLtStHdrstUpwdPosMin_Val : Constant  Value=KeSMSw6sVIPSecRwLtStHdrstUpwdPosMin_Val
  PA_KeSMSw6sVIPSecRwLtStHdrstUpwdPos_Val : Constant  Value=KeSMSw6sVIPSecRwLtStHdrstUpwdPos_Val
  PA_KeSMSw6sVIPSecRwLtStLgrstUpwdPosMax_Val : Constant  Value=KeSMSw6sVIPSecRwLtStLgrstUpwdPosMax_Val
  PA_KeSMSw6sVIPSecRwLtStLgrstUpwdPosMin_Val : Constant  Value=KeSMSw6sVIPSecRwLtStLgrstUpwdPosMin_Val
  PA_KeSMSw6sVIPSecRwLtStLgrstUpwdPos_Val : Constant  Value=KeSMSw6sVIPSecRwLtStLgrstUpwdPos_Val
  PA_KeSMSw6sVIPSecRwLtStLtwdRtwdPosMax_Val : Constant  Value=KeSMSw6sVIPSecRwLtStLtwdRtwdPosMax_Val
  PA_KeSMSw6sVIPSecRwLtStLtwdRtwdPosMin_Val : Constant  Value=KeSMSw6sVIPSecRwLtStLtwdRtwdPosMin_Val
  PA_KeSMSw6sVIPSecRwLtStLtwdRtwdPos_Val : Constant  Value=KeSMSw6sVIPSecRwLtStLtwdRtwdPos_Val
  PA_KeSMSw6sVIPSecRwRtStArmScrnPosMax_Val : Constant  Value=KeSMSw6sVIPSecRwRtStArmScrnPosMax_Val
  PA_KeSMSw6sVIPSecRwRtStArmScrnPosMin_Val : Constant  Value=KeSMSw6sVIPSecRwRtStArmScrnPosMin_Val
  PA_KeSMSw6sVIPSecRwRtStArmScrnPos_Val : Constant  Value=KeSMSw6sVIPSecRwRtStArmScrnPos_Val
  PA_KeSMSw6sVIPSecRwRtStBkReclnUpwdDnwdPosMax_Val : Constant  Value=KeSMSw6sVIPSecRwRtStBkReclnUpwdDnwdPosMax_Val
  PA_KeSMSw6sVIPSecRwRtStBkReclnUpwdDnwdPosMin_Val : Constant  Value=KeSMSw6sVIPSecRwRtStBkReclnUpwdDnwdPosMin_Val
  PA_KeSMSw6sVIPSecRwRtStBkReclnUpwdDnwdPos_Val : Constant  Value=KeSMSw6sVIPSecRwRtStBkReclnUpwdDnwdPos_Val
  PA_KeSMSw6sVIPSecRwRtStFrwdBkwdPosMax_Val : Constant  Value=KeSMSw6sVIPSecRwRtStFrwdBkwdPosMax_Val
  PA_KeSMSw6sVIPSecRwRtStFrwdBkwdPosMin_Val : Constant  Value=KeSMSw6sVIPSecRwRtStFrwdBkwdPosMin_Val
  PA_KeSMSw6sVIPSecRwRtStFrwdBkwdPos_Val : Constant  Value=KeSMSw6sVIPSecRwRtStFrwdBkwdPos_Val
  PA_KeSMSw6sVIPSecRwRtStHdrstUpwdPosMax_Val : Constant  Value=KeSMSw6sVIPSecRwRtStHdrstUpwdPosMax_Val
  PA_KeSMSw6sVIPSecRwRtStHdrstUpwdPosMin_Val : Constant  Value=KeSMSw6sVIPSecRwRtStHdrstUpwdPosMin_Val
  PA_KeSMSw6sVIPSecRwRtStHdrstUpwdPos_Val : Constant  Value=KeSMSw6sVIPSecRwRtStHdrstUpwdPos_Val
  PA_KeSMSw6sVIPSecRwRtStLgrstUpwdPosMax_Val : Constant  Value=KeSMSw6sVIPSecRwRtStLgrstUpwdPosMax_Val
  PA_KeSMSw6sVIPSecRwRtStLgrstUpwdPosMin_Val : Constant  Value=KeSMSw6sVIPSecRwRtStLgrstUpwdPosMin_Val
  PA_KeSMSw6sVIPSecRwRtStLgrstUpwdPos_Val : Constant  Value=KeSMSw6sVIPSecRwRtStLgrstUpwdPos_Val
  PA_KeSMSw6sVIPSecRwRtStLtwdRtwdPosMax_Val : Constant  Value=KeSMSw6sVIPSecRwRtStLtwdRtwdPosMax_Val
  PA_KeSMSw6sVIPSecRwRtStLtwdRtwdPosMin_Val : Constant  Value=KeSMSw6sVIPSecRwRtStLtwdRtwdPosMin_Val
  PA_KeSMSw6sVIPSecRwRtStLtwdRtwdPos_Val : Constant  Value=KeSMSw6sVIPSecRwRtStLtwdRtwdPos_Val
  PA_KeSMSw6sVIPThdRwLtStBkReclnUpwdDnwdPosMax_Val : Constant  Value=KeSMSw6sVIPThdRwLtStBkReclnUpwdDnwdPosMax_Val
  PA_KeSMSw6sVIPThdRwLtStBkReclnUpwdDnwdPosMin_Val : Constant  Value=KeSMSw6sVIPThdRwLtStBkReclnUpwdDnwdPosMin_Val
  PA_KeSMSw6sVIPThdRwLtStBkReclnUpwdDnwdPos_Val : Constant  Value=KeSMSw6sVIPThdRwLtStBkReclnUpwdDnwdPos_Val
  PA_KeSMSw6sVIPThdRwLtStCshnFldUpwdDnwdPosMax_Val : Constant  Value=KeSMSw6sVIPThdRwLtStCshnFldUpwdDnwdPosMax_Val
  PA_KeSMSw6sVIPThdRwLtStCshnFldUpwdDnwdPosMin_Val : Constant  Value=KeSMSw6sVIPThdRwLtStCshnFldUpwdDnwdPosMin_Val
  PA_KeSMSw6sVIPThdRwLtStCshnFldUpwdDnwdPos_Val : Constant  Value=KeSMSw6sVIPThdRwLtStCshnFldUpwdDnwdPos_Val
  PA_KeSMSw6sVIPThdRwLtStFrwdBkwdPosMax_Val : Constant  Value=KeSMSw6sVIPThdRwLtStFrwdBkwdPosMax_Val
  PA_KeSMSw6sVIPThdRwLtStFrwdBkwdPosMin_Val : Constant  Value=KeSMSw6sVIPThdRwLtStFrwdBkwdPosMin_Val
  PA_KeSMSw6sVIPThdRwLtStFrwdBkwdPos_Val : Constant  Value=KeSMSw6sVIPThdRwLtStFrwdBkwdPos_Val
  PA_KeSMSw6sVIPThdRwRtStBkReclnUpwdDnwdPosMax_Val : Constant  Value=KeSMSw6sVIPThdRwRtStBkReclnUpwdDnwdPosMax_Val
  PA_KeSMSw6sVIPThdRwRtStBkReclnUpwdDnwdPosMin_Val : Constant  Value=KeSMSw6sVIPThdRwRtStBkReclnUpwdDnwdPosMin_Val
  PA_KeSMSw6sVIPThdRwRtStBkReclnUpwdDnwdPos_Val : Constant  Value=KeSMSw6sVIPThdRwRtStBkReclnUpwdDnwdPos_Val
  PA_KeSMSw6sVIPThdRwRtStCshnFldUpwdDnwdPosMax_Val : Constant  Value=KeSMSw6sVIPThdRwRtStCshnFldUpwdDnwdPosMax_Val
  PA_KeSMSw6sVIPThdRwRtStCshnFldUpwdDnwdPosMin_Val : Constant  Value=KeSMSw6sVIPThdRwRtStCshnFldUpwdDnwdPosMin_Val
  PA_KeSMSw6sVIPThdRwRtStCshnFldUpwdDnwdPos_Val : Constant  Value=KeSMSw6sVIPThdRwRtStCshnFldUpwdDnwdPos_Val
  PA_KeSMSw6sVIPThdRwRtStFrwdBkwdPosMax_Val : Constant  Value=KeSMSw6sVIPThdRwRtStFrwdBkwdPosMax_Val
  PA_KeSMSw6sVIPThdRwRtStFrwdBkwdPosMin_Val : Constant  Value=KeSMSw6sVIPThdRwRtStFrwdBkwdPosMin_Val
  PA_KeSMSw6sVIPThdRwRtStFrwdBkwdPos_Val : Constant  Value=KeSMSw6sVIPThdRwRtStFrwdBkwdPos_Val
  PA_KeSMSwAcsEntryDrvStBkReclnUpwdDnwdPosMax_Val : Constant  Value=KeSMSwAcsEntryDrvStBkReclnUpwdDnwdPosMax_Val
  PA_KeSMSwAcsEntryDrvStBkReclnUpwdDnwdPosMin_Val : Constant  Value=KeSMSwAcsEntryDrvStBkReclnUpwdDnwdPosMin_Val
  PA_KeSMSwAcsEntryDrvStBkReclnUpwdDnwdPos_Val : Constant  Value=KeSMSwAcsEntryDrvStBkReclnUpwdDnwdPos_Val
  PA_KeSMSwAcsEntryDrvStFrwdBkwdPosMax_Val : Constant  Value=KeSMSwAcsEntryDrvStFrwdBkwdPosMax_Val
  PA_KeSMSwAcsEntryDrvStFrwdBkwdPosMin_Val : Constant  Value=KeSMSwAcsEntryDrvStFrwdBkwdPosMin_Val
  PA_KeSMSwAcsEntryDrvStFrwdBkwdPos_Val : Constant  Value=KeSMSwAcsEntryDrvStFrwdBkwdPos_Val
  PA_KeSMSwAcsEntryDrvStFtUpwdDnwdPosMax_Val : Constant  Value=KeSMSwAcsEntryDrvStFtUpwdDnwdPosMax_Val
  PA_KeSMSwAcsEntryDrvStFtUpwdDnwdPosMin_Val : Constant  Value=KeSMSwAcsEntryDrvStFtUpwdDnwdPosMin_Val
  PA_KeSMSwAcsEntryDrvStFtUpwdDnwdPos_Val : Constant  Value=KeSMSwAcsEntryDrvStFtUpwdDnwdPos_Val
  PA_KeSMSwAcsEntryPassStBkReclnUpwdDnwdPosMax_Val : Constant  Value=KeSMSwAcsEntryPassStBkReclnUpwdDnwdPosMax_Val
  PA_KeSMSwAcsEntryPassStBkReclnUpwdDnwdPosMin_Val : Constant  Value=KeSMSwAcsEntryPassStBkReclnUpwdDnwdPosMin_Val
  PA_KeSMSwAcsEntryPassStBkReclnUpwdDnwdPos_Val : Constant  Value=KeSMSwAcsEntryPassStBkReclnUpwdDnwdPos_Val
  PA_KeSMSwAcsEntryPassStFrwdBkwdPosMax_Val : Constant  Value=KeSMSwAcsEntryPassStFrwdBkwdPosMax_Val
  PA_KeSMSwAcsEntryPassStFrwdBkwdPosMin_Val : Constant  Value=KeSMSwAcsEntryPassStFrwdBkwdPosMin_Val
  PA_KeSMSwAcsEntryPassStFrwdBkwdPos_Val : Constant  Value=KeSMSwAcsEntryPassStFrwdBkwdPos_Val
  PA_KeSMSwAcsEntryPassStFtUpwdDnwdPosMiax_Val : Constant  Value=KeSMSwAcsEntryPassStFtUpwdDnwdPosMiax_Val
  PA_KeSMSwAcsEntryPassStFtUpwdDnwdPosMin_Val : Constant  Value=KeSMSwAcsEntryPassStFtUpwdDnwdPosMin_Val
  PA_KeSMSwAcsEntryPassStFtUpwdDnwdPos_Val : Constant  Value=KeSMSwAcsEntryPassStFtUpwdDnwdPos_Val
  PA_KeSMSwAcsEntrySecRwLtStArmScrnPosMax_Val : Constant  Value=KeSMSwAcsEntrySecRwLtStArmScrnPosMax_Val
  PA_KeSMSwAcsEntrySecRwLtStArmScrnPosMin_Val : Constant  Value=KeSMSwAcsEntrySecRwLtStArmScrnPosMin_Val
  PA_KeSMSwAcsEntrySecRwLtStArmScrnPos_Val : Constant  Value=KeSMSwAcsEntrySecRwLtStArmScrnPos_Val
  PA_KeSMSwAcsEntrySecRwLtStBkReclnUpwdDnwdPosMax_Val : Constant  Value=KeSMSwAcsEntrySecRwLtStBkReclnUpwdDnwdPosMax_Val
  PA_KeSMSwAcsEntrySecRwLtStBkReclnUpwdDnwdPosMin_Val : Constant  Value=KeSMSwAcsEntrySecRwLtStBkReclnUpwdDnwdPosMin_Val
  PA_KeSMSwAcsEntrySecRwLtStBkReclnUpwdDnwdPos_Val : Constant  Value=KeSMSwAcsEntrySecRwLtStBkReclnUpwdDnwdPos_Val
  PA_KeSMSwAcsEntrySecRwLtStFrwdBkwdPosMax_Val : Constant  Value=KeSMSwAcsEntrySecRwLtStFrwdBkwdPosMax_Val
  PA_KeSMSwAcsEntrySecRwLtStFrwdBkwdPosMin_Val : Constant  Value=KeSMSwAcsEntrySecRwLtStFrwdBkwdPosMin_Val
  PA_KeSMSwAcsEntrySecRwLtStFrwdBkwdPos_Val : Constant  Value=KeSMSwAcsEntrySecRwLtStFrwdBkwdPos_Val
  PA_KeSMSwAcsEntrySecRwLtStHdrstUpwdPosMax_Val : Constant  Value=KeSMSwAcsEntrySecRwLtStHdrstUpwdPosMax_Val
  PA_KeSMSwAcsEntrySecRwLtStHdrstUpwdPosMin_Val : Constant  Value=KeSMSwAcsEntrySecRwLtStHdrstUpwdPosMin_Val
  PA_KeSMSwAcsEntrySecRwLtStHdrstUpwdPos_Val : Constant  Value=KeSMSwAcsEntrySecRwLtStHdrstUpwdPos_Val
  PA_KeSMSwAcsEntrySecRwLtStLgrstUpwdPosMax_Val : Constant  Value=KeSMSwAcsEntrySecRwLtStLgrstUpwdPosMax_Val
  PA_KeSMSwAcsEntrySecRwLtStLgrstUpwdPosMin_Val : Constant  Value=KeSMSwAcsEntrySecRwLtStLgrstUpwdPosMin_Val
  PA_KeSMSwAcsEntrySecRwLtStLgrstUpwdPos_Val : Constant  Value=KeSMSwAcsEntrySecRwLtStLgrstUpwdPos_Val
  PA_KeSMSwAcsEntrySecRwLtStLtwdRtwdPosMax_Val : Constant  Value=KeSMSwAcsEntrySecRwLtStLtwdRtwdPosMax_Val
  PA_KeSMSwAcsEntrySecRwLtStLtwdRtwdPosMin_Val : Constant  Value=KeSMSwAcsEntrySecRwLtStLtwdRtwdPosMin_Val
  PA_KeSMSwAcsEntrySecRwLtStLtwdRtwdPos_Val : Constant  Value=KeSMSwAcsEntrySecRwLtStLtwdRtwdPos_Val
  PA_KeSMSwAcsEntrySecRwRtStArmScrnPosMax_Val : Constant  Value=KeSMSwAcsEntrySecRwRtStArmScrnPosMax_Val
  PA_KeSMSwAcsEntrySecRwRtStArmScrnPosMin_Val : Constant  Value=KeSMSwAcsEntrySecRwRtStArmScrnPosMin_Val
  PA_KeSMSwAcsEntrySecRwRtStArmScrnPos_Val : Constant  Value=KeSMSwAcsEntrySecRwRtStArmScrnPos_Val
  PA_KeSMSwAcsEntrySecRwRtStBkReclnUpwdDnwdPosMax_Val : Constant  Value=KeSMSwAcsEntrySecRwRtStBkReclnUpwdDnwdPosMax_Val
  PA_KeSMSwAcsEntrySecRwRtStBkReclnUpwdDnwdPosMin_Val : Constant  Value=KeSMSwAcsEntrySecRwRtStBkReclnUpwdDnwdPosMin_Val
  PA_KeSMSwAcsEntrySecRwRtStBkReclnUpwdDnwdPos_Val : Constant  Value=KeSMSwAcsEntrySecRwRtStBkReclnUpwdDnwdPos_Val
  PA_KeSMSwAcsEntrySecRwRtStFrwdBkwdPosMax_Val : Constant  Value=KeSMSwAcsEntrySecRwRtStFrwdBkwdPosMax_Val
  PA_KeSMSwAcsEntrySecRwRtStFrwdBkwdPosMin_Val : Constant  Value=KeSMSwAcsEntrySecRwRtStFrwdBkwdPosMin_Val
  PA_KeSMSwAcsEntrySecRwRtStFrwdBkwdPos_Val : Constant  Value=KeSMSwAcsEntrySecRwRtStFrwdBkwdPos_Val
  PA_KeSMSwAcsEntrySecRwRtStHdrstUpwdPosMax_Val : Constant  Value=KeSMSwAcsEntrySecRwRtStHdrstUpwdPosMax_Val
  PA_KeSMSwAcsEntrySecRwRtStHdrstUpwdPosMin_Val : Constant  Value=KeSMSwAcsEntrySecRwRtStHdrstUpwdPosMin_Val
  PA_KeSMSwAcsEntrySecRwRtStHdrstUpwdPos_Val : Constant  Value=KeSMSwAcsEntrySecRwRtStHdrstUpwdPos_Val
  PA_KeSMSwAcsEntrySecRwRtStLgrstUpwdPosMax_Val : Constant  Value=KeSMSwAcsEntrySecRwRtStLgrstUpwdPosMax_Val
  PA_KeSMSwAcsEntrySecRwRtStLgrstUpwdPosMin_Val : Constant  Value=KeSMSwAcsEntrySecRwRtStLgrstUpwdPosMin_Val
  PA_KeSMSwAcsEntrySecRwRtStLgrstUpwdPos_Val : Constant  Value=KeSMSwAcsEntrySecRwRtStLgrstUpwdPos_Val
  PA_KeSMSwAcsEntrySecRwRtStLtwdRtwdPosMax_Val : Constant  Value=KeSMSwAcsEntrySecRwRtStLtwdRtwdPosMax_Val
  PA_KeSMSwAcsEntrySecRwRtStLtwdRtwdPosMin_Val : Constant  Value=KeSMSwAcsEntrySecRwRtStLtwdRtwdPosMin_Val
  PA_KeSMSwAcsEntrySecRwRtStLtwdRtwdPos_Val : Constant  Value=KeSMSwAcsEntrySecRwRtStLtwdRtwdPos_Val
  PA_KeSMSwAcsEntryThdRwLtStBkReclnUpwdDnwdPosMax_Val : Constant  Value=KeSMSwAcsEntryThdRwLtStBkReclnUpwdDnwdPosMax_Val
  PA_KeSMSwAcsEntryThdRwLtStBkReclnUpwdDnwdPosMin_Val : Constant  Value=KeSMSwAcsEntryThdRwLtStBkReclnUpwdDnwdPosMin_Val
  PA_KeSMSwAcsEntryThdRwLtStBkReclnUpwdDnwdPos_Val : Constant  Value=KeSMSwAcsEntryThdRwLtStBkReclnUpwdDnwdPos_Val
  PA_KeSMSwAcsEntryThdRwLtStCshnFldUpwdDnwdPosMax_Val : Constant  Value=KeSMSwAcsEntryThdRwLtStCshnFldUpwdDnwdPosMax_Val
  PA_KeSMSwAcsEntryThdRwLtStCshnFldUpwdDnwdPosMin_Val : Constant  Value=KeSMSwAcsEntryThdRwLtStCshnFldUpwdDnwdPosMin_Val
  PA_KeSMSwAcsEntryThdRwLtStCshnFldUpwdDnwdPos_Val : Constant  Value=KeSMSwAcsEntryThdRwLtStCshnFldUpwdDnwdPos_Val
  PA_KeSMSwAcsEntryThdRwLtStFrwdBkwdPosMax_Val : Constant  Value=KeSMSwAcsEntryThdRwLtStFrwdBkwdPosMax_Val
  PA_KeSMSwAcsEntryThdRwLtStFrwdBkwdPosMin_Val : Constant  Value=KeSMSwAcsEntryThdRwLtStFrwdBkwdPosMin_Val
  PA_KeSMSwAcsEntryThdRwLtStFrwdBkwdPos_Val : Constant  Value=KeSMSwAcsEntryThdRwLtStFrwdBkwdPos_Val
  PA_KeSMSwAcsEntryThdRwRtStBkReclnUpwdDnwdPosMax_Val : Constant  Value=KeSMSwAcsEntryThdRwRtStBkReclnUpwdDnwdPosMax_Val
  PA_KeSMSwAcsEntryThdRwRtStBkReclnUpwdDnwdPosMin_Val : Constant  Value=KeSMSwAcsEntryThdRwRtStBkReclnUpwdDnwdPosMin_Val
  PA_KeSMSwAcsEntryThdRwRtStBkReclnUpwdDnwdPos_Val : Constant  Value=KeSMSwAcsEntryThdRwRtStBkReclnUpwdDnwdPos_Val
  PA_KeSMSwAcsEntryThdRwRtStCshnFldUpwdDnwdPosMax_Val : Constant  Value=KeSMSwAcsEntryThdRwRtStCshnFldUpwdDnwdPosMax_Val
  PA_KeSMSwAcsEntryThdRwRtStCshnFldUpwdDnwdPosMin_Val : Constant  Value=KeSMSwAcsEntryThdRwRtStCshnFldUpwdDnwdPosMin_Val
  PA_KeSMSwAcsEntryThdRwRtStCshnFldUpwdDnwdPos_Val : Constant  Value=KeSMSwAcsEntryThdRwRtStCshnFldUpwdDnwdPos_Val
  PA_KeSMSwAcsEntryThdRwRtStFrwdBkwdPosMax_Val : Constant  Value=KeSMSwAcsEntryThdRwRtStFrwdBkwdPosMax_Val
  PA_KeSMSwAcsEntryThdRwRtStFrwdBkwdPosMin_Val : Constant  Value=KeSMSwAcsEntryThdRwRtStFrwdBkwdPosMin_Val
  PA_KeSMSwAcsEntryThdRwRtStFrwdBkwdPos_Val : Constant  Value=KeSMSwAcsEntryThdRwRtStFrwdBkwdPos_Val
  PA_KeSMSwAcsExtDrvStBkReclnUpwdDnwdPosMax_Val : Constant  Value=KeSMSwAcsExtDrvStBkReclnUpwdDnwdPosMax_Val
  PA_KeSMSwAcsExtDrvStBkReclnUpwdDnwdPosMin_Val : Constant  Value=KeSMSwAcsExtDrvStBkReclnUpwdDnwdPosMin_Val
  PA_KeSMSwAcsExtDrvStBkReclnUpwdDnwdPos_Val : Constant  Value=KeSMSwAcsExtDrvStBkReclnUpwdDnwdPos_Val
  PA_KeSMSwAcsExtDrvStFrwdBkwdPosMax_Val : Constant  Value=KeSMSwAcsExtDrvStFrwdBkwdPosMax_Val
  PA_KeSMSwAcsExtDrvStFrwdBkwdPosMin_Val : Constant  Value=KeSMSwAcsExtDrvStFrwdBkwdPosMin_Val
  PA_KeSMSwAcsExtDrvStFrwdBkwdPos_Val : Constant  Value=KeSMSwAcsExtDrvStFrwdBkwdPos_Val
  PA_KeSMSwAcsExtDrvStFtUpwdDnwdPosMax_Val : Constant  Value=KeSMSwAcsExtDrvStFtUpwdDnwdPosMax_Val
  PA_KeSMSwAcsExtDrvStFtUpwdDnwdPosMin_Val : Constant  Value=KeSMSwAcsExtDrvStFtUpwdDnwdPosMin_Val
  PA_KeSMSwAcsExtDrvStFtUpwdDnwdPos_Val : Constant  Value=KeSMSwAcsExtDrvStFtUpwdDnwdPos_Val
  PA_KeSMSwAcsExtPassStBkReclnUpwdDnwdPosMax_Val : Constant  Value=KeSMSwAcsExtPassStBkReclnUpwdDnwdPosMax_Val
  PA_KeSMSwAcsExtPassStBkReclnUpwdDnwdPosMin_Val : Constant  Value=KeSMSwAcsExtPassStBkReclnUpwdDnwdPosMin_Val
  PA_KeSMSwAcsExtPassStBkReclnUpwdDnwdPos_Val : Constant  Value=KeSMSwAcsExtPassStBkReclnUpwdDnwdPos_Val
  PA_KeSMSwAcsExtPassStFrwdBkwdPosMax_Val : Constant  Value=KeSMSwAcsExtPassStFrwdBkwdPosMax_Val
  PA_KeSMSwAcsExtPassStFrwdBkwdPosMin_Val : Constant  Value=KeSMSwAcsExtPassStFrwdBkwdPosMin_Val
  PA_KeSMSwAcsExtPassStFrwdBkwdPos_Val : Constant  Value=KeSMSwAcsExtPassStFrwdBkwdPos_Val
  PA_KeSMSwAcsExtPassStFtUpwdDnwdPosMax_Val : Constant  Value=KeSMSwAcsExtPassStFtUpwdDnwdPosMax_Val
  PA_KeSMSwAcsExtPassStFtUpwdDnwdPosMin_Val : Constant  Value=KeSMSwAcsExtPassStFtUpwdDnwdPosMin_Val
  PA_KeSMSwAcsExtPassStFtUpwdDnwdPos_Val : Constant  Value=KeSMSwAcsExtPassStFtUpwdDnwdPos_Val
  PA_KeSMSwAcsExtSecRwLtStArmScrnPosMax_Val : Constant  Value=KeSMSwAcsExtSecRwLtStArmScrnPosMax_Val
  PA_KeSMSwAcsExtSecRwLtStArmScrnPosMin_Val : Constant  Value=KeSMSwAcsExtSecRwLtStArmScrnPosMin_Val
  PA_KeSMSwAcsExtSecRwLtStArmScrnPos_Val : Constant  Value=KeSMSwAcsExtSecRwLtStArmScrnPos_Val
  PA_KeSMSwAcsExtSecRwLtStBkReclnUpwdDnwdPosMax_Val : Constant  Value=KeSMSwAcsExtSecRwLtStBkReclnUpwdDnwdPosMax_Val
  PA_KeSMSwAcsExtSecRwLtStBkReclnUpwdDnwdPosMin_Val : Constant  Value=KeSMSwAcsExtSecRwLtStBkReclnUpwdDnwdPosMin_Val
  PA_KeSMSwAcsExtSecRwLtStBkReclnUpwdDnwdPos_Val : Constant  Value=KeSMSwAcsExtSecRwLtStBkReclnUpwdDnwdPos_Val
  PA_KeSMSwAcsExtSecRwLtStFrwdBkwdPosMax_Val : Constant  Value=KeSMSwAcsExtSecRwLtStFrwdBkwdPosMax_Val
  PA_KeSMSwAcsExtSecRwLtStFrwdBkwdPosMin_Val : Constant  Value=KeSMSwAcsExtSecRwLtStFrwdBkwdPosMin_Val
  PA_KeSMSwAcsExtSecRwLtStFrwdBkwdPos_Val : Constant  Value=KeSMSwAcsExtSecRwLtStFrwdBkwdPos_Val
  PA_KeSMSwAcsExtSecRwLtStLgrstUpwdDnwdPosMax_Val : Constant  Value=KeSMSwAcsExtSecRwLtStLgrstUpwdDnwdPosMax_Val
  PA_KeSMSwAcsExtSecRwLtStLgrstUpwdDnwdPosMin_Val : Constant  Value=KeSMSwAcsExtSecRwLtStLgrstUpwdDnwdPosMin_Val
  PA_KeSMSwAcsExtSecRwLtStLgrstUpwdDnwdPos_Val : Constant  Value=KeSMSwAcsExtSecRwLtStLgrstUpwdDnwdPos_Val
  PA_KeSMSwAcsExtSecRwLtStLtwdRtwdPosMax_Val : Constant  Value=KeSMSwAcsExtSecRwLtStLtwdRtwdPosMax_Val
  PA_KeSMSwAcsExtSecRwLtStLtwdRtwdPosMin_Val : Constant  Value=KeSMSwAcsExtSecRwLtStLtwdRtwdPosMin_Val
  PA_KeSMSwAcsExtSecRwLtStLtwdRtwdPos_Val : Constant  Value=KeSMSwAcsExtSecRwLtStLtwdRtwdPos_Val
  PA_KeSMSwAcsExtSecRwRtStArmScrnPosMax_Val : Constant  Value=KeSMSwAcsExtSecRwRtStArmScrnPosMax_Val
  PA_KeSMSwAcsExtSecRwRtStArmScrnPosMin_Val : Constant  Value=KeSMSwAcsExtSecRwRtStArmScrnPosMin_Val
  PA_KeSMSwAcsExtSecRwRtStArmScrnPos_Val : Constant  Value=KeSMSwAcsExtSecRwRtStArmScrnPos_Val
  PA_KeSMSwAcsExtSecRwRtStBkReclnUpwdDnwdPosMax_Val : Constant  Value=KeSMSwAcsExtSecRwRtStBkReclnUpwdDnwdPosMax_Val
  PA_KeSMSwAcsExtSecRwRtStBkReclnUpwdDnwdPosMin_Val : Constant  Value=KeSMSwAcsExtSecRwRtStBkReclnUpwdDnwdPosMin_Val
  PA_KeSMSwAcsExtSecRwRtStBkReclnUpwdDnwdPos_Val : Constant  Value=KeSMSwAcsExtSecRwRtStBkReclnUpwdDnwdPos_Val
  PA_KeSMSwAcsExtSecRwRtStFrwdBkwdPosMax_Val : Constant  Value=KeSMSwAcsExtSecRwRtStFrwdBkwdPosMax_Val
  PA_KeSMSwAcsExtSecRwRtStFrwdBkwdPosMin_Val : Constant  Value=KeSMSwAcsExtSecRwRtStFrwdBkwdPosMin_Val
  PA_KeSMSwAcsExtSecRwRtStFrwdBkwdPos_Val : Constant  Value=KeSMSwAcsExtSecRwRtStFrwdBkwdPos_Val
  PA_KeSMSwAcsExtSecRwRtStLgrstUpwdDnwdPosMax_Val : Constant  Value=KeSMSwAcsExtSecRwRtStLgrstUpwdDnwdPosMax_Val
  PA_KeSMSwAcsExtSecRwRtStLgrstUpwdDnwdPosMin_Val : Constant  Value=KeSMSwAcsExtSecRwRtStLgrstUpwdDnwdPosMin_Val
  PA_KeSMSwAcsExtSecRwRtStLgrstUpwdDnwdPos_Val : Constant  Value=KeSMSwAcsExtSecRwRtStLgrstUpwdDnwdPos_Val
  PA_KeSMSwAcsExtSecRwRtStLtwdRtwdPosMax_Val : Constant  Value=KeSMSwAcsExtSecRwRtStLtwdRtwdPosMax_Val
  PA_KeSMSwAcsExtSecRwRtStLtwdRtwdPosMin_Val : Constant  Value=KeSMSwAcsExtSecRwRtStLtwdRtwdPosMin_Val
  PA_KeSMSwAcsExtSecRwRtStLtwdRtwdPos_Val : Constant  Value=KeSMSwAcsExtSecRwRtStLtwdRtwdPos_Val
  PA_KeSMSwAcsExtThdRwLtStBkReclnUpwdDnwdPosMax_Val : Constant  Value=KeSMSwAcsExtThdRwLtStBkReclnUpwdDnwdPosMax_Val
  PA_KeSMSwAcsExtThdRwLtStBkReclnUpwdDnwdPosMin_Val : Constant  Value=KeSMSwAcsExtThdRwLtStBkReclnUpwdDnwdPosMin_Val
  PA_KeSMSwAcsExtThdRwLtStBkReclnUpwdDnwdPos_Val : Constant  Value=KeSMSwAcsExtThdRwLtStBkReclnUpwdDnwdPos_Val
  PA_KeSMSwAcsExtThdRwLtStCshnFldUpwdDnwdPosMax_Val : Constant  Value=KeSMSwAcsExtThdRwLtStCshnFldUpwdDnwdPosMax_Val
  PA_KeSMSwAcsExtThdRwLtStCshnFldUpwdDnwdPosMin_Val : Constant  Value=KeSMSwAcsExtThdRwLtStCshnFldUpwdDnwdPosMin_Val
  PA_KeSMSwAcsExtThdRwLtStCshnFldUpwdDnwdPos_Val : Constant  Value=KeSMSwAcsExtThdRwLtStCshnFldUpwdDnwdPos_Val
  PA_KeSMSwAcsExtThdRwLtStFrwdBkwdPosMax_Val : Constant  Value=KeSMSwAcsExtThdRwLtStFrwdBkwdPosMax_Val
  PA_KeSMSwAcsExtThdRwLtStFrwdBkwdPosMin_Val : Constant  Value=KeSMSwAcsExtThdRwLtStFrwdBkwdPosMin_Val
  PA_KeSMSwAcsExtThdRwLtStFrwdBkwdPos_Val : Constant  Value=KeSMSwAcsExtThdRwLtStFrwdBkwdPos_Val
  PA_KeSMSwAcsExtThdRwRtStBkReclnUpwdDnwdPosMax_Val : Constant  Value=KeSMSwAcsExtThdRwRtStBkReclnUpwdDnwdPosMax_Val
  PA_KeSMSwAcsExtThdRwRtStBkReclnUpwdDnwdPosMin_Val : Constant  Value=KeSMSwAcsExtThdRwRtStBkReclnUpwdDnwdPosMin_Val
  PA_KeSMSwAcsExtThdRwRtStBkReclnUpwdDnwdPos_Val : Constant  Value=KeSMSwAcsExtThdRwRtStBkReclnUpwdDnwdPos_Val
  PA_KeSMSwAcsExtThdRwRtStCshnFldUpwdDnwdPosMax_Val : Constant  Value=KeSMSwAcsExtThdRwRtStCshnFldUpwdDnwdPosMax_Val
  PA_KeSMSwAcsExtThdRwRtStCshnFldUpwdDnwdPosMin_Val : Constant  Value=KeSMSwAcsExtThdRwRtStCshnFldUpwdDnwdPosMin_Val
  PA_KeSMSwAcsExtThdRwRtStCshnFldUpwdDnwdPos_Val : Constant  Value=KeSMSwAcsExtThdRwRtStCshnFldUpwdDnwdPos_Val
  PA_KeSMSwAcsExtThdRwRtStFrwdBkwdPosMax_Val : Constant  Value=KeSMSwAcsExtThdRwRtStFrwdBkwdPosMax_Val
  PA_KeSMSwAcsExtThdRwRtStFrwdBkwdPosMin_Val : Constant  Value=KeSMSwAcsExtThdRwRtStFrwdBkwdPosMin_Val
  PA_KeSMSwAcsExtThdRwRtStFrwdBkwdPos_Val : Constant  Value=KeSMSwAcsExtThdRwRtStFrwdBkwdPos_Val
  PA_KeSMSwDltTrgtPos_Val{1..360} (360 alike) : Constant  Value=KeSMSwPosInvalidVal_Val
  PA_KeSMSwFamilyLMdThdRwLtStFrwdBkwdPosMax_Val : Constant  Value=KeSMSwFamilyLMdThdRwLtStFrwdBkwdPosMax_Val
  PA_KeSMSwFamilyLMdThdRwLtStFrwdBkwdPosMin_Val : Constant  Value=KeSMSwFamilyLMdThdRwLtStFrwdBkwdPosMin_Val
  PA_KeSMSwFamilyLMdThdRwLtStFrwdBkwdPos_Val : Constant  Value=KeSMSwFamilyLMdThdRwLtStFrwdBkwdPos_Val
  PA_KeSMSwFamilyMdSecRwLtStFrwdBkwdPosMax_Val : Constant  Value=KeSMSwFamilyMdSecRwLtStFrwdBkwdPosMax_Val
  PA_KeSMSwFamilyMdSecRwLtStFrwdBkwdPosMin_Val : Constant  Value=KeSMSwFamilyMdSecRwLtStFrwdBkwdPosMin_Val
  PA_KeSMSwFamilyMdSecRwLtStFrwdBkwdPos_Val : Constant  Value=KeSMSwFamilyMdSecRwLtStFrwdBkwdPos_Val
  PA_KeSMSwFamilyMdSecRwLtStLtwdRtwdPosMax_Val : Constant  Value=KeSMSwFamilyMdSecRwLtStLtwdRtwdPosMax_Val
  PA_KeSMSwFamilyMdSecRwLtStLtwdRtwdPosMin_Val : Constant  Value=KeSMSwFamilyMdSecRwLtStLtwdRtwdPosMin_Val
  PA_KeSMSwFamilyMdSecRwLtStLtwdRtwdPos_Val : Constant  Value=KeSMSwFamilyMdSecRwLtStLtwdRtwdPos_Val
  PA_KeSMSwFamilyMdSecRwRtStFrwdBkwdPosMax_Val : Constant  Value=KeSMSwFamilyMdSecRwRtStFrwdBkwdPosMax_Val
  PA_KeSMSwFamilyMdSecRwRtStFrwdBkwdPosMin_Val : Constant  Value=KeSMSwFamilyMdSecRwRtStFrwdBkwdPosMin_Val
  PA_KeSMSwFamilyMdSecRwRtStFrwdBkwdPos_Val : Constant  Value=KeSMSwFamilyMdSecRwRtStFrwdBkwdPos_Val
  PA_KeSMSwFamilyMdSecRwRtStLtwdRtwdPosMax_Val : Constant  Value=KeSMSwFamilyMdSecRwRtStLtwdRtwdPosMax_Val
  PA_KeSMSwFamilyMdSecRwRtStLtwdRtwdPosMin_Val : Constant  Value=KeSMSwFamilyMdSecRwRtStLtwdRtwdPosMin_Val
  PA_KeSMSwFamilyMdSecRwRtStLtwdRtwdPos_Val : Constant  Value=KeSMSwFamilyMdSecRwRtStLtwdRtwdPos_Val
  PA_KeSMSwFamilyMdThdRwLtStFrwdBkwdPosMax_Val : Constant  Value=KeSMSwFamilyMdThdRwLtStFrwdBkwdPosMax_Val
  PA_KeSMSwFamilyMdThdRwLtStFrwdBkwdPosMin_Val : Constant  Value=KeSMSwFamilyMdThdRwLtStFrwdBkwdPosMin_Val
  PA_KeSMSwFamilyMdThdRwLtStFrwdBkwdPos_Val : Constant  Value=KeSMSwFamilyMdThdRwLtStFrwdBkwdPos_Val
  PA_KeSMSwFamilyMdThdRwRtStFrwdBkwdPosMax_Val : Constant  Value=KeSMSwFamilyMdThdRwRtStFrwdBkwdPosMax_Val
  PA_KeSMSwFamilyMdThdRwRtStFrwdBkwdPosMin_Val : Constant  Value=KeSMSwFamilyMdThdRwRtStFrwdBkwdPosMin_Val
  PA_KeSMSwFamilyMdThdRwRtStFrwdBkwdPos_Val : Constant  Value=KeSMSwFamilyMdThdRwRtStFrwdBkwdPos_Val
  PA_KeSMSwFamilyRMdSecRwLtStFrwdBkwdPosMax_Val : Constant  Value=KeSMSwFamilyRMdSecRwLtStFrwdBkwdPosMax_Val
  PA_KeSMSwFamilyRMdSecRwLtStFrwdBkwdPosMin_Val : Constant  Value=KeSMSwFamilyRMdSecRwLtStFrwdBkwdPosMin_Val
  PA_KeSMSwFamilyRMdSecRwLtStFrwdBkwdPos_Val : Constant  Value=KeSMSwFamilyRMdSecRwLtStFrwdBkwdPos_Val
  PA_KeSMSwFamilyRMdSecRwLtStLtwdRtwdPosMax_Val : Constant  Value=KeSMSwFamilyRMdSecRwLtStLtwdRtwdPosMax_Val
  PA_KeSMSwFamilyRMdSecRwLtStLtwdRtwdPosMin_Val : Constant  Value=KeSMSwFamilyRMdSecRwLtStLtwdRtwdPosMin_Val
  PA_KeSMSwFamilyRMdSecRwLtStLtwdRtwdPos_Val : Constant  Value=KeSMSwFamilyRMdSecRwLtStLtwdRtwdPos_Val
  PA_KeSMSwFamilyRMdSecRwRtStFrwdBkwdPosMax_Val : Constant  Value=KeSMSwFamilyRMdSecRwRtStFrwdBkwdPosMax_Val
  PA_KeSMSwFamilyRMdSecRwRtStFrwdBkwdPosMin_Val : Constant  Value=KeSMSwFamilyRMdSecRwRtStFrwdBkwdPosMin_Val
  PA_KeSMSwFamilyRMdSecRwRtStFrwdBkwdPos_Val : Constant  Value=KeSMSwFamilyRMdSecRwRtStFrwdBkwdPos_Val
  PA_KeSMSwFamilyRMdSecRwRtStLtwdRtwdPosMax_Val : Constant  Value=KeSMSwFamilyRMdSecRwRtStLtwdRtwdPosMax_Val
  PA_KeSMSwFamilyRMdSecRwRtStLtwdRtwdPosMin_Val : Constant  Value=KeSMSwFamilyRMdSecRwRtStLtwdRtwdPosMin_Val
  PA_KeSMSwFamilyRMdSecRwRtStLtwdRtwdPos_Val : Constant  Value=KeSMSwFamilyRMdSecRwRtStLtwdRtwdPos_Val
  PA_KeSMSwFamilyRMdThdRwRtStFrwdBkwdPosMax_Val : Constant  Value=KeSMSwFamilyRMdThdRwRtStFrwdBkwdPosMax_Val
  PA_KeSMSwFamilyRMdThdRwRtStFrwdBkwdPosMin_Val : Constant  Value=KeSMSwFamilyRMdThdRwRtStFrwdBkwdPosMin_Val
  PA_KeSMSwFamilyRMdThdRwRtStFrwdBkwdPos_Val : Constant  Value=KeSMSwFamilyRMdThdRwRtStFrwdBkwdPos_Val
  PA_KeSMSwIntimacyMdSecRwLtStLtwdRtwdPosMax_Val : Constant  Value=KeSMSwIntimacyMdSecRwLtStLtwdRtwdPosMax_Val
  PA_KeSMSwIntimacyMdSecRwLtStLtwdRtwdPosMin_Val : Constant  Value=KeSMSwIntimacyMdSecRwLtStLtwdRtwdPosMin_Val
  PA_KeSMSwIntimacyMdSecRwLtStLtwdRtwdPos_Val : Constant  Value=KeSMSwIntimacyMdSecRwLtStLtwdRtwdPos_Val
  PA_KeSMSwIntimacyMdSecRwRtStLtwdRtwdPosMax_Val : Constant  Value=KeSMSwIntimacyMdSecRwRtStLtwdRtwdPosMax_Val
  PA_KeSMSwIntimacyMdSecRwRtStLtwdRtwdPosMin_Val : Constant  Value=KeSMSwIntimacyMdSecRwRtStLtwdRtwdPosMin_Val
  PA_KeSMSwIntimacyMdSecRwRtStLtwdRtwdPos_Val : Constant  Value=KeSMSwIntimacyMdSecRwRtStLtwdRtwdPos_Val
  PA_KeSMSwIntimacyRMdSecRwLtStLtwdRtwdPosMax_Val : Constant  Value=KeSMSwIntimacyRMdSecRwLtStLtwdRtwdPosMax_Val
  PA_KeSMSwIntimacyRMdSecRwLtStLtwdRtwdPosMin_Val : Constant  Value=KeSMSwIntimacyRMdSecRwLtStLtwdRtwdPosMin_Val
  PA_KeSMSwIntimacyRMdSecRwLtStLtwdRtwdPos_Val : Constant  Value=KeSMSwIntimacyRMdSecRwLtStLtwdRtwdPos_Val
  PA_KeSMSwIntimacyRMdSecRwRtStLtwdRtwdPosMax_Val : Constant  Value=KeSMSwIntimacyRMdSecRwRtStLtwdRtwdPosMax_Val
  PA_KeSMSwIntimacyRMdSecRwRtStLtwdRtwdPosMin_Val : Constant  Value=KeSMSwIntimacyRMdSecRwRtStLtwdRtwdPosMin_Val
  PA_KeSMSwIntimacyRMdSecRwRtStLtwdRtwdPos_Val : Constant  Value=KeSMSwIntimacyRMdSecRwRtStLtwdRtwdPos_Val
  PA_KeSMSwLugThdRwLtStBkReclnUpwdDnwdPosMax_Val : Constant  Value=KeSMSwLugThdRwLtStBkReclnUpwdDnwdPosMax_Val
  PA_KeSMSwLugThdRwLtStBkReclnUpwdDnwdPosMin_Val : Constant  Value=KeSMSwLugThdRwLtStBkReclnUpwdDnwdPosMin_Val
  PA_KeSMSwLugThdRwLtStBkReclnUpwdDnwdPos_Val : Constant  Value=KeSMSwLugThdRwLtStBkReclnUpwdDnwdPos_Val
  PA_KeSMSwLugThdRwLtStCshnFldUpwdDnwdPosMax_Val : Constant  Value=KeSMSwLugThdRwLtStCshnFldUpwdDnwdPosMax_Val
  PA_KeSMSwLugThdRwLtStCshnFldUpwdDnwdPosMin_Val : Constant  Value=KeSMSwLugThdRwLtStCshnFldUpwdDnwdPosMin_Val
  PA_KeSMSwLugThdRwLtStCshnFldUpwdDnwdPos_Val : Constant  Value=KeSMSwLugThdRwLtStCshnFldUpwdDnwdPos_Val
  PA_KeSMSwLugThdRwLtStFrwdBkwdPosMax_Val : Constant  Value=KeSMSwLugThdRwLtStFrwdBkwdPosMax_Val
  PA_KeSMSwLugThdRwLtStFrwdBkwdPosMin_Val : Constant  Value=KeSMSwLugThdRwLtStFrwdBkwdPosMin_Val
  PA_KeSMSwLugThdRwLtStFrwdBkwdPos_Val : Constant  Value=KeSMSwLugThdRwLtStFrwdBkwdPos_Val
  PA_KeSMSwLugThdRwRtStBkReclnUpwdDnwdPosMax_Val : Constant  Value=KeSMSwLugThdRwRtStBkReclnUpwdDnwdPosMax_Val
  PA_KeSMSwLugThdRwRtStBkReclnUpwdDnwdPosMin_Val : Constant  Value=KeSMSwLugThdRwRtStBkReclnUpwdDnwdPosMin_Val
  PA_KeSMSwLugThdRwRtStBkReclnUpwdDnwdPos_Val : Constant  Value=KeSMSwLugThdRwRtStBkReclnUpwdDnwdPos_Val
  PA_KeSMSwLugThdRwRtStCshnFldUpwdDnwdPosMax_Val : Constant  Value=KeSMSwLugThdRwRtStCshnFldUpwdDnwdPosMax_Val
  PA_KeSMSwLugThdRwRtStCshnFldUpwdDnwdPosMin_Val : Constant  Value=KeSMSwLugThdRwRtStCshnFldUpwdDnwdPosMin_Val
  PA_KeSMSwLugThdRwRtStCshnFldUpwdDnwdPos_Val : Constant  Value=KeSMSwLugThdRwRtStCshnFldUpwdDnwdPos_Val
  PA_KeSMSwLugThdRwRtStFrwdBkwdPosMax_Val : Constant  Value=KeSMSwLugThdRwRtStFrwdBkwdPosMax_Val
  PA_KeSMSwLugThdRwRtStFrwdBkwdPosMin_Val : Constant  Value=KeSMSwLugThdRwRtStFrwdBkwdPosMin_Val
  PA_KeSMSwLugThdRwRtStFrwdBkwdPos_Val : Constant  Value=KeSMSwLugThdRwRtStFrwdBkwdPos_Val
  PA_KeSMSwRecoveryDrvStFtUpwdDnwdPosMax_Val : Constant  Value=KeSMSwRecoveryDrvStFtUpwdDnwdPosMax_Val
  PA_KeSMSwRecoveryDrvStFtUpwdDnwdPosMin_Val : Constant  Value=KeSMSwRecoveryDrvStFtUpwdDnwdPosMin_Val
  PA_KeSMSwRecoveryDrvStFtUpwdDnwdPos_Val : Constant  Value=KeSMSwRecoveryDrvStFtUpwdDnwdPos_Val
  PA_KeSMSwRecoveryMdSecRwLtStArmScrnPosMax_Val : Constant  Value=KeSMSwRecoveryMdSecRwLtStArmScrnPosMax_Val
  PA_KeSMSwRecoveryMdSecRwLtStArmScrnPosMin_Val : Constant  Value=KeSMSwRecoveryMdSecRwLtStArmScrnPosMin_Val
  PA_KeSMSwRecoveryMdSecRwLtStArmScrnPos_Val : Constant  Value=KeSMSwRecoveryMdSecRwLtStArmScrnPos_Val
  PA_KeSMSwRecoveryMdSecRwLtStBkReclnUpwdDnwdPosMax_Val : Constant  Value=KeSMSwRecoveryMdSecRwLtStBkReclnUpwdDnwdPosMax_Val
  PA_KeSMSwRecoveryMdSecRwLtStBkReclnUpwdDnwdPosMin_Val : Constant  Value=KeSMSwRecoveryMdSecRwLtStBkReclnUpwdDnwdPosMin_Val
  PA_KeSMSwRecoveryMdSecRwLtStBkReclnUpwdDnwdPos_Val : Constant  Value=KeSMSwRecoveryMdSecRwLtStBkReclnUpwdDnwdPos_Val
  PA_KeSMSwRecoveryMdSecRwLtStFrwdBkwdPosMax_Val : Constant  Value=KeSMSwRecoveryMdSecRwLtStFrwdBkwdPosMax_Val
  PA_KeSMSwRecoveryMdSecRwLtStFrwdBkwdPosMin_Val : Constant  Value=KeSMSwRecoveryMdSecRwLtStFrwdBkwdPosMin_Val
  PA_KeSMSwRecoveryMdSecRwLtStFrwdBkwdPos_Val : Constant  Value=KeSMSwRecoveryMdSecRwLtStFrwdBkwdPos_Val
  PA_KeSMSwRecoveryMdSecRwLtStHdrstUpwdDnwdPosMax_Val : Constant  Value=KeSMSwRecoveryMdSecRwLtStHdrstUpwdDnwdPosMax_Val
  PA_KeSMSwRecoveryMdSecRwLtStHdrstUpwdDnwdPosMin_Val : Constant  Value=KeSMSwRecoveryMdSecRwLtStHdrstUpwdDnwdPosMin_Val
  PA_KeSMSwRecoveryMdSecRwLtStHdrstUpwdDnwdPos_Val : Constant  Value=KeSMSwRecoveryMdSecRwLtStHdrstUpwdDnwdPos_Val
  PA_KeSMSwRecoveryMdSecRwLtStLgrstUpwdDnwdPosMax_Val : Constant  Value=KeSMSwRecoveryMdSecRwLtStLgrstUpwdDnwdPosMax_Val
  PA_KeSMSwRecoveryMdSecRwLtStLgrstUpwdDnwdPosMin_Val : Constant  Value=KeSMSwRecoveryMdSecRwLtStLgrstUpwdDnwdPosMin_Val
  PA_KeSMSwRecoveryMdSecRwLtStLgrstUpwdDnwdPos_Val : Constant  Value=KeSMSwRecoveryMdSecRwLtStLgrstUpwdDnwdPos_Val
  PA_KeSMSwRecoveryMdSecRwLtStLtwdRtwdPosMax_Val : Constant  Value=KeSMSwRecoveryMdSecRwLtStLtwdRtwdPosMax_Val
  PA_KeSMSwRecoveryMdSecRwLtStLtwdRtwdPosMin_Val : Constant  Value=KeSMSwRecoveryMdSecRwLtStLtwdRtwdPosMin_Val
  PA_KeSMSwRecoveryMdSecRwLtStLtwdRtwdPos_Val : Constant  Value=KeSMSwRecoveryMdSecRwLtStLtwdRtwdPos_Val
  PA_KeSMSwRecoveryMdSecRwRtStArmScrnPosMax_Val : Constant  Value=KeSMSwRecoveryMdSecRwRtStArmScrnPosMax_Val
  PA_KeSMSwRecoveryMdSecRwRtStArmScrnPosMin_Val : Constant  Value=KeSMSwRecoveryMdSecRwRtStArmScrnPosMin_Val
  PA_KeSMSwRecoveryMdSecRwRtStArmScrnPos_Val : Constant  Value=KeSMSwRecoveryMdSecRwRtStArmScrnPos_Val
  PA_KeSMSwRecoveryMdSecRwRtStBkReclnUpwdDnwdPosMax_Val : Constant  Value=KeSMSwRecoveryMdSecRwRtStBkReclnUpwdDnwdPosMax_Val
  PA_KeSMSwRecoveryMdSecRwRtStBkReclnUpwdDnwdPosMin_Val : Constant  Value=KeSMSwRecoveryMdSecRwRtStBkReclnUpwdDnwdPosMin_Val
  PA_KeSMSwRecoveryMdSecRwRtStBkReclnUpwdDnwdPos_Val : Constant  Value=KeSMSwRecoveryMdSecRwRtStBkReclnUpwdDnwdPos_Val
  PA_KeSMSwRecoveryMdSecRwRtStFrwdBkwdPosMax_Val : Constant  Value=KeSMSwRecoveryMdSecRwRtStFrwdBkwdPosMax_Val
  PA_KeSMSwRecoveryMdSecRwRtStFrwdBkwdPosMin_Val : Constant  Value=KeSMSwRecoveryMdSecRwRtStFrwdBkwdPosMin_Val
  PA_KeSMSwRecoveryMdSecRwRtStFrwdBkwdPos_Val : Constant  Value=KeSMSwRecoveryMdSecRwRtStFrwdBkwdPos_Val
  PA_KeSMSwRecoveryMdSecRwRtStHdrstUpwdDnwdPosMax_Val : Constant  Value=KeSMSwRecoveryMdSecRwRtStHdrstUpwdDnwdPosMax_Val
  PA_KeSMSwRecoveryMdSecRwRtStHdrstUpwdDnwdPosMin_Val : Constant  Value=KeSMSwRecoveryMdSecRwRtStHdrstUpwdDnwdPosMin_Val
  PA_KeSMSwRecoveryMdSecRwRtStHdrstUpwdDnwdPos_Val : Constant  Value=KeSMSwRecoveryMdSecRwRtStHdrstUpwdDnwdPos_Val
  PA_KeSMSwRecoveryMdSecRwRtStLgrstUpwdDnwdPosMax_Val : Constant  Value=KeSMSwRecoveryMdSecRwRtStLgrstUpwdDnwdPosMax_Val
  PA_KeSMSwRecoveryMdSecRwRtStLgrstUpwdDnwdPosMin_Val : Constant  Value=KeSMSwRecoveryMdSecRwRtStLgrstUpwdDnwdPosMin_Val
  PA_KeSMSwRecoveryMdSecRwRtStLgrstUpwdDnwdPos_Val : Constant  Value=KeSMSwRecoveryMdSecRwRtStLgrstUpwdDnwdPos_Val
  PA_KeSMSwRecoveryMdSecRwRtStLtwdRtwdPosMax_Val : Constant  Value=KeSMSwRecoveryMdSecRwRtStLtwdRtwdPosMax_Val
  PA_KeSMSwRecoveryMdSecRwRtStLtwdRtwdPosMin_Val : Constant  Value=KeSMSwRecoveryMdSecRwRtStLtwdRtwdPosMin_Val
  PA_KeSMSwRecoveryMdSecRwRtStLtwdRtwdPos_Val : Constant  Value=KeSMSwRecoveryMdSecRwRtStLtwdRtwdPos_Val
  PA_KeSMSwRecoveryPassStStFtUpwdDnwdPosMax_Val : Constant  Value=KeSMSwRecoveryPassStStFtUpwdDnwdPosMax_Val
  PA_KeSMSwRecoveryPassStStFtUpwdDnwdPosMin_Val : Constant  Value=KeSMSwRecoveryPassStStFtUpwdDnwdPosMin_Val
  PA_KeSMSwRecoveryPassStStFtUpwdDnwdPos_Val : Constant  Value=KeSMSwRecoveryPassStStFtUpwdDnwdPos_Val
  PA_KeSMSwVIPMDDrvStFtUpwdDnwdPosMax_Val : Constant  Value=KeSMSwVIPMDDrvStFtUpwdDnwdPosMax_Val
  PA_KeSMSwVIPMDDrvStFtUpwdDnwdPosMin_Val : Constant  Value=KeSMSwVIPMDDrvStFtUpwdDnwdPosMin_Val
  PA_KeSMSwVIPMDDrvStFtUpwdDnwdPos_Val : Constant  Value=KeSMSwVIPMDDrvStFtUpwdDnwdPos_Val
  PA_KeSMSwVIPMDPassStStFtUpwdDnwdPosMax_Val : Constant  Value=KeSMSwVIPMDPassStStFtUpwdDnwdPosMax_Val
  PA_KeSMSwVIPMDPassStStFtUpwdDnwdPosMin_Val : Constant  Value=KeSMSwVIPMDPassStStFtUpwdDnwdPosMin_Val
  PA_KeSMSwVIPMDPassStStFtUpwdDnwdPos_Val : Constant  Value=KeSMSwVIPMDPassStStFtUpwdDnwdPos_Val
  PA_KeSMSwVIPSecRwLtStArmScrnPosMax_Val : Constant  Value=KeSMSwVIPSecRwLtStArmScrnPosMax_Val
  PA_KeSMSwVIPSecRwLtStArmScrnPosMin_Val : Constant  Value=KeSMSwVIPSecRwLtStArmScrnPosMin_Val
  PA_KeSMSwVIPSecRwLtStArmScrnPos_Val : Constant  Value=KeSMSwVIPSecRwLtStArmScrnPos_Val
  PA_KeSMSwVIPSecRwLtStBkReclnUpwdDnwdPosMax_Val : Constant  Value=KeSMSwVIPSecRwLtStBkReclnUpwdDnwdPosMax_Val
  PA_KeSMSwVIPSecRwLtStBkReclnUpwdDnwdPosMin_Val : Constant  Value=KeSMSwVIPSecRwLtStBkReclnUpwdDnwdPosMin_Val
  PA_KeSMSwVIPSecRwLtStBkReclnUpwdDnwdPos_Val : Constant  Value=KeSMSwVIPSecRwLtStBkReclnUpwdDnwdPos_Val
  PA_KeSMSwVIPSecRwLtStFrwdBkwdPosMax_Val : Constant  Value=KeSMSwVIPSecRwLtStFrwdBkwdPosMax_Val
  PA_KeSMSwVIPSecRwLtStFrwdBkwdPosMin_Val : Constant  Value=KeSMSwVIPSecRwLtStFrwdBkwdPosMin_Val
  PA_KeSMSwVIPSecRwLtStFrwdBkwdPos_Val : Constant  Value=KeSMSwVIPSecRwLtStFrwdBkwdPos_Val
  PA_KeSMSwVIPSecRwLtStHdrstUpwdPosMax_Val : Constant  Value=KeSMSwVIPSecRwLtStHdrstUpwdPosMax_Val
  PA_KeSMSwVIPSecRwLtStHdrstUpwdPosMin_Val : Constant  Value=KeSMSwVIPSecRwLtStHdrstUpwdPosMin_Val
  PA_KeSMSwVIPSecRwLtStHdrstUpwdPos_Val : Constant  Value=KeSMSwVIPSecRwLtStHdrstUpwdPos_Val
  PA_KeSMSwVIPSecRwLtStLgrstUpwdPosMax_Val : Constant  Value=KeSMSwVIPSecRwLtStLgrstUpwdPosMax_Val
  PA_KeSMSwVIPSecRwLtStLgrstUpwdPosMin_Val : Constant  Value=KeSMSwVIPSecRwLtStLgrstUpwdPosMin_Val
  PA_KeSMSwVIPSecRwLtStLgrstUpwdPos_Val : Constant  Value=KeSMSwVIPSecRwLtStLgrstUpwdPos_Val
  PA_KeSMSwVIPSecRwLtStLtwdRtwdPosMax_Val : Constant  Value=KeSMSwVIPSecRwLtStLtwdRtwdPosMax_Val
  PA_KeSMSwVIPSecRwLtStLtwdRtwdPosMin_Val : Constant  Value=KeSMSwVIPSecRwLtStLtwdRtwdPosMin_Val
  PA_KeSMSwVIPSecRwLtStLtwdRtwdPos_Val : Constant  Value=KeSMSwVIPSecRwLtStLtwdRtwdPos_Val
  PA_KeSMSwVIPSecRwRtStArmScrnPosMax_Val : Constant  Value=KeSMSwVIPSecRwRtStArmScrnPosMax_Val
  PA_KeSMSwVIPSecRwRtStArmScrnPosMin_Val : Constant  Value=KeSMSwVIPSecRwRtStArmScrnPosMin_Val
  PA_KeSMSwVIPSecRwRtStArmScrnPos_Val : Constant  Value=KeSMSwVIPSecRwRtStArmScrnPos_Val
  PA_KeSMSwVIPSecRwRtStBkReclnUpwdDnwdPosMax_Val : Constant  Value=KeSMSwVIPSecRwRtStBkReclnUpwdDnwdPosMax_Val
  PA_KeSMSwVIPSecRwRtStBkReclnUpwdDnwdPosMin_Val : Constant  Value=KeSMSwVIPSecRwRtStBkReclnUpwdDnwdPosMin_Val
  PA_KeSMSwVIPSecRwRtStBkReclnUpwdDnwdPos_Val : Constant  Value=KeSMSwVIPSecRwRtStBkReclnUpwdDnwdPos_Val
  PA_KeSMSwVIPSecRwRtStFrwdBkwdPosMax_Val : Constant  Value=KeSMSwVIPSecRwRtStFrwdBkwdPosMax_Val
  PA_KeSMSwVIPSecRwRtStFrwdBkwdPosMin_Val : Constant  Value=KeSMSwVIPSecRwRtStFrwdBkwdPosMin_Val
  PA_KeSMSwVIPSecRwRtStFrwdBkwdPos_Val : Constant  Value=KeSMSwVIPSecRwRtStFrwdBkwdPos_Val
  PA_KeSMSwVIPSecRwRtStHdrstUpwdPosMax_Val : Constant  Value=KeSMSwVIPSecRwRtStHdrstUpwdPosMax_Val
  PA_KeSMSwVIPSecRwRtStHdrstUpwdPosMin_Val : Constant  Value=KeSMSwVIPSecRwRtStHdrstUpwdPosMin_Val
  PA_KeSMSwVIPSecRwRtStHdrstUpwdPos_Val : Constant  Value=KeSMSwVIPSecRwRtStHdrstUpwdPos_Val
  PA_KeSMSwVIPSecRwRtStLgrstUpwdPosMax_Val : Constant  Value=KeSMSwVIPSecRwRtStLgrstUpwdPosMax_Val
  PA_KeSMSwVIPSecRwRtStLgrstUpwdPosMin_Val : Constant  Value=KeSMSwVIPSecRwRtStLgrstUpwdPosMin_Val
  PA_KeSMSwVIPSecRwRtStLgrstUpwdPos_Val : Constant  Value=KeSMSwVIPSecRwRtStLgrstUpwdPos_Val
  PA_KeSMSwVIPSecRwRtStLtwdRtwdPosMax_Val : Constant  Value=KeSMSwVIPSecRwRtStLtwdRtwdPosMax_Val
  PA_KeSMSwVIPSecRwRtStLtwdRtwdPosMin_Val : Constant  Value=KeSMSwVIPSecRwRtStLtwdRtwdPosMin_Val
  PA_KeSMSwVIPSecRwRtStLtwdRtwdPos_Val : Constant  Value=KeSMSwVIPSecRwRtStLtwdRtwdPos_Val
  PA_KeSMSwVIPThdRwLtStBkReclnUpwdDnwdPosMax_Val : Constant  Value=KeSMSwVIPThdRwLtStBkReclnUpwdDnwdPosMax_Val
  PA_KeSMSwVIPThdRwLtStBkReclnUpwdDnwdPosMin_Val : Constant  Value=KeSMSwVIPThdRwLtStBkReclnUpwdDnwdPosMin_Val
  PA_KeSMSwVIPThdRwLtStBkReclnUpwdDnwdPos_Val : Constant  Value=KeSMSwVIPThdRwLtStBkReclnUpwdDnwdPos_Val
  PA_KeSMSwVIPThdRwLtStCshnFldUpwdDnwdPosMax_Val : Constant  Value=KeSMSwVIPThdRwLtStCshnFldUpwdDnwdPosMax_Val
  PA_KeSMSwVIPThdRwLtStCshnFldUpwdDnwdPosMin_Val : Constant  Value=KeSMSwVIPThdRwLtStCshnFldUpwdDnwdPosMin_Val
  PA_KeSMSwVIPThdRwLtStCshnFldUpwdDnwdPos_Val : Constant  Value=KeSMSwVIPThdRwLtStCshnFldUpwdDnwdPos_Val
  PA_KeSMSwVIPThdRwLtStFrwdBkwdPosMax_Val : Constant  Value=KeSMSwVIPThdRwLtStFrwdBkwdPosMax_Val
  PA_KeSMSwVIPThdRwLtStFrwdBkwdPosMin_Val : Constant  Value=KeSMSwVIPThdRwLtStFrwdBkwdPosMin_Val
  PA_KeSMSwVIPThdRwLtStFrwdBkwdPos_Val : Constant  Value=KeSMSwVIPThdRwLtStFrwdBkwdPos_Val
  PA_KeSMSwVIPThdRwRtStBkReclnUpwdDnwdPosMax_Val : Constant  Value=KeSMSwVIPThdRwRtStBkReclnUpwdDnwdPosMax_Val
  PA_KeSMSwVIPThdRwRtStBkReclnUpwdDnwdPosMin_Val : Constant  Value=KeSMSwVIPThdRwRtStBkReclnUpwdDnwdPosMin_Val
  PA_KeSMSwVIPThdRwRtStBkReclnUpwdDnwdPos_Val : Constant  Value=KeSMSwVIPThdRwRtStBkReclnUpwdDnwdPos_Val
  PA_KeSMSwVIPThdRwRtStCshnFldUpwdDnwdPosMax_Val : Constant  Value=KeSMSwVIPThdRwRtStCshnFldUpwdDnwdPosMax_Val
  PA_KeSMSwVIPThdRwRtStCshnFldUpwdDnwdPosMin_Val : Constant  Value=KeSMSwVIPThdRwRtStCshnFldUpwdDnwdPosMin_Val
  PA_KeSMSwVIPThdRwRtStCshnFldUpwdDnwdPos_Val : Constant  Value=KeSMSwVIPThdRwRtStCshnFldUpwdDnwdPos_Val
  PA_KeSMSwVIPThdRwRtStFrwdBkwdPosMax_Val : Constant  Value=KeSMSwVIPThdRwRtStFrwdBkwdPosMax_Val
  PA_KeSMSwVIPThdRwRtStFrwdBkwdPosMin_Val : Constant  Value=KeSMSwVIPThdRwRtStFrwdBkwdPosMin_Val
  PA_KeSMSwVIPThdRwRtStFrwdBkwdPos_Val : Constant  Value=KeSMSwVIPThdRwRtStFrwdBkwdPos_Val
  ModeStCalib : Outport
  wires:
  PA_KeSMSwAcsEntryDrvStBkReclnUpwdDnwdPosMax_Val/1 -> Bus Creator/2  "BkReclnUpwdDnwdPosMax"
  PA_KeSMSwAcsEntryDrvStBkReclnUpwdDnwdPosMin_Val/1 -> Bus Creator/3  "BkReclnUpwdDnwdPosMin"
  PA_KeSMSwAcsEntryDrvStBkReclnUpwdDnwdPos_Val/1 -> Bus Creator/1  "BkReclnUpwdDnwdPos"
  PA_KeSMSwAcsEntryDrvStFtUpwdDnwdPosMax_Val/1 -> Bus Creator/8  "FtUpwdDnwdPosMax"
  PA_KeSMSwAcsEntryDrvStFtUpwdDnwdPosMin_Val/1 -> Bus Creator/9  "FtUpwdDnwdPosMin"
  PA_KeSMSwAcsEntryDrvStFrwdBkwdPosMax_Val/1 -> Bus Creator/5  "FrwdBkwdPosMax"
  PA_KeSMSwAcsEntryDrvStFrwdBkwdPosMin_Val/1 -> Bus Creator/6  "FrwdBkwdPosMin"
  PA_KeSMSwAcsEntryDrvStFrwdBkwdPos_Val/1 -> Bus Creator/4  "FrwdBkwdPos"
  PA_KeSMSwAcsEntryDrvStFtUpwdDnwdPos_Val/1 -> Bus Creator/7  "FtUpwdDnwdPos"
  Bus Creator/1 -> Bus Creator1/1  "AcsEntryDrvSt"
  PA_KeSMSwAcsExtDrvStBkReclnUpwdDnwdPosMax_Val/1 -> Bus Creator2/2  "BkReclnUpwdDnwdPosMax"
  PA_KeSMSwAcsExtDrvStBkReclnUpwdDnwdPosMin_Val/1 -> Bus Creator2/3  "BkReclnUpwdDnwdPosMin"
  PA_KeSMSwAcsExtDrvStBkReclnUpwdDnwdPos_Val/1 -> Bus Creator2/1  "BkReclnUpwdDnwdPos"
  PA_KeSMSwAcsExtDrvStFtUpwdDnwdPosMax_Val/1 -> Bus Creator2/8  "FtUpwdDnwdPosMax"
  PA_KeSMSwAcsExtDrvStFtUpwdDnwdPosMin_Val/1 -> Bus Creator2/9  "FtUpwdDnwdPosMin"
  PA_KeSMSwAcsExtDrvStFrwdBkwdPosMax_Val/1 -> Bus Creator2/5  "FrwdBkwdPosMax"
  PA_KeSMSwAcsExtDrvStFrwdBkwdPosMin_Val/1 -> Bus Creator2/6  "FrwdBkwdPosMin"
  PA_KeSMSwAcsExtDrvStFtUpwdDnwdPos_Val/1 -> Bus Creator2/7  "FtUpwdDnwdPos"
  PA_KeSMSwAcsExtDrvStFrwdBkwdPos_Val/1 -> Bus Creator2/4  "FrwdBkwdPos"
  Bus Creator2/1 -> Bus Creator1/2  "AcsExtDrvSt"
  PA_KeSMSwAcsEntryPassStBkReclnUpwdDnwdPosMin_Val/1 -> Bus Creator3/3  "BkReclnUpwdDnwdPosMin"
  PA_KeSMSwAcsEntryPassStBkReclnUpwdDnwdPosMax_Val/1 -> Bus Creator3/2  "BkReclnUpwdDnwdPosMax"
  PA_KeSMSwAcsEntryPassStBkReclnUpwdDnwdPos_Val/1 -> Bus Creator3/1  "BkReclnUpwdDnwdPos"
  PA_KeSMSwAcsEntryPassStFtUpwdDnwdPosMiax_Val/1 -> Bus Creator3/8  "FtUpwdDnwdPosMax"
  PA_KeSMSwAcsEntryPassStFtUpwdDnwdPosMin_Val/1 -> Bus Creator3/9  "FtUpwdDnwdPosMin"
  PA_KeSMSwAcsEntryPassStFrwdBkwdPosMax_Val/1 -> Bus Creator3/5  "FrwdBkwdPosMax"
  PA_KeSMSwAcsEntryPassStFrwdBkwdPosMin_Val/1 -> Bus Creator3/6  "FrwdBkwdPosMin"
  PA_KeSMSwAcsEntryPassStFtUpwdDnwdPos_Val/1 -> Bus Creator3/7  "FtUpwdDnwdPos"
  PA_KeSMSwAcsEntryPassStFrwdBkwdPos_Val/1 -> Bus Creator3/4  "FrwdBkwdPos"
  PA_KeSMSwAcsExtPassStBkReclnUpwdDnwdPosMax_Val/1 -> Bus Creator4/2  "BkReclnUpwdDnwdPosMax"
  PA_KeSMSwAcsExtPassStBkReclnUpwdDnwdPosMin_Val/1 -> Bus Creator4/3  "BkReclnUpwdDnwdPosMin"
  PA_KeSMSwAcsExtPassStBkReclnUpwdDnwdPos_Val/1 -> Bus Creator4/1  "BkReclnUpwdDnwdPos"
  PA_KeSMSwAcsExtPassStFtUpwdDnwdPosMax_Val/1 -> Bus Creator4/8  "FtUpwdDnwdPosMax"
  PA_KeSMSwAcsExtPassStFtUpwdDnwdPosMin_Val/1 -> Bus Creator4/9  "FtUpwdDnwdPosMin"
  PA_KeSMSwAcsExtPassStFrwdBkwdPosMax_Val/1 -> Bus Creator4/5  "FrwdBkwdPosMax"
  PA_KeSMSwAcsExtPassStFrwdBkwdPosMin_Val/1 -> Bus Creator4/6  "FrwdBkwdPosMin"
  PA_KeSMSwAcsExtPassStFtUpwdDnwdPos_Val/1 -> Bus Creator4/7  "FtUpwdDnwdPos"
  PA_KeSMSwAcsExtPassStFrwdBkwdPos_Val/1 -> Bus Creator4/4  "FrwdBkwdPos"
  Bus Creator4/1 -> Bus Creator5/2  "AcsExtPassSt"
  Bus Creator3/1 -> Bus Creator5/1  "AcsEntryPassSt"
  PA_KeSMSwAcsEntrySecRwLtStBkReclnUpwdDnwdPosMax_Val/1 -> Bus Creator6/5  "BkReclnUpwdDnwdPosMax"
  PA_KeSMSwAcsEntrySecRwLtStBkReclnUpwdDnwdPosMin_Val/1 -> Bus Creator6/6  "BkReclnUpwdDnwdPosMin"
  PA_KeSMSwAcsEntrySecRwLtStBkReclnUpwdDnwdPos_Val/1 -> Bus Creator6/4  "BkReclnUpwdDnwdPos"
  PA_KeSMSwAcsEntrySecRwLtStArmScrnPosMax_Val/1 -> Bus Creator6/2  "ArmScrnPosMax"
  PA_KeSMSwAcsEntrySecRwLtStArmScrnPosMin_Val/1 -> Bus Creator6/3  "ArmScrnPosMin"
  PA_KeSMSwAcsEntrySecRwLtStHdrstUpwdPosMax_Val/1 -> Bus Creator6/11  "HdrstUpwdPosMax"
  PA_KeSMSwAcsEntrySecRwLtStHdrstUpwdPosMin_Val/1 -> Bus Creator6/12  "HdrstUpwdPosMin"
  PA_KeSMSwAcsEntrySecRwLtStFrwdBkwdPosMax_Val/1 -> Bus Creator6/8  "FrwdBkwdPosMax"
  PA_KeSMSwAcsEntrySecRwLtStFrwdBkwdPosMin_Val/1 -> Bus Creator6/9  "FrwdBkwdPosMin"
  PA_KeSMSwAcsEntrySecRwLtStLgrstUpwdPosMax_Val/1 -> Bus Creator6/14  "LgrstUpwdPosMax"
  PA_KeSMSwAcsEntrySecRwLtStLgrstUpwdPosMin_Val/1 -> Bus Creator6/15  "LgrstUpwdPosMin"
  PA_KeSMSwAcsEntrySecRwLtStArmScrnPos_Val/1 -> Bus Creator6/1  "ArmScrnPos"
  PA_KeSMSwAcsEntrySecRwLtStFrwdBkwdPos_Val/1 -> Bus Creator6/7  "FrwdBkwdPos"
  PA_KeSMSwAcsEntrySecRwLtStHdrstUpwdPos_Val/1 -> Bus Creator6/10  "HdrstUpwdPos"
  PA_KeSMSwAcsEntrySecRwLtStLtwdRtwdPosMax_Val/1 -> Bus Creator6/17  "LtwdRtwdPosMax"
  PA_KeSMSwAcsEntrySecRwLtStLgrstUpwdPos_Val/1 -> Bus Creator6/13  "LgrstUpwdPos"
  PA_KeSMSwAcsEntrySecRwLtStLtwdRtwdPosMin_Val/1 -> Bus Creator6/18  "LtwdRtwdPosMin"
  PA_KeSMSwAcsEntrySecRwLtStLtwdRtwdPos_Val/1 -> Bus Creator6/16  "LtwdRtwdPos"
  PA_KeSMSwAcsExtSecRwLtStBkReclnUpwdDnwdPos_Val/1 -> Bus Creator7/4  "BkReclnUpwdDnwdPos"
  PA_KeSMSwAcsExtSecRwLtStBkReclnUpwdDnwdPosMin_Val/1 -> Bus Creator7/6  "BkReclnUpwdDnwdPosMin"
  PA_KeSMSwAcsExtSecRwLtStBkReclnUpwdDnwdPosMax_Val/1 -> Bus Creator7/5  "BkReclnUpwdDnwdPosMax"
  PA_KeSMSwDltTrgtPos_Val2/1 -> Bus Creator7/12  "HdrstUpwdPosMin"
  PA_KeSMSwAcsExtSecRwLtStArmScrnPosMin_Val/1 -> Bus Creator7/3  "ArmScrnPosMin"
  PA_KeSMSwAcsExtSecRwLtStLtwdRtwdPos_Val/1 -> Bus Creator7/16  "LtwdRtwdPos"
  PA_KeSMSwAcsExtSecRwLtStArmScrnPosMax_Val/1 -> Bus Creator7/2  "ArmScrnPosMax"
  PA_KeSMSwAcsExtSecRwLtStLtwdRtwdPosMin_Val/1 -> Bus Creator7/18  "LtwdRtwdPosMin"
  PA_KeSMSwAcsExtSecRwLtStLgrstUpwdDnwdPos_Val/1 -> Bus Creator7/13  "LgrstUpwdPos"
  PA_KeSMSwAcsExtSecRwLtStLtwdRtwdPosMax_Val/1 -> Bus Creator7/17  "LtwdRtwdPosMax"
  PA_KeSMSwAcsExtSecRwLtStArmScrnPos_Val/1 -> Bus Creator7/1  "ArmScrnPos"
  PA_KeSMSwDltTrgtPos_Val12/1 -> Bus Creator7/10  "HdrstUpwdPos"
  PA_KeSMSwAcsExtSecRwLtStLgrstUpwdDnwdPosMax_Val/1 -> Bus Creator7/14  "LgrstUpwdPosMax"
  PA_KeSMSwAcsExtSecRwLtStFrwdBkwdPosMin_Val/1 -> Bus Creator7/9  "FrwdBkwdPosMin"
  PA_KeSMSwAcsExtSecRwLtStFrwdBkwdPos_Val/1 -> Bus Creator7/7  "FrwdBkwdPos"
  PA_KeSMSwDltTrgtPos_Val1/1 -> Bus Creator7/11  "HdrstUpwdPosMax"
  PA_KeSMSwAcsExtSecRwLtStFrwdBkwdPosMax_Val/1 -> Bus Creator7/8  "FrwdBkwdPosMax"
  PA_KeSMSwAcsExtSecRwLtStLgrstUpwdDnwdPosMin_Val/1 -> Bus Creator7/15  "LgrstUpwdPosMin"
  PA_KeSMSwRecoveryMdSecRwLtStHdrstUpwdDnwdPos_Val/1 -> Bus Creator8/10  "HdrstUpwdPos"
  PA_KeSMSwRecoveryMdSecRwLtStBkReclnUpwdDnwdPos_Val/1 -> Bus Creator8/4  "BkReclnUpwdDnwdPos"
  PA_KeSMSwRecoveryMdSecRwLtStFrwdBkwdPos_Val/1 -> Bus Creator8/7  "FrwdBkwdPos"
  PA_KeSMSwRecoveryMdSecRwLtStArmScrnPosMin_Val/1 -> Bus Creator8/3  "ArmScrnPosMin"
  PA_KeSMSwRecoveryMdSecRwLtStLgrstUpwdDnwdPos_Val/1 -> Bus Creator8/13  "LgrstUpwdPos"
  PA_KeSMSwRecoveryMdSecRwLtStHdrstUpwdDnwdPosMin_Val/1 -> Bus Creator8/12  "HdrstUpwdPosMin"
  PA_KeSMSwRecoveryMdSecRwLtStHdrstUpwdDnwdPosMax_Val/1 -> Bus Creator8/11  "HdrstUpwdPosMax"
  PA_KeSMSwRecoveryMdSecRwLtStArmScrnPos_Val/1 -> Bus Creator8/1  "ArmScrnPos"
  PA_KeSMSwRecoveryMdSecRwLtStFrwdBkwdPosMax_Val/1 -> Bus Creator8/8  "FrwdBkwdPosMax"
  PA_KeSMSwRecoveryMdSecRwLtStLtwdRtwdPosMax_Val/1 -> Bus Creator8/17  "LtwdRtwdPosMax"
  PA_KeSMSwRecoveryMdSecRwLtStBkReclnUpwdDnwdPosMin_Val/1 -> Bus Creator8/6  "BkReclnUpwdDnwdPosMin"
  PA_KeSMSwRecoveryMdSecRwLtStArmScrnPosMax_Val/1 -> Bus Creator8/2  "ArmScrnPosMax"
  PA_KeSMSwRecoveryMdSecRwLtStBkReclnUpwdDnwdPosMax_Val/1 -> Bus Creator8/5  "BkReclnUpwdDnwdPosMax"
  PA_KeSMSwRecoveryMdSecRwLtStLgrstUpwdDnwdPosMax_Val/1 -> Bus Creator8/14  "LgrstUpwdPosMax"
  PA_KeSMSwRecoveryMdSecRwLtStLtwdRtwdPosMin_Val/1 -> Bus Creator8/18  "LtwdRtwdPosMin"
  PA_KeSMSwRecoveryMdSecRwLtStFrwdBkwdPosMin_Val/1 -> Bus Creator8/9  "FrwdBkwdPosMin"
  PA_KeSMSwRecoveryMdSecRwLtStLgrstUpwdDnwdPosMin_Val/1 -> Bus Creator8/15  "LgrstUpwdPosMin"
  PA_KeSMSwRecoveryMdSecRwLtStLtwdRtwdPos_Val/1 -> Bus Creator8/16  "LtwdRtwdPos"
  PA_KeSMSwVIPSecRwLtStHdrstUpwdPos_Val/1 -> Bus Creator9/10  "HdrstUpwdPos"
  PA_KeSMSwVIPSecRwLtStLtwdRtwdPosMin_Val/1 -> Bus Creator9/18  "LtwdRtwdPosMin"
  PA_KeSMSwVIPSecRwLtStLgrstUpwdPosMin_Val/1 -> Bus Creator9/15  "LgrstUpwdPosMin"
  PA_KeSMSwVIPSecRwLtStLtwdRtwdPosMax_Val/1 -> Bus Creator9/17  "LtwdRtwdPosMax"
  PA_KeSMSwVIPSecRwLtStHdrstUpwdPosMax_Val/1 -> Bus Creator9/11  "HdrstUpwdPosMax"
  PA_KeSMSwVIPSecRwLtStHdrstUpwdPosMin_Val/1 -> Bus Creator9/12  "HdrstUpwdPosMin"
  PA_KeSMSwVIPSecRwLtStLgrstUpwdPos_Val/1 -> Bus Creator9/13  "LgrstUpwdPos"
  PA_KeSMSwVIPSecRwLtStFrwdBkwdPosMax_Val/1 -> Bus Creator9/8  "FrwdBkwdPosMax"
  PA_KeSMSwVIPSecRwLtStFrwdBkwdPos_Val/1 -> Bus Creator9/7  "FrwdBkwdPos"
  PA_KeSMSwVIPSecRwLtStArmScrnPosMin_Val/1 -> Bus Creator9/3  "ArmScrnPosMin"
  PA_KeSMSwVIPSecRwLtStFrwdBkwdPosMin_Val/1 -> Bus Creator9/9  "FrwdBkwdPosMin"
  PA_KeSMSwVIPSecRwLtStLgrstUpwdPosMax_Val/1 -> Bus Creator9/14  "LgrstUpwdPosMax"
  PA_KeSMSwVIPSecRwLtStBkReclnUpwdDnwdPosMax_Val/1 -> Bus Creator9/5  "BkReclnUpwdDnwdPosMax"
  PA_KeSMSwVIPSecRwLtStArmScrnPosMax_Val/1 -> Bus Creator9/2  "ArmScrnPosMax"
  PA_KeSMSwVIPSecRwLtStBkReclnUpwdDnwdPosMin_Val/1 -> Bus Creator9/6  "BkReclnUpwdDnwdPosMin"
  PA_KeSMSwVIPSecRwLtStLtwdRtwdPos_Val/1 -> Bus Creator9/16  "LtwdRtwdPos"
  PA_KeSMSwVIPSecRwLtStArmScrnPos_Val/1 -> Bus Creator9/1  "ArmScrnPos"
  PA_KeSMSwVIPSecRwLtStBkReclnUpwdDnwdPos_Val/1 -> Bus Creator9/4  "BkReclnUpwdDnwdPos"
  PA_KeSMSwAcsEntrySecRwRtStBkReclnUpwdDnwdPos_Val/1 -> Bus Creator10/4  "BkReclnUpwdDnwdPos"
  PA_KeSMSwAcsEntrySecRwRtStBkReclnUpwdDnwdPosMin_Val/1 -> Bus Creator10/6  "BkReclnUpwdDnwdPosMin"
  PA_KeSMSwAcsEntrySecRwRtStBkReclnUpwdDnwdPosMax_Val/1 -> Bus Creator10/5  "BkReclnUpwdDnwdPosMax"
  PA_KeSMSwAcsEntrySecRwRtStHdrstUpwdPosMin_Val/1 -> Bus Creator10/12  "HdrstUpwdPosMin"
  PA_KeSMSwAcsEntrySecRwRtStArmScrnPosMin_Val/1 -> Bus Creator10/3  "ArmScrnPosMin"
  PA_KeSMSwAcsEntrySecRwRtStLtwdRtwdPos_Val/1 -> Bus Creator10/16  "LtwdRtwdPos"
  PA_KeSMSwAcsEntrySecRwRtStArmScrnPosMax_Val/1 -> Bus Creator10/2  "ArmScrnPosMax"
  PA_KeSMSwAcsEntrySecRwRtStLtwdRtwdPosMin_Val/1 -> Bus Creator10/18  "LtwdRtwdPosMin"
  PA_KeSMSwAcsEntrySecRwRtStLgrstUpwdPos_Val/1 -> Bus Creator10/13  "LgrstUpwdPos"
  PA_KeSMSwAcsEntrySecRwRtStLtwdRtwdPosMax_Val/1 -> Bus Creator10/17  "LtwdRtwdPosMax"
  PA_KeSMSwAcsEntrySecRwRtStArmScrnPos_Val/1 -> Bus Creator10/1  "ArmScrnPos"
  PA_KeSMSwAcsEntrySecRwRtStHdrstUpwdPos_Val/1 -> Bus Creator10/10  "HdrstUpwdPos"
  PA_KeSMSwAcsEntrySecRwRtStLgrstUpwdPosMax_Val/1 -> Bus Creator10/14  "LgrstUpwdPosMax"
  PA_KeSMSwAcsEntrySecRwRtStFrwdBkwdPosMin_Val/1 -> Bus Creator10/9  "FrwdBkwdPosMin"
  PA_KeSMSwAcsEntrySecRwRtStFrwdBkwdPos_Val/1 -> Bus Creator10/7  "FrwdBkwdPos"
  PA_KeSMSwAcsEntrySecRwRtStHdrstUpwdPosMax_Val/1 -> Bus Creator10/11  "HdrstUpwdPosMax"
  PA_KeSMSwAcsEntrySecRwRtStFrwdBkwdPosMax_Val/1 -> Bus Creator10/8  "FrwdBkwdPosMax"
  PA_KeSMSwAcsEntrySecRwRtStLgrstUpwdPosMin_Val/1 -> Bus Creator10/15  "LgrstUpwdPosMin"
  PA_KeSMSwAcsExtSecRwRtStLtwdRtwdPosMax_Val/1 -> Bus Creator11/17  "LtwdRtwdPosMax"
  PA_KeSMSwAcsExtSecRwRtStLtwdRtwdPosMin_Val/1 -> Bus Creator11/18  "LtwdRtwdPosMin"
  PA_KeSMSwAcsExtSecRwRtStLtwdRtwdPos_Val/1 -> Bus Creator11/16  "LtwdRtwdPos"
  PA_KeSMSwDltTrgtPos_Val3/1 -> Bus Creator11/11  "HdrstUpwdPosMax"
  PA_KeSMSwAcsExtSecRwRtStFrwdBkwdPos_Val/1 -> Bus Creator11/7  "FrwdBkwdPos"
  PA_KeSMSwAcsExtSecRwRtStLgrstUpwdDnwdPosMax_Val/1 -> Bus Creator11/14  "LgrstUpwdPosMax"
  PA_KeSMSwAcsExtSecRwRtStLgrstUpwdDnwdPos_Val/1 -> Bus Creator11/13  "LgrstUpwdPos"
  PA_KeSMSwAcsExtSecRwRtStBkReclnUpwdDnwdPos_Val/1 -> Bus Creator11/4  "BkReclnUpwdDnwdPos"
  PA_KeSMSwAcsExtSecRwRtStArmScrnPosMax_Val/1 -> Bus Creator11/2  "ArmScrnPosMax"
  PA_KeSMSwAcsExtSecRwRtStFrwdBkwdPosMin_Val/1 -> Bus Creator11/9  "FrwdBkwdPosMin"
  PA_KeSMSwAcsExtSecRwRtStLgrstUpwdDnwdPosMin_Val/1 -> Bus Creator11/15  "LgrstUpwdPosMin"
  PA_KeSMSwDltTrgtPos_Val4/1 -> Bus Creator11/10  "HdrstUpwdPos"
  PA_KeSMSwAcsExtSecRwRtStArmScrnPosMin_Val/1 -> Bus Creator11/3  "ArmScrnPosMin"
  PA_KeSMSwDltTrgtPos_Val5/1 -> Bus Creator11/12  "HdrstUpwdPosMin"
  PA_KeSMSwAcsExtSecRwRtStBkReclnUpwdDnwdPosMax_Val/1 -> Bus Creator11/5  "BkReclnUpwdDnwdPosMax"
  PA_KeSMSwAcsExtSecRwRtStFrwdBkwdPosMax_Val/1 -> Bus Creator11/8  "FrwdBkwdPosMax"
  PA_KeSMSwAcsExtSecRwRtStBkReclnUpwdDnwdPosMin_Val/1 -> Bus Creator11/6  "BkReclnUpwdDnwdPosMin"
  PA_KeSMSwAcsExtSecRwRtStArmScrnPos_Val/1 -> Bus Creator11/1  "ArmScrnPos"
  PA_KeSMSwRecoveryMdSecRwRtStBkReclnUpwdDnwdPosMin_Val/1 -> Bus Creator12/6  "BkReclnUpwdDnwdPosMin"
  PA_KeSMSwRecoveryMdSecRwRtStLgrstUpwdDnwdPosMin_Val/1 -> Bus Creator12/15  "LgrstUpwdPosMin"
  PA_KeSMSwRecoveryMdSecRwRtStLgrstUpwdDnwdPosMax_Val/1 -> Bus Creator12/14  "LgrstUpwdPosMax"
  PA_KeSMSwRecoveryMdSecRwRtStFrwdBkwdPos_Val/1 -> Bus Creator12/7  "FrwdBkwdPos"
  PA_KeSMSwRecoveryMdSecRwRtStLtwdRtwdPosMin_Val/1 -> Bus Creator12/18  "LtwdRtwdPosMin"
  PA_KeSMSwRecoveryMdSecRwRtStFrwdBkwdPosMax_Val/1 -> Bus Creator12/8  "FrwdBkwdPosMax"
  PA_KeSMSwRecoveryMdSecRwRtStLtwdRtwdPos_Val/1 -> Bus Creator12/16  "LtwdRtwdPos"
  PA_KeSMSwRecoveryMdSecRwRtStArmScrnPos_Val/1 -> Bus Creator12/1  "ArmScrnPos"
  PA_KeSMSwRecoveryMdSecRwRtStHdrstUpwdDnwdPosMax_Val/1 -> Bus Creator12/11  "HdrstUpwdPosMax"
  PA_KeSMSwRecoveryMdSecRwRtStBkReclnUpwdDnwdPos_Val/1 -> Bus Creator12/4  "BkReclnUpwdDnwdPos"
  PA_KeSMSwRecoveryMdSecRwRtStLtwdRtwdPosMax_Val/1 -> Bus Creator12/17  "LtwdRtwdPosMax"
  PA_KeSMSwRecoveryMdSecRwRtStLgrstUpwdDnwdPos_Val/1 -> Bus Creator12/13  "LgrstUpwdPos"
  PA_KeSMSwRecoveryMdSecRwRtStFrwdBkwdPosMin_Val/1 -> Bus Creator12/9  "FrwdBkwdPosMin"
  PA_KeSMSwRecoveryMdSecRwRtStBkReclnUpwdDnwdPosMax_Val/1 -> Bus Creator12/5  "BkReclnUpwdDnwdPosMax"
  PA_KeSMSwRecoveryMdSecRwRtStArmScrnPosMin_Val/1 -> Bus Creator12/3  "ArmScrnPosMin"
  PA_KeSMSwRecoveryMdSecRwRtStHdrstUpwdDnwdPos_Val/1 -> Bus Creator12/10  "HdrstUpwdPos"
  PA_KeSMSwRecoveryMdSecRwRtStHdrstUpwdDnwdPosMin_Val/1 -> Bus Creator12/12  "HdrstUpwdPosMin"
  PA_KeSMSwRecoveryMdSecRwRtStArmScrnPosMax_Val/1 -> Bus Creator12/2  "ArmScrnPosMax"
  PA_KeSMSwVIPSecRwRtStHdrstUpwdPos_Val/1 -> Bus Creator13/10  "HdrstUpwdPos"
  PA_KeSMSwVIPSecRwRtStHdrstUpwdPosMax_Val/1 -> Bus Creator13/11  "HdrstUpwdPosMax"
  PA_KeSMSwVIPSecRwRtStHdrstUpwdPosMin_Val/1 -> Bus Creator13/12  "HdrstUpwdPosMin"
  PA_KeSMSwVIPSecRwRtStLgrstUpwdPosMax_Val/1 -> Bus Creator13/14  "LgrstUpwdPosMax"
  PA_KeSMSwVIPSecRwRtStLtwdRtwdPosMin_Val/1 -> Bus Creator13/18  "LtwdRtwdPosMin"
  PA_KeSMSwVIPSecRwRtStFrwdBkwdPosMax_Val/1 -> Bus Creator13/8  "FrwdBkwdPosMax"
  PA_KeSMSwVIPSecRwRtStBkReclnUpwdDnwdPos_Val/1 -> Bus Creator13/4  "BkReclnUpwdDnwdPos"
  PA_KeSMSwVIPSecRwRtStFrwdBkwdPos_Val/1 -> Bus Creator13/7  "FrwdBkwdPos"
  PA_KeSMSwVIPSecRwRtStFrwdBkwdPosMin_Val/1 -> Bus Creator13/9  "FrwdBkwdPosMin"
  PA_KeSMSwVIPSecRwRtStArmScrnPos_Val/1 -> Bus Creator13/1  "ArmScrnPos"
  PA_KeSMSwVIPSecRwRtStArmScrnPosMin_Val/1 -> Bus Creator13/3  "ArmScrnPosMin"
  PA_KeSMSwVIPSecRwRtStLtwdRtwdPosMax_Val/1 -> Bus Creator13/17  "LtwdRtwdPosMax"
  PA_KeSMSwVIPSecRwRtStLgrstUpwdPos_Val/1 -> Bus Creator13/13  "LgrstUpwdPos"
  PA_KeSMSwVIPSecRwRtStArmScrnPosMax_Val/1 -> Bus Creator13/2  "ArmScrnPosMax"
  PA_KeSMSwVIPSecRwRtStBkReclnUpwdDnwdPosMin_Val/1 -> Bus Creator13/6  "BkReclnUpwdDnwdPosMin"
  PA_KeSMSwVIPSecRwRtStLgrstUpwdPosMin_Val/1 -> Bus Creator13/15  "LgrstUpwdPosMin"
  PA_KeSMSwVIPSecRwRtStLtwdRtwdPos_Val/1 -> Bus Creator13/16  "LtwdRtwdPos"
  PA_KeSMSwVIPSecRwRtStBkReclnUpwdDnwdPosMax_Val/1 -> Bus Creator13/5  "BkReclnUpwdDnwdPosMax"
  StNumConfig/1 -> [IfKeSMSeStNumConfig_Val]
  [IfKeSMSeStNumConfig_Val] -> Multiport Switch6/1
  Bus Creator5/1 -> Multiport Switch6/4, Multiport Switch6/2
  Multiport Switch6/1 -> [Calib_Pass]
  Multiport Switch1/1 -> [Calib_Drv]
  Bus Creator1/1 -> Multiport Switch1/2, Multiport Switch1/4
  [IfKeSMSeStNumConfig_Val] -> Multiport Switch1/1
  Bus Creator6/1 -> Bus Creator14/1  "AcsEntrySecRwLtSt"
  Bus Creator7/1 -> Bus Creator14/2  "AcsExtSecRwLtSt"
  Bus Creator8/1 -> Bus Creator14/3  "RecoveryMdSecRwLtSt"
  Bus Creator9/1 -> Bus Creator14/4  "VIPSecRwLtSt"
  Bus Creator14/1 -> Multiport Switch2/2, Multiport Switch2/4
  [IfKeSMSeStNumConfig_Val] -> Multiport Switch2/1
  Bus Creator15/1 -> Multiport Switch7/2, Multiport Switch7/4
  Bus Creator11/1 -> Bus Creator15/2  "AcsExtSecRwRSt"
  Bus Creator10/1 -> Bus Creator15/1  "AcsEntrySecRwRtSt"
  Bus Creator12/1 -> Bus Creator15/3  "RecoveryMdSecRwRtSt"
  Bus Creator13/1 -> Bus Creator15/4  "VIPSecRwRtSt"
  [IfKeSMSeStNumConfig_Val] -> Multiport Switch7/1
  PA_KeSMSwAcsEntryThdRwLtStCshnFldUpwdDnwdPosMin_Val/1 -> Bus Creator16/6  "CshnFldUpwdDnwdPosMin"
  PA_KeSMSwAcsEntryThdRwLtStCshnFldUpwdDnwdPosMax_Val/1 -> Bus Creator16/5  "CshnFldUpwdDnwdPosMax"
  PA_KeSMSwAcsEntryThdRwLtStBkReclnUpwdDnwdPosMin_Val/1 -> Bus Creator16/3  "BkReclnUpwdDnwdPosMin"
  PA_KeSMSwAcsEntryThdRwLtStBkReclnUpwdDnwdPosMax_Val/1 -> Bus Creator16/2  "BkReclnUpwdDnwdPosMax"
  PA_KeSMSwAcsEntryThdRwLtStCshnFldUpwdDnwdPos_Val/1 -> Bus Creator16/4  "CshnFldUpwdDnwdPos"
  PA_KeSMSwAcsEntryThdRwLtStBkReclnUpwdDnwdPos_Val/1 -> Bus Creator16/1  "BkReclnUpwdDnwdPos"
  PA_KeSMSwAcsEntryThdRwLtStFrwdBkwdPosMax_Val/1 -> Bus Creator16/8  "FrwdBkwdPosMax"
  PA_KeSMSwAcsEntryThdRwLtStFrwdBkwdPosMin_Val/1 -> Bus Creator16/9  "FrwdBkwdPosMin"
  PA_KeSMSwAcsEntryThdRwLtStFrwdBkwdPos_Val/1 -> Bus Creator16/7  "FrwdBkwdPos"
  PA_KeSMSwAcsExtThdRwLtStFrwdBkwdPosMin_Val/1 -> Bus Creator17/9  "FrwdBkwdPosMin"
  PA_KeSMSwAcsExtThdRwLtStBkReclnUpwdDnwdPosMax_Val/1 -> Bus Creator17/2  "BkReclnUpwdDnwdPosMax"
  PA_KeSMSwAcsExtThdRwLtStFrwdBkwdPos_Val/1 -> Bus Creator17/7  "FrwdBkwdPos"
  PA_KeSMSwAcsExtThdRwLtStBkReclnUpwdDnwdPosMin_Val/1 -> Bus Creator17/3  "BkReclnUpwdDnwdPosMin"
  PA_KeSMSwAcsExtThdRwLtStFrwdBkwdPosMax_Val/1 -> Bus Creator17/8  "FrwdBkwdPosMax"
  PA_KeSMSwAcsExtThdRwLtStBkReclnUpwdDnwdPos_Val/1 -> Bus Creator17/1  "BkReclnUpwdDnwdPos"
  PA_KeSMSwAcsExtThdRwLtStCshnFldUpwdDnwdPos_Val/1 -> Bus Creator17/4  "CshnFldUpwdDnwdPos"
  PA_KeSMSwAcsExtThdRwLtStCshnFldUpwdDnwdPosMin_Val/1 -> Bus Creator17/6  "CshnFldUpwdDnwdPosMin"
  PA_KeSMSwAcsExtThdRwLtStCshnFldUpwdDnwdPosMax_Val/1 -> Bus Creator17/5  "CshnFldUpwdDnwdPosMax"
  PA_KeSMSwLugThdRwLtStCshnFldUpwdDnwdPosMax_Val/1 -> Bus Creator18/5  "CshnFldUpwdDnwdPosMax"
  PA_KeSMSwLugThdRwLtStFrwdBkwdPos_Val/1 -> Bus Creator18/7  "FrwdBkwdPos"
  PA_KeSMSwLugThdRwLtStBkReclnUpwdDnwdPos_Val/1 -> Bus Creator18/1  "BkReclnUpwdDnwdPos"
  PA_KeSMSwLugThdRwLtStCshnFldUpwdDnwdPos_Val/1 -> Bus Creator18/4  "CshnFldUpwdDnwdPos"
  PA_KeSMSwLugThdRwLtStBkReclnUpwdDnwdPosMin_Val/1 -> Bus Creator18/3  "BkReclnUpwdDnwdPosMin"
  PA_KeSMSwLugThdRwLtStBkReclnUpwdDnwdPosMax_Val/1 -> Bus Creator18/2  "BkReclnUpwdDnwdPosMax"
  PA_KeSMSwLugThdRwLtStFrwdBkwdPosMax_Val/1 -> Bus Creator18/8  "FrwdBkwdPosMax"
  PA_KeSMSwLugThdRwLtStFrwdBkwdPosMin_Val/1 -> Bus Creator18/9  "FrwdBkwdPosMin"
  PA_KeSMSwLugThdRwLtStCshnFldUpwdDnwdPosMin_Val/1 -> Bus Creator18/6  "CshnFldUpwdDnwdPosMin"
  PA_KeSMSwVIPThdRwLtStFrwdBkwdPos_Val/1 -> Bus Creator20/7  "FrwdBkwdPos"
  PA_KeSMSwVIPThdRwLtStFrwdBkwdPosMax_Val/1 -> Bus Creator20/8  "FrwdBkwdPosMax"
  PA_KeSMSwVIPThdRwLtStCshnFldUpwdDnwdPosMin_Val/1 -> Bus Creator20/6  "CshnFldUpwdDnwdPosMin"
  PA_KeSMSwVIPThdRwLtStBkReclnUpwdDnwdPos_Val/1 -> Bus Creator20/1  "BkReclnUpwdDnwdPos"
  PA_KeSMSwVIPThdRwLtStBkReclnUpwdDnwdPosMax_Val/1 -> Bus Creator20/2  "BkReclnUpwdDnwdPosMax"
  PA_KeSMSwVIPThdRwLtStCshnFldUpwdDnwdPosMax_Val/1 -> Bus Creator20/5  "CshnFldUpwdDnwdPosMax"
  PA_KeSMSwVIPThdRwLtStBkReclnUpwdDnwdPosMin_Val/1 -> Bus Creator20/3  "BkReclnUpwdDnwdPosMin"
  PA_KeSMSwVIPThdRwLtStCshnFldUpwdDnwdPos_Val/1 -> Bus Creator20/4  "CshnFldUpwdDnwdPos"
  PA_KeSMSwVIPThdRwLtStFrwdBkwdPosMin_Val/1 -> Bus Creator20/9  "FrwdBkwdPosMin"
  Bus Creator16/1 -> Bus Creator19/1  "AcsEntryThdRwLtSt"
  Bus Creator17/1 -> Bus Creator19/2  "AcsExtThdRwLtSt"
  Bus Creator18/1 -> Bus Creator19/3  "LugThdRwLtSt"
  Bus Creator20/1 -> Bus Creator19/4  "VIPThdRwLtSt"
  Bus Creator19/1 -> Multiport Switch3/4, Multiport Switch3/2
  [IfKeSMSeStNumConfig_Val] -> Multiport Switch3/1
  Bus Creator21/1 -> Bus Creator25/1  "AcsEntryThdRwRtSt"
  PA_KeSMSwAcsEntryThdRwRtStFrwdBkwdPosMin_Val/1 -> Bus Creator21/9  "FrwdBkwdPosMin"
  PA_KeSMSwAcsEntryThdRwRtStBkReclnUpwdDnwdPosMax_Val/1 -> Bus Creator21/2  "BkReclnUpwdDnwdPosMax"
  PA_KeSMSwAcsEntryThdRwRtStFrwdBkwdPos_Val/1 -> Bus Creator21/7  "FrwdBkwdPos"
  PA_KeSMSwAcsEntryThdRwRtStBkReclnUpwdDnwdPosMin_Val/1 -> Bus Creator21/3  "BkReclnUpwdDnwdPosMin"
  PA_KeSMSwAcsEntryThdRwRtStFrwdBkwdPosMax_Val/1 -> Bus Creator21/8  "FrwdBkwdPosMax"
  PA_KeSMSwAcsEntryThdRwRtStBkReclnUpwdDnwdPos_Val/1 -> Bus Creator21/1  "BkReclnUpwdDnwdPos"
  PA_KeSMSwAcsEntryThdRwRtStCshnFldUpwdDnwdPos_Val/1 -> Bus Creator21/4  "CshnFldUpwdDnwdPos"
  PA_KeSMSwAcsEntryThdRwRtStCshnFldUpwdDnwdPosMin_Val/1 -> Bus Creator21/6  "CshnFldUpwdDnwdPosMin"
  PA_KeSMSwAcsEntryThdRwRtStCshnFldUpwdDnwdPosMax_Val/1 -> Bus Creator21/5  "CshnFldUpwdDnwdPosMax"
  PA_KeSMSwAcsExtThdRwRtStCshnFldUpwdDnwdPosMax_Val/1 -> Bus Creator22/5  "CshnFldUpwdDnwdPosMax"
  PA_KeSMSwAcsExtThdRwRtStFrwdBkwdPosMin_Val/1 -> Bus Creator22/9  "FrwdBkwdPosMin"
  PA_KeSMSwAcsExtThdRwRtStBkReclnUpwdDnwdPosMax_Val/1 -> Bus Creator22/2  "BkReclnUpwdDnwdPosMax"
  PA_KeSMSwAcsExtThdRwRtStFrwdBkwdPos_Val/1 -> Bus Creator22/7  "FrwdBkwdPos"
  PA_KeSMSwAcsExtThdRwRtStCshnFldUpwdDnwdPos_Val/1 -> Bus Creator22/4  "CshnFldUpwdDnwdPos"
  PA_KeSMSwAcsExtThdRwRtStBkReclnUpwdDnwdPosMin_Val/1 -> Bus Creator22/3  "BkReclnUpwdDnwdPosMin"
  PA_KeSMSwAcsExtThdRwRtStFrwdBkwdPosMax_Val/1 -> Bus Creator22/8  "FrwdBkwdPosMax"
  Bus Creator22/1 -> Bus Creator25/2  "AcsExtThdRwRtSt"
  PA_KeSMSwAcsExtThdRwRtStCshnFldUpwdDnwdPosMin_Val/1 -> Bus Creator22/6  "CshnFldUpwdDnwdPosMin"
  PA_KeSMSwAcsExtThdRwRtStBkReclnUpwdDnwdPos_Val/1 -> Bus Creator22/1  "BkReclnUpwdDnwdPos"
  PA_KeSMSwLugThdRwRtStCshnFldUpwdDnwdPosMax_Val/1 -> Bus Creator23/5  "CshnFldUpwdDnwdPosMax"
  PA_KeSMSwLugThdRwRtStFrwdBkwdPosMin_Val/1 -> Bus Creator23/9  "FrwdBkwdPosMin"
  PA_KeSMSwLugThdRwRtStBkReclnUpwdDnwdPosMax_Val/1 -> Bus Creator23/2  "BkReclnUpwdDnwdPosMax"
  PA_KeSMSwLugThdRwRtStFrwdBkwdPos_Val/1 -> Bus Creator23/7  "FrwdBkwdPos"
  PA_KeSMSwLugThdRwRtStCshnFldUpwdDnwdPos_Val/1 -> Bus Creator23/4  "CshnFldUpwdDnwdPos"
  PA_KeSMSwLugThdRwRtStBkReclnUpwdDnwdPosMin_Val/1 -> Bus Creator23/3  "BkReclnUpwdDnwdPosMin"
  PA_KeSMSwLugThdRwRtStFrwdBkwdPosMax_Val/1 -> Bus Creator23/8  "FrwdBkwdPosMax"
  Bus Creator23/1 -> Bus Creator25/3  "LugThdRwRtSt"
  PA_KeSMSwLugThdRwRtStCshnFldUpwdDnwdPosMin_Val/1 -> Bus Creator23/6  "CshnFldUpwdDnwdPosMin"
  PA_KeSMSwLugThdRwRtStBkReclnUpwdDnwdPos_Val/1 -> Bus Creator23/1  "BkReclnUpwdDnwdPos"
  PA_KeSMSwVIPThdRwRtStCshnFldUpwdDnwdPosMax_Val/1 -> Bus Creator24/5  "CshnFldUpwdDnwdPosMax"
  PA_KeSMSwVIPThdRwRtStFrwdBkwdPosMin_Val/1 -> Bus Creator24/9  "FrwdBkwdPosMin"
  PA_KeSMSwVIPThdRwRtStBkReclnUpwdDnwdPosMax_Val/1 -> Bus Creator24/2  "BkReclnUpwdDnwdPosMax"
  PA_KeSMSwVIPThdRwRtStFrwdBkwdPos_Val/1 -> Bus Creator24/7  "FrwdBkwdPos"
  PA_KeSMSwVIPThdRwRtStCshnFldUpwdDnwdPos_Val/1 -> Bus Creator24/4  "CshnFldUpwdDnwdPos"
  PA_KeSMSwVIPThdRwRtStBkReclnUpwdDnwdPosMin_Val/1 -> Bus Creator24/3  "BkReclnUpwdDnwdPosMin"
  PA_KeSMSwVIPThdRwRtStFrwdBkwdPosMax_Val/1 -> Bus Creator24/8  "FrwdBkwdPosMax"
  Bus Creator24/1 -> Bus Creator25/4  "VIPThdRwRtSt"
  PA_KeSMSwVIPThdRwRtStCshnFldUpwdDnwdPosMin_Val/1 -> Bus Creator24/6  "CshnFldUpwdDnwdPosMin"
  PA_KeSMSwVIPThdRwRtStBkReclnUpwdDnwdPos_Val/1 -> Bus Creator24/1  "BkReclnUpwdDnwdPos"
  [IfKeSMSeStNumConfig_Val] -> Multiport Switch4/1
  Bus Creator25/1 -> Multiport Switch4/4, Multiport Switch4/2
  [Calib_2R] -> Bus Creator26/4  "Calib_2R"
  [Calib_3L] -> Bus Creator26/5  "Calib_3L"
  [Calib_3R] -> Bus Creator26/6  "Calib_3R"
  [Calib_2L] -> Bus Creator26/3  "Calib_2L"
  [Calib_Pass] -> Bus Creator26/2  "Calib_Pass"
  [Calib_Drv] -> Bus Creator26/1  "Calib_Drv"
  Bus Creator26/1 -> ModeStCalib/1
  Multiport Switch2/1 -> [Calib_2L]
  Multiport Switch7/1 -> [Calib_2R]
  Multiport Switch3/1 -> [Calib_3L]
  Multiport Switch4/1 -> [Calib_3R]
  PA_KeSMSw6sAcsEntryDrvStFrwdBkwdPos_Val/1 -> Bus Creator27/4  "FrwdBkwdPos"
  PA_KeSMSw6sAcsEntryDrvStFrwdBkwdPosMax_Val/1 -> Bus Creator27/5  "FrwdBkwdPosMax"
  PA_KeSMSw6sAcsEntryDrvStFtUpwdDnwdPos_Val/1 -> Bus Creator27/7  "FtUpwdDnwdPos"
  Bus Creator27/1 -> Bus Creator29/1  "AcsEntryDrvSt"
  PA_KeSMSw6sAcsEntryDrvStFrwdBkwdPosMin_Val/1 -> Bus Creator27/6  "FrwdBkwdPosMin"
  PA_KeSMSw6sAcsEntryDrvStFtUpwdDnwdPosMax_Val/1 -> Bus Creator27/8  "FtUpwdDnwdPosMax"
  PA_KeSMSw6sAcsEntryDrvStBkReclnUpwdDnwdPosMin_Val/1 -> Bus Creator27/3  "BkReclnUpwdDnwdPosMin"
  PA_KeSMSw6sAcsEntryDrvStBkReclnUpwdDnwdPos_Val/1 -> Bus Creator27/1  "BkReclnUpwdDnwdPos"
  PA_KeSMSw6sAcsEntryDrvStFtUpwdDnwdPosMin_Val/1 -> Bus Creator27/9  "FtUpwdDnwdPosMin"
  PA_KeSMSw6sAcsEntryDrvStBkReclnUpwdDnwdPosMax_Val/1 -> Bus Creator27/2  "BkReclnUpwdDnwdPosMax"
  PA_KeSMSw6sAcsExtDrvStBkReclnUpwdDnwdPosMin_Val/1 -> Bus Creator28/3  "BkReclnUpwdDnwdPosMin"
  Bus Creator28/1 -> Bus Creator29/2  "AcsExtDrvSt"
  PA_KeSMSw6sAcsExtDrvStFrwdBkwdPosMin_Val/1 -> Bus Creator28/6  "FrwdBkwdPosMin"
  PA_KeSMSw6sAcsExtDrvStFtUpwdDnwdPos_Val/1 -> Bus Creator28/7  "FtUpwdDnwdPos"
  PA_KeSMSw6sAcsExtDrvStBkReclnUpwdDnwdPosMax_Val/1 -> Bus Creator28/2  "BkReclnUpwdDnwdPosMax"
  PA_KeSMSw6sAcsExtDrvStFrwdBkwdPosMax_Val/1 -> Bus Creator28/5  "FrwdBkwdPosMax"
  PA_KeSMSw6sAcsExtDrvStBkReclnUpwdDnwdPos_Val/1 -> Bus Creator28/1  "BkReclnUpwdDnwdPos"
  PA_KeSMSw6sAcsExtDrvStFtUpwdDnwdPosMin_Val/1 -> Bus Creator28/9  "FtUpwdDnwdPosMin"
  PA_KeSMSw6sAcsExtDrvStFrwdBkwdPos_Val/1 -> Bus Creator28/4  "FrwdBkwdPos"
  PA_KeSMSw6sAcsExtDrvStFtUpwdDnwdPosMax_Val/1 -> Bus Creator28/8  "FtUpwdDnwdPosMax"
  Bus Creator29/1 -> Multiport Switch1/3
  PA_KeSMSw6sAcsEntryPassStFtUpwdDnwdPos_Val/1 -> Bus Creator30/7  "FtUpwdDnwdPos"
  PA_KeSMSw6sAcsEntryPassStFtUpwdDnwdPosMiax_Val/1 -> Bus Creator30/8  "FtUpwdDnwdPosMax"
  PA_KeSMSw6sAcsEntryPassStFrwdBkwdPos_Val/1 -> Bus Creator30/4  "FrwdBkwdPos"
  PA_KeSMSw6sAcsEntryPassStFrwdBkwdPosMin_Val/1 -> Bus Creator30/6  "FrwdBkwdPosMin"
  Bus Creator30/1 -> Bus Creator32/1  "AcsEntryPassSt"
  PA_KeSMSw6sAcsEntryPassStFrwdBkwdPosMax_Val/1 -> Bus Creator30/5  "FrwdBkwdPosMax"
  PA_KeSMSw6sAcsEntryPassStFtUpwdDnwdPosMin_Val/1 -> Bus Creator30/9  "FtUpwdDnwdPosMin"
  PA_KeSMSw6sAcsEntryPassStBkReclnUpwdDnwdPosMax_Val/1 -> Bus Creator30/2  "BkReclnUpwdDnwdPosMax"
  PA_KeSMSw6sAcsEntryPassStBkReclnUpwdDnwdPosMin_Val/1 -> Bus Creator30/3  "BkReclnUpwdDnwdPosMin"
  PA_KeSMSw6sAcsEntryPassStBkReclnUpwdDnwdPos_Val/1 -> Bus Creator30/1  "BkReclnUpwdDnwdPos"
  Bus Creator31/1 -> Bus Creator32/2  "AcsExtPassSt"
  PA_KeSMSw6sAcsExtPassStFrwdBkwdPos_Val/1 -> Bus Creator31/4  "FrwdBkwdPos"
  PA_KeSMSw6sAcsExtPassStFrwdBkwdPosMin_Val/1 -> Bus Creator31/6  "FrwdBkwdPosMin"
  PA_KeSMSw6sAcsExtPassStBkReclnUpwdDnwdPos_Val/1 -> Bus Creator31/1  "BkReclnUpwdDnwdPos"
  PA_KeSMSw6sAcsExtPassStFrwdBkwdPosMax_Val/1 -> Bus Creator31/5  "FrwdBkwdPosMax"
  PA_KeSMSw6sAcsExtPassStBkReclnUpwdDnwdPosMin_Val/1 -> Bus Creator31/3  "BkReclnUpwdDnwdPosMin"
  PA_KeSMSw6sAcsExtPassStFtUpwdDnwdPosMax_Val/1 -> Bus Creator31/8  "FtUpwdDnwdPosMax"
  PA_KeSMSw6sAcsExtPassStFtUpwdDnwdPos_Val/1 -> Bus Creator31/7  "FtUpwdDnwdPos"
  PA_KeSMSw6sAcsExtPassStFtUpwdDnwdPosMin_Val/1 -> Bus Creator31/9  "FtUpwdDnwdPosMin"
  PA_KeSMSw6sAcsExtPassStBkReclnUpwdDnwdPosMax_Val/1 -> Bus Creator31/2  "BkReclnUpwdDnwdPosMax"
  Bus Creator32/1 -> Multiport Switch6/3
  PA_KeSMSw6sAcsEntrySecRwLtStBkReclnUpwdDnwdPosMax_Val/1 -> Bus Creator33/5  "BkReclnUpwdDnwdPosMax"
  PA_KeSMSw6sAcsEntrySecRwLtStFrwdBkwdPosMin_Val/1 -> Bus Creator33/9  "FrwdBkwdPosMin"
  PA_KeSMSw6sAcsEntrySecRwLtStBkReclnUpwdDnwdPos_Val/1 -> Bus Creator33/4  "BkReclnUpwdDnwdPos"
  PA_KeSMSw6sAcsEntrySecRwLtStLtwdRtwdPosMin_Val/1 -> Bus Creator33/18  "LtwdRtwdPosMin"
  PA_KeSMSw6sAcsEntrySecRwLtStBkReclnUpwdDnwdPosMin_Val/1 -> Bus Creator33/6  "BkReclnUpwdDnwdPosMin"
  PA_KeSMSw6sAcsEntrySecRwLtStLtwdRtwdPos_Val/1 -> Bus Creator33/16  "LtwdRtwdPos"
  PA_KeSMSw6sAcsEntrySecRwLtStFrwdBkwdPos_Val/1 -> Bus Creator33/7  "FrwdBkwdPos"
  PA_KeSMSw6sAcsEntrySecRwLtStLgrstUpwdPos_Val/1 -> Bus Creator33/13  "LgrstUpwdPos"
  PA_KeSMSw6sAcsEntrySecRwLtStHdrstUpwdPosMin_Val/1 -> Bus Creator33/12  "HdrstUpwdPosMin"
  PA_KeSMSw6sAcsEntrySecRwLtStHdrstUpwdPos_Val/1 -> Bus Creator33/10  "HdrstUpwdPos"
  PA_KeSMSw6sAcsEntrySecRwLtStArmScrnPos_Val/1 -> Bus Creator33/1  "ArmScrnPos"
  Bus Creator33/1 -> Bus Creator37/1  "AcsEntrySecRwLtSt"
  PA_KeSMSw6sAcsEntrySecRwLtStFrwdBkwdPosMax_Val/1 -> Bus Creator33/8  "FrwdBkwdPosMax"
  PA_KeSMSw6sAcsEntrySecRwLtStLgrstUpwdPosMax_Val/1 -> Bus Creator33/14  "LgrstUpwdPosMax"
  PA_KeSMSw6sAcsEntrySecRwLtStArmScrnPosMin_Val/1 -> Bus Creator33/3  "ArmScrnPosMin"
  PA_KeSMSw6sAcsEntrySecRwLtStHdrstUpwdPosMax_Val/1 -> Bus Creator33/11  "HdrstUpwdPosMax"
  PA_KeSMSw6sAcsEntrySecRwLtStLtwdRtwdPosMax_Val/1 -> Bus Creator33/17  "LtwdRtwdPosMax"
  PA_KeSMSw6sAcsEntrySecRwLtStArmScrnPosMax_Val/1 -> Bus Creator33/2  "ArmScrnPosMax"
  PA_KeSMSw6sAcsEntrySecRwLtStLgrstUpwdPosMin_Val/1 -> Bus Creator33/15  "LgrstUpwdPosMin"
  PA_KeSMSw6sAcsExtSecRwLtStFrwdBkwdPosMax_Val/1 -> Bus Creator34/8  "FrwdBkwdPosMax"
  PA_KeSMSwDltTrgtPos_Val8/1 -> Bus Creator34/12  "HdrstUpwdPosMin"
  PA_KeSMSw6sAcsExtSecRwLtStBkReclnUpwdDnwdPosMin_Val/1 -> Bus Creator34/6  "BkReclnUpwdDnwdPosMin"
  PA_KeSMSw6sAcsExtSecRwLtStLtwdRtwdPosMax_Val/1 -> Bus Creator34/17  "LtwdRtwdPosMax"
  PA_KeSMSw6sAcsExtSecRwLtStFrwdBkwdPosMin_Val/1 -> Bus Creator34/9  "FrwdBkwdPosMin"
  Bus Creator34/1 -> Bus Creator37/2  "AcsExtSecRwLtSt"
  PA_KeSMSw6sAcsExtSecRwLtStLtwdRtwdPosMin_Val/1 -> Bus Creator34/18  "LtwdRtwdPosMin"
  PA_KeSMSw6sAcsExtSecRwLtStLgrstUpwdDnwdPos_Val/1 -> Bus Creator34/13  "LgrstUpwdPos"
  PA_KeSMSw6sAcsExtSecRwLtStArmScrnPosMax_Val/1 -> Bus Creator34/2  "ArmScrnPosMax"
  PA_KeSMSw6sAcsExtSecRwLtStFrwdBkwdPos_Val/1 -> Bus Creator34/7  "FrwdBkwdPos"
  PA_KeSMSw6sAcsExtSecRwLtStBkReclnUpwdDnwdPosMax_Val/1 -> Bus Creator34/5  "BkReclnUpwdDnwdPosMax"
  PA_KeSMSw6sAcsExtSecRwLtStBkReclnUpwdDnwdPos_Val/1 -> Bus Creator34/4  "BkReclnUpwdDnwdPos"
  PA_KeSMSw6sAcsExtSecRwLtStLtwdRtwdPos_Val/1 -> Bus Creator34/16  "LtwdRtwdPos"
  PA_KeSMSwDltTrgtPos_Val7/1 -> Bus Creator34/10  "HdrstUpwdPos"
  PA_KeSMSw6sAcsExtSecRwLtStLgrstUpwdDnwdPosMin_Val/1 -> Bus Creator34/15  "LgrstUpwdPosMin"
  PA_KeSMSw6sAcsExtSecRwLtStLgrstUpwdDnwdPosMax_Val/1 -> Bus Creator34/14  "LgrstUpwdPosMax"
  PA_KeSMSw6sAcsExtSecRwLtStArmScrnPosMin_Val/1 -> Bus Creator34/3  "ArmScrnPosMin"
  PA_KeSMSw6sAcsExtSecRwLtStArmScrnPos_Val/1 -> Bus Creator34/1  "ArmScrnPos"
  PA_KeSMSwDltTrgtPos_Val6/1 -> Bus Creator34/11  "HdrstUpwdPosMax"
  PA_KeSMSw6sRecoveryMdSecRwLtStHdrstUpwdDnwdPos_Val/1 -> Bus Creator35/10  "HdrstUpwdPos"
  PA_KeSMSw6sRecoveryMdSecRwLtStLtwdRtwdPos_Val/1 -> Bus Creator35/16  "LtwdRtwdPos"
  PA_KeSMSw6sRecoveryMdSecRwLtStLgrstUpwdDnwdPosMax_Val/1 -> Bus Creator35/14  "LgrstUpwdPosMax"
  PA_KeSMSw6sRecoveryMdSecRwLtStHdrstUpwdDnwdPosMin_Val/1 -> Bus Creator35/12  "HdrstUpwdPosMin"
  PA_KeSMSw6sRecoveryMdSecRwLtStArmScrnPos_Val/1 -> Bus Creator35/1  "ArmScrnPos"
  PA_KeSMSw6sRecoveryMdSecRwLtStLgrstUpwdDnwdPosMin_Val/1 -> Bus Creator35/15  "LgrstUpwdPosMin"
  Bus Creator35/1 -> Bus Creator37/3  "RecoveryMdSecRwLtSt"
  PA_KeSMSw6sRecoveryMdSecRwLtStArmScrnPosMax_Val/1 -> Bus Creator35/2  "ArmScrnPosMax"
  PA_KeSMSw6sRecoveryMdSecRwLtStLtwdRtwdPosMax_Val/1 -> Bus Creator35/17  "LtwdRtwdPosMax"
  PA_KeSMSw6sRecoveryMdSecRwLtStBkReclnUpwdDnwdPosMin_Val/1 -> Bus Creator35/6  "BkReclnUpwdDnwdPosMin"
  PA_KeSMSw6sRecoveryMdSecRwLtStBkReclnUpwdDnwdPos_Val/1 -> Bus Creator35/4  "BkReclnUpwdDnwdPos"
  PA_KeSMSw6sRecoveryMdSecRwLtStHdrstUpwdDnwdPosMax_Val/1 -> Bus Creator35/11  "HdrstUpwdPosMax"
  PA_KeSMSw6sRecoveryMdSecRwLtStFrwdBkwdPosMax_Val/1 -> Bus Creator35/8  "FrwdBkwdPosMax"
  PA_KeSMSw6sRecoveryMdSecRwLtStLtwdRtwdPosMin_Val/1 -> Bus Creator35/18  "LtwdRtwdPosMin"
  PA_KeSMSw6sRecoveryMdSecRwLtStArmScrnPosMin_Val/1 -> Bus Creator35/3  "ArmScrnPosMin"
  PA_KeSMSw6sRecoveryMdSecRwLtStFrwdBkwdPosMin_Val/1 -> Bus Creator35/9  "FrwdBkwdPosMin"
  PA_KeSMSw6sRecoveryMdSecRwLtStBkReclnUpwdDnwdPosMax_Val/1 -> Bus Creator35/5  "BkReclnUpwdDnwdPosMax"
  PA_KeSMSw6sRecoveryMdSecRwLtStFrwdBkwdPos_Val/1 -> Bus Creator35/7  "FrwdBkwdPos"
  PA_KeSMSw6sRecoveryMdSecRwLtStLgrstUpwdDnwdPos_Val/1 -> Bus Creator35/13  "LgrstUpwdPos"
  PA_KeSMSw6sVIPSecRwLtStLtwdRtwdPosMax_Val/1 -> Bus Creator36/17  "LtwdRtwdPosMax"
  PA_KeSMSw6sVIPSecRwLtStHdrstUpwdPosMin_Val/1 -> Bus Creator36/12  "HdrstUpwdPosMin"
  PA_KeSMSw6sVIPSecRwLtStBkReclnUpwdDnwdPosMax_Val/1 -> Bus Creator36/5  "BkReclnUpwdDnwdPosMax"
  PA_KeSMSw6sVIPSecRwLtStFrwdBkwdPosMax_Val/1 -> Bus Creator36/8  "FrwdBkwdPosMax"
  PA_KeSMSw6sVIPSecRwLtStLgrstUpwdPos_Val/1 -> Bus Creator36/13  "LgrstUpwdPos"
  PA_KeSMSw6sVIPSecRwLtStHdrstUpwdPosMax_Val/1 -> Bus Creator36/11  "HdrstUpwdPosMax"
  PA_KeSMSw6sVIPSecRwLtStBkReclnUpwdDnwdPosMin_Val/1 -> Bus Creator36/6  "BkReclnUpwdDnwdPosMin"
  PA_KeSMSw6sVIPSecRwLtStLtwdRtwdPosMin_Val/1 -> Bus Creator36/18  "LtwdRtwdPosMin"
  Bus Creator36/1 -> Bus Creator37/4  "VIPSecRwLtSt"
  PA_KeSMSw6sVIPSecRwLtStBkReclnUpwdDnwdPos_Val/1 -> Bus Creator36/4  "BkReclnUpwdDnwdPos"
  PA_KeSMSw6sVIPSecRwLtStFrwdBkwdPosMin_Val/1 -> Bus Creator36/9  "FrwdBkwdPosMin"
  PA_KeSMSw6sVIPSecRwLtStLgrstUpwdPosMax_Val/1 -> Bus Creator36/14  "LgrstUpwdPosMax"
  PA_KeSMSw6sVIPSecRwLtStLtwdRtwdPos_Val/1 -> Bus Creator36/16  "LtwdRtwdPos"
  PA_KeSMSw6sVIPSecRwLtStLgrstUpwdPosMin_Val/1 -> Bus Creator36/15  "LgrstUpwdPosMin"
  PA_KeSMSw6sVIPSecRwLtStArmScrnPos_Val/1 -> Bus Creator36/1  "ArmScrnPos"
  PA_KeSMSw6sVIPSecRwLtStArmScrnPosMin_Val/1 -> Bus Creator36/3  "ArmScrnPosMin"
  PA_KeSMSw6sVIPSecRwLtStFrwdBkwdPos_Val/1 -> Bus Creator36/7  "FrwdBkwdPos"
  PA_KeSMSw6sVIPSecRwLtStHdrstUpwdPos_Val/1 -> Bus Creator36/10  "HdrstUpwdPos"
  PA_KeSMSw6sVIPSecRwLtStArmScrnPosMax_Val/1 -> Bus Creator36/2  "ArmScrnPosMax"
  Bus Creator37/1 -> Multiport Switch2/3
  PA_KeSMSw6sAcsEntrySecRwRtStLgrstUpwdPosMax_Val/1 -> Bus Creator38/14  "LgrstUpwdPosMax"
  PA_KeSMSw6sAcsEntrySecRwRtStHdrstUpwdPosMax_Val/1 -> Bus Creator38/11  "HdrstUpwdPosMax"
  PA_KeSMSw6sAcsEntrySecRwRtStLtwdRtwdPos_Val/1 -> Bus Creator38/16  "LtwdRtwdPos"
  PA_KeSMSw6sAcsEntrySecRwRtStHdrstUpwdPos_Val/1 -> Bus Creator38/10  "HdrstUpwdPos"
  PA_KeSMSw6sAcsEntrySecRwRtStArmScrnPos_Val/1 -> Bus Creator38/1  "ArmScrnPos"
  PA_KeSMSw6sAcsEntrySecRwRtStFrwdBkwdPosMax_Val/1 -> Bus Creator38/8  "FrwdBkwdPosMax"
  PA_KeSMSw6sAcsEntrySecRwRtStBkReclnUpwdDnwdPosMax_Val/1 -> Bus Creator38/5  "BkReclnUpwdDnwdPosMax"
  Bus Creator38/1 -> Bus Creator42/1  "AcsEntrySecRwRtSt"
  PA_KeSMSw6sAcsEntrySecRwRtStLgrstUpwdPosMin_Val/1 -> Bus Creator38/15  "LgrstUpwdPosMin"
  PA_KeSMSw6sAcsEntrySecRwRtStLtwdRtwdPosMax_Val/1 -> Bus Creator38/17  "LtwdRtwdPosMax"
  PA_KeSMSw6sAcsEntrySecRwRtStHdrstUpwdPosMin_Val/1 -> Bus Creator38/12  "HdrstUpwdPosMin"
  PA_KeSMSw6sAcsEntrySecRwRtStFrwdBkwdPos_Val/1 -> Bus Creator38/7  "FrwdBkwdPos"
  PA_KeSMSw6sAcsEntrySecRwRtStFrwdBkwdPosMin_Val/1 -> Bus Creator38/9  "FrwdBkwdPosMin"
  PA_KeSMSw6sAcsEntrySecRwRtStLgrstUpwdPos_Val/1 -> Bus Creator38/13  "LgrstUpwdPos"
  PA_KeSMSw6sAcsEntrySecRwRtStLtwdRtwdPosMin_Val/1 -> Bus Creator38/18  "LtwdRtwdPosMin"
  PA_KeSMSw6sAcsEntrySecRwRtStArmScrnPosMax_Val/1 -> Bus Creator38/2  "ArmScrnPosMax"
  PA_KeSMSw6sAcsEntrySecRwRtStBkReclnUpwdDnwdPosMin_Val/1 -> Bus Creator38/6  "BkReclnUpwdDnwdPosMin"
  PA_KeSMSw6sAcsEntrySecRwRtStArmScrnPosMin_Val/1 -> Bus Creator38/3  "ArmScrnPosMin"
  PA_KeSMSw6sAcsEntrySecRwRtStBkReclnUpwdDnwdPos_Val/1 -> Bus Creator38/4  "BkReclnUpwdDnwdPos"
  Bus Creator39/1 -> Bus Creator42/2  "AcsExtSecRwRSt"
  PA_KeSMSw6sAcsExtSecRwRtStFrwdBkwdPos_Val/1 -> Bus Creator39/7  "FrwdBkwdPos"
  PA_KeSMSw6sAcsExtSecRwRtStArmScrnPosMax_Val/1 -> Bus Creator39/2  "ArmScrnPosMax"
  PA_KeSMSw6sAcsExtSecRwRtStLgrstUpwdDnwdPos_Val/1 -> Bus Creator39/13  "LgrstUpwdPos"
  PA_KeSMSw6sAcsExtSecRwRtStLtwdRtwdPosMax_Val/1 -> Bus Creator39/17  "LtwdRtwdPosMax"
  PA_KeSMSw6sAcsExtSecRwRtStFrwdBkwdPosMax_Val/1 -> Bus Creator39/8  "FrwdBkwdPosMax"
  PA_KeSMSw6sAcsExtSecRwRtStLgrstUpwdDnwdPosMax_Val/1 -> Bus Creator39/14  "LgrstUpwdPosMax"
  PA_KeSMSw6sAcsExtSecRwRtStBkReclnUpwdDnwdPosMin_Val/1 -> Bus Creator39/6  "BkReclnUpwdDnwdPosMin"
  PA_KeSMSwDltTrgtPos_Val9/1 -> Bus Creator39/11  "HdrstUpwdPosMax"
  PA_KeSMSw6sAcsExtSecRwRtStBkReclnUpwdDnwdPosMax_Val/1 -> Bus Creator39/5  "BkReclnUpwdDnwdPosMax"
  PA_KeSMSw6sAcsExtSecRwRtStArmScrnPosMin_Val/1 -> Bus Creator39/3  "ArmScrnPosMin"
  PA_KeSMSw6sAcsExtSecRwRtStFrwdBkwdPosMin_Val/1 -> Bus Creator39/9  "FrwdBkwdPosMin"
  PA_KeSMSw6sAcsExtSecRwRtStLgrstUpwdDnwdPosMin_Val/1 -> Bus Creator39/15  "LgrstUpwdPosMin"
  PA_KeSMSw6sAcsExtSecRwRtStLtwdRtwdPosMin_Val/1 -> Bus Creator39/18  "LtwdRtwdPosMin"
  PA_KeSMSw6sAcsExtSecRwRtStLtwdRtwdPos_Val/1 -> Bus Creator39/16  "LtwdRtwdPos"
  PA_KeSMSw6sAcsExtSecRwRtStArmScrnPos_Val/1 -> Bus Creator39/1  "ArmScrnPos"
  PA_KeSMSw6sAcsExtSecRwRtStBkReclnUpwdDnwdPos_Val/1 -> Bus Creator39/4  "BkReclnUpwdDnwdPos"
  PA_KeSMSwDltTrgtPos_Val10/1 -> Bus Creator39/10  "HdrstUpwdPos"
  PA_KeSMSwDltTrgtPos_Val11/1 -> Bus Creator39/12  "HdrstUpwdPosMin"
  PA_KeSMSw6sRecoveryMdSecRwRtStFrwdBkwdPosMin_Val/1 -> Bus Creator40/9  "FrwdBkwdPosMin"
  PA_KeSMSw6sRecoveryMdSecRwRtStLgrstUpwdDnwdPos_Val/1 -> Bus Creator40/13  "LgrstUpwdPos"
  PA_KeSMSw6sRecoveryMdSecRwRtStLtwdRtwdPosMin_Val/1 -> Bus Creator40/18  "LtwdRtwdPosMin"
  PA_KeSMSw6sRecoveryMdSecRwRtStHdrstUpwdDnwdPosMin_Val/1 -> Bus Creator40/12  "HdrstUpwdPosMin"
  PA_KeSMSw6sRecoveryMdSecRwRtStBkReclnUpwdDnwdPosMax_Val/1 -> Bus Creator40/5  "BkReclnUpwdDnwdPosMax"
  PA_KeSMSw6sRecoveryMdSecRwRtStFrwdBkwdPos_Val/1 -> Bus Creator40/7  "FrwdBkwdPos"
  PA_KeSMSw6sRecoveryMdSecRwRtStArmScrnPosMax_Val/1 -> Bus Creator40/2  "ArmScrnPosMax"
  PA_KeSMSw6sRecoveryMdSecRwRtStHdrstUpwdDnwdPos_Val/1 -> Bus Creator40/10  "HdrstUpwdPos"
  PA_KeSMSw6sRecoveryMdSecRwRtStArmScrnPos_Val/1 -> Bus Creator40/1  "ArmScrnPos"
  PA_KeSMSw6sRecoveryMdSecRwRtStLgrstUpwdDnwdPosMin_Val/1 -> Bus Creator40/15  "LgrstUpwdPosMin"
  PA_KeSMSw6sRecoveryMdSecRwRtStFrwdBkwdPosMax_Val/1 -> Bus Creator40/8  "FrwdBkwdPosMax"
  PA_KeSMSw6sRecoveryMdSecRwRtStBkReclnUpwdDnwdPos_Val/1 -> Bus Creator40/4  "BkReclnUpwdDnwdPos"
  Bus Creator40/1 -> Bus Creator42/3  "RecoveryMdSecRwRtSt"
  PA_KeSMSw6sRecoveryMdSecRwRtStHdrstUpwdDnwdPosMax_Val/1 -> Bus Creator40/11  "HdrstUpwdPosMax"
  PA_KeSMSw6sRecoveryMdSecRwRtStLgrstUpwdDnwdPosMax_Val/1 -> Bus Creator40/14  "LgrstUpwdPosMax"
  PA_KeSMSw6sRecoveryMdSecRwRtStArmScrnPosMin_Val/1 -> Bus Creator40/3  "ArmScrnPosMin"
  PA_KeSMSw6sRecoveryMdSecRwRtStLtwdRtwdPos_Val/1 -> Bus Creator40/16  "LtwdRtwdPos"
  PA_KeSMSw6sRecoveryMdSecRwRtStBkReclnUpwdDnwdPosMin_Val/1 -> Bus Creator40/6  "BkReclnUpwdDnwdPosMin"
  PA_KeSMSw6sRecoveryMdSecRwRtStLtwdRtwdPosMax_Val/1 -> Bus Creator40/17  "LtwdRtwdPosMax"
  Bus Creator41/1 -> Bus Creator42/4  "VIPSecRwRtSt"
  PA_KeSMSw6sVIPSecRwRtStFrwdBkwdPosMax_Val/1 -> Bus Creator41/8  "FrwdBkwdPosMax"
  PA_KeSMSw6sVIPSecRwRtStArmScrnPosMax_Val/1 -> Bus Creator41/2  "ArmScrnPosMax"
  PA_KeSMSw6sVIPSecRwRtStArmScrnPos_Val/1 -> Bus Creator41/1  "ArmScrnPos"
  PA_KeSMSw6sVIPSecRwRtStLtwdRtwdPosMax_Val/1 -> Bus Creator41/17  "LtwdRtwdPosMax"
  PA_KeSMSw6sVIPSecRwRtStLtwdRtwdPosMin_Val/1 -> Bus Creator41/18  "LtwdRtwdPosMin"
  PA_KeSMSw6sVIPSecRwRtStBkReclnUpwdDnwdPosMin_Val/1 -> Bus Creator41/6  "BkReclnUpwdDnwdPosMin"
  PA_KeSMSw6sVIPSecRwRtStBkReclnUpwdDnwdPosMax_Val/1 -> Bus Creator41/5  "BkReclnUpwdDnwdPosMax"
  PA_KeSMSw6sVIPSecRwRtStLtwdRtwdPos_Val/1 -> Bus Creator41/16  "LtwdRtwdPos"
  PA_KeSMSw6sVIPSecRwRtStLgrstUpwdPosMin_Val/1 -> Bus Creator41/15  "LgrstUpwdPosMin"
  PA_KeSMSw6sVIPSecRwRtStFrwdBkwdPosMin_Val/1 -> Bus Creator41/9  "FrwdBkwdPosMin"
  PA_KeSMSw6sVIPSecRwRtStHdrstUpwdPosMin_Val/1 -> Bus Creator41/12  "HdrstUpwdPosMin"
  PA_KeSMSw6sVIPSecRwRtStHdrstUpwdPos_Val/1 -> Bus Creator41/10  "HdrstUpwdPos"
  PA_KeSMSw6sVIPSecRwRtStHdrstUpwdPosMax_Val/1 -> Bus Creator41/11  "HdrstUpwdPosMax"
  PA_KeSMSw6sVIPSecRwRtStLgrstUpwdPos_Val/1 -> Bus Creator41/13  "LgrstUpwdPos"
  PA_KeSMSw6sVIPSecRwRtStFrwdBkwdPos_Val/1 -> Bus Creator41/7  "FrwdBkwdPos"
  PA_KeSMSw6sVIPSecRwRtStBkReclnUpwdDnwdPos_Val/1 -> Bus Creator41/4  "BkReclnUpwdDnwdPos"
  PA_KeSMSw6sVIPSecRwRtStLgrstUpwdPosMax_Val/1 -> Bus Creator41/14  "LgrstUpwdPosMax"
  PA_KeSMSw6sVIPSecRwRtStArmScrnPosMin_Val/1 -> Bus Creator41/3  "ArmScrnPosMin"
  Bus Creator42/1 -> Multiport Switch7/3
  Bus Creator43/1 -> Bus Creator47/1  "AcsEntryThdRwLtSt"
  PA_KeSMSw6sAcsEntryThdRwLtStBkReclnUpwdDnwdPosMin_Val/1 -> Bus Creator43/3  "BkReclnUpwdDnwdPosMin"
  PA_KeSMSw6sAcsEntryThdRwLtStBkReclnUpwdDnwdPosMax_Val/1 -> Bus Creator43/2  "BkReclnUpwdDnwdPosMax"
  PA_KeSMSw6sAcsEntryThdRwLtStFrwdBkwdPos_Val/1 -> Bus Creator43/7  "FrwdBkwdPos"
  PA_KeSMSw6sAcsEntryThdRwLtStCshnFldUpwdDnwdPosMax_Val/1 -> Bus Creator43/5  "CshnFldUpwdDnwdPosMax"
  PA_KeSMSw6sAcsEntryThdRwLtStFrwdBkwdPosMin_Val/1 -> Bus Creator43/9  "FrwdBkwdPosMin"
  PA_KeSMSw6sAcsEntryThdRwLtStCshnFldUpwdDnwdPos_Val/1 -> Bus Creator43/4  "CshnFldUpwdDnwdPos"
  PA_KeSMSw6sAcsEntryThdRwLtStBkReclnUpwdDnwdPos_Val/1 -> Bus Creator43/1  "BkReclnUpwdDnwdPos"
  PA_KeSMSw6sAcsEntryThdRwLtStFrwdBkwdPosMax_Val/1 -> Bus Creator43/8  "FrwdBkwdPosMax"
  PA_KeSMSw6sAcsEntryThdRwLtStCshnFldUpwdDnwdPosMin_Val/1 -> Bus Creator43/6  "CshnFldUpwdDnwdPosMin"
  PA_KeSMSw6sAcsExtThdRwLtStFrwdBkwdPosMin_Val/1 -> Bus Creator44/9  "FrwdBkwdPosMin"
  PA_KeSMSw6sAcsExtThdRwLtStBkReclnUpwdDnwdPos_Val/1 -> Bus Creator44/1  "BkReclnUpwdDnwdPos"
  PA_KeSMSw6sAcsExtThdRwLtStBkReclnUpwdDnwdPosMax_Val/1 -> Bus Creator44/2  "BkReclnUpwdDnwdPosMax"
  Bus Creator44/1 -> Bus Creator47/2  "AcsExtThdRwLtSt"
  PA_KeSMSw6sAcsExtThdRwLtStCshnFldUpwdDnwdPosMin_Val/1 -> Bus Creator44/6  "CshnFldUpwdDnwdPosMin"
  PA_KeSMSw6sAcsExtThdRwLtStBkReclnUpwdDnwdPosMin_Val/1 -> Bus Creator44/3  "BkReclnUpwdDnwdPosMin"
  PA_KeSMSw6sAcsExtThdRwLtStCshnFldUpwdDnwdPosMax_Val/1 -> Bus Creator44/5  "CshnFldUpwdDnwdPosMax"
  PA_KeSMSw6sAcsExtThdRwLtStCshnFldUpwdDnwdPos_Val/1 -> Bus Creator44/4  "CshnFldUpwdDnwdPos"
  PA_KeSMSw6sAcsExtThdRwLtStFrwdBkwdPos_Val/1 -> Bus Creator44/7  "FrwdBkwdPos"
  PA_KeSMSw6sAcsExtThdRwLtStFrwdBkwdPosMax_Val/1 -> Bus Creator44/8  "FrwdBkwdPosMax"
  PA_KeSMSw6sLugThdRwLtStBkReclnUpwdDnwdPosMax_Val/1 -> Bus Creator45/2  "BkReclnUpwdDnwdPosMax"
  PA_KeSMSw6sLugThdRwLtStCshnFldUpwdDnwdPosMin_Val/1 -> Bus Creator45/6  "CshnFldUpwdDnwdPosMin"
  PA_KeSMSw6sLugThdRwLtStCshnFldUpwdDnwdPos_Val/1 -> Bus Creator45/4  "CshnFldUpwdDnwdPos"
  PA_KeSMSw6sLugThdRwLtStFrwdBkwdPosMin_Val/1 -> Bus Creator45/9  "FrwdBkwdPosMin"
  PA_KeSMSw6sLugThdRwLtStBkReclnUpwdDnwdPos_Val/1 -> Bus Creator45/1  "BkReclnUpwdDnwdPos"
  PA_KeSMSw6sLugThdRwLtStCshnFldUpwdDnwdPosMax_Val/1 -> Bus Creator45/5  "CshnFldUpwdDnwdPosMax"
  PA_KeSMSw6sLugThdRwLtStFrwdBkwdPosMax_Val/1 -> Bus Creator45/8  "FrwdBkwdPosMax"
  Bus Creator45/1 -> Bus Creator47/3  "LugThdRwLtSt"
  PA_KeSMSw6sLugThdRwLtStBkReclnUpwdDnwdPosMin_Val/1 -> Bus Creator45/3  "BkReclnUpwdDnwdPosMin"
  PA_KeSMSw6sLugThdRwLtStFrwdBkwdPos_Val/1 -> Bus Creator45/7  "FrwdBkwdPos"
  PA_KeSMSw6sVIPThdRwLtStBkReclnUpwdDnwdPos_Val/1 -> Bus Creator46/1  "BkReclnUpwdDnwdPos"
  Bus Creator46/1 -> Bus Creator47/4  "VIPThdRwLtSt"
  PA_KeSMSw6sVIPThdRwLtStCshnFldUpwdDnwdPosMin_Val/1 -> Bus Creator46/6  "CshnFldUpwdDnwdPosMin"
  PA_KeSMSw6sVIPThdRwLtStCshnFldUpwdDnwdPosMax_Val/1 -> Bus Creator46/5  "CshnFldUpwdDnwdPosMax"
  PA_KeSMSw6sVIPThdRwLtStBkReclnUpwdDnwdPosMax_Val/1 -> Bus Creator46/2  "BkReclnUpwdDnwdPosMax"
  PA_KeSMSw6sVIPThdRwLtStCshnFldUpwdDnwdPos_Val/1 -> Bus Creator46/4  "CshnFldUpwdDnwdPos"
  PA_KeSMSw6sVIPThdRwLtStFrwdBkwdPosMin_Val/1 -> Bus Creator46/9  "FrwdBkwdPosMin"
  PA_KeSMSw6sVIPThdRwLtStFrwdBkwdPosMax_Val/1 -> Bus Creator46/8  "FrwdBkwdPosMax"
  PA_KeSMSw6sVIPThdRwLtStFrwdBkwdPos_Val/1 -> Bus Creator46/7  "FrwdBkwdPos"
  PA_KeSMSw6sVIPThdRwLtStBkReclnUpwdDnwdPosMin_Val/1 -> Bus Creator46/3  "BkReclnUpwdDnwdPosMin"
  Bus Creator47/1 -> Multiport Switch3/3
  PA_KeSMSw6sAcsEntryThdRwRtStFrwdBkwdPos_Val/1 -> Bus Creator48/7  "FrwdBkwdPos"
  PA_KeSMSw6sAcsEntryThdRwRtStCshnFldUpwdDnwdPosMax_Val/1 -> Bus Creator48/5  "CshnFldUpwdDnwdPosMax"
  PA_KeSMSw6sAcsEntryThdRwRtStBkReclnUpwdDnwdPos_Val/1 -> Bus Creator48/1  "BkReclnUpwdDnwdPos"
  PA_KeSMSw6sAcsEntryThdRwRtStCshnFldUpwdDnwdPos_Val/1 -> Bus Creator48/4  "CshnFldUpwdDnwdPos"
  PA_KeSMSw6sAcsEntryThdRwRtStBkReclnUpwdDnwdPosMax_Val/1 -> Bus Creator48/2  "BkReclnUpwdDnwdPosMax"
  PA_KeSMSw6sAcsEntryThdRwRtStCshnFldUpwdDnwdPosMin_Val/1 -> Bus Creator48/6  "CshnFldUpwdDnwdPosMin"
  PA_KeSMSw6sAcsEntryThdRwRtStFrwdBkwdPosMax_Val/1 -> Bus Creator48/8  "FrwdBkwdPosMax"
  PA_KeSMSw6sAcsEntryThdRwRtStFrwdBkwdPosMin_Val/1 -> Bus Creator48/9  "FrwdBkwdPosMin"
  PA_KeSMSw6sAcsEntryThdRwRtStBkReclnUpwdDnwdPosMin_Val/1 -> Bus Creator48/3  "BkReclnUpwdDnwdPosMin"
  Bus Creator48/1 -> Bus Creator52/1  "AcsEntryThdRwRtSt"
  PA_KeSMSw6sAcsExtThdRwRtStBkReclnUpwdDnwdPosMax_Val/1 -> Bus Creator49/2  "BkReclnUpwdDnwdPosMax"
  PA_KeSMSw6sAcsExtThdRwRtStFrwdBkwdPosMax_Val/1 -> Bus Creator49/8  "FrwdBkwdPosMax"
  PA_KeSMSw6sAcsExtThdRwRtStCshnFldUpwdDnwdPosMin_Val/1 -> Bus Creator49/6  "CshnFldUpwdDnwdPosMin"
  PA_KeSMSw6sAcsExtThdRwRtStFrwdBkwdPos_Val/1 -> Bus Creator49/7  "FrwdBkwdPos"
  PA_KeSMSw6sAcsExtThdRwRtStCshnFldUpwdDnwdPos_Val/1 -> Bus Creator49/4  "CshnFldUpwdDnwdPos"
  PA_KeSMSw6sAcsExtThdRwRtStFrwdBkwdPosMin_Val/1 -> Bus Creator49/9  "FrwdBkwdPosMin"
  Bus Creator49/1 -> Bus Creator52/2  "AcsExtThdRwRtSt"
  PA_KeSMSw6sAcsExtThdRwRtStBkReclnUpwdDnwdPos_Val/1 -> Bus Creator49/1  "BkReclnUpwdDnwdPos"
  PA_KeSMSw6sAcsExtThdRwRtStCshnFldUpwdDnwdPosMax_Val/1 -> Bus Creator49/5  "CshnFldUpwdDnwdPosMax"
  PA_KeSMSw6sAcsExtThdRwRtStBkReclnUpwdDnwdPosMin_Val/1 -> Bus Creator49/3  "BkReclnUpwdDnwdPosMin"
  PA_KeSMSw6sLugThdRwRtStBkReclnUpwdDnwdPosMin_Val/1 -> Bus Creator50/3  "BkReclnUpwdDnwdPosMin"
  PA_KeSMSw6sLugThdRwRtStFrwdBkwdPosMin_Val/1 -> Bus Creator50/9  "FrwdBkwdPosMin"
  PA_KeSMSw6sLugThdRwRtStBkReclnUpwdDnwdPos_Val/1 -> Bus Creator50/1  "BkReclnUpwdDnwdPos"
  PA_KeSMSw6sLugThdRwRtStFrwdBkwdPosMax_Val/1 -> Bus Creator50/8  "FrwdBkwdPosMax"
  PA_KeSMSw6sLugThdRwRtStCshnFldUpwdDnwdPos_Val/1 -> Bus Creator50/4  "CshnFldUpwdDnwdPos"
  PA_KeSMSw6sLugThdRwRtStFrwdBkwdPos_Val/1 -> Bus Creator50/7  "FrwdBkwdPos"
  Bus Creator50/1 -> Bus Creator52/3  "LugThdRwRtSt"
  PA_KeSMSw6sLugThdRwRtStBkReclnUpwdDnwdPosMax_Val/1 -> Bus Creator50/2  "BkReclnUpwdDnwdPosMax"
  PA_KeSMSw6sLugThdRwRtStCshnFldUpwdDnwdPosMin_Val/1 -> Bus Creator50/6  "CshnFldUpwdDnwdPosMin"
  PA_KeSMSw6sLugThdRwRtStCshnFldUpwdDnwdPosMax_Val/1 -> Bus Creator50/5  "CshnFldUpwdDnwdPosMax"
  Bus Creator51/1 -> Bus Creator52/4  "VIPThdRwRtSt"
  PA_KeSMSw6sVIPThdRwRtStBkReclnUpwdDnwdPos_Val/1 -> Bus Creator51/1  "BkReclnUpwdDnwdPos"
  PA_KeSMSw6sVIPThdRwRtStFrwdBkwdPosMin_Val/1 -> Bus Creator51/9  "FrwdBkwdPosMin"
  PA_KeSMSw6sVIPThdRwRtStFrwdBkwdPosMax_Val/1 -> Bus Creator51/8  "FrwdBkwdPosMax"
  PA_KeSMSw6sVIPThdRwRtStCshnFldUpwdDnwdPosMin_Val/1 -> Bus Creator51/6  "CshnFldUpwdDnwdPosMin"
  PA_KeSMSw6sVIPThdRwRtStFrwdBkwdPos_Val/1 -> Bus Creator51/7  "FrwdBkwdPos"
  PA_KeSMSw6sVIPThdRwRtStBkReclnUpwdDnwdPosMin_Val/1 -> Bus Creator51/3  "BkReclnUpwdDnwdPosMin"
  PA_KeSMSw6sVIPThdRwRtStCshnFldUpwdDnwdPos_Val/1 -> Bus Creator51/4  "CshnFldUpwdDnwdPos"
  PA_KeSMSw6sVIPThdRwRtStBkReclnUpwdDnwdPosMax_Val/1 -> Bus Creator51/2  "BkReclnUpwdDnwdPosMax"
  PA_KeSMSw6sVIPThdRwRtStCshnFldUpwdDnwdPosMax_Val/1 -> Bus Creator51/5  "CshnFldUpwdDnwdPosMax"
  Bus Creator52/1 -> Multiport Switch4/3
  PA_KeSMSwDltTrgtPos_Val184/1 -> Bus Creator63/5  "CshnFldUpwdDnwdPosMax"
  PA_KeSMSwFamilyMdThdRwLtStFrwdBkwdPosMin_Val/1 -> Bus Creator63/9  "FrwdBkwdPosMin"
  Bus Creator63/1 -> Bus Creator19/5  "FamlyRThdRwLtSt"
  PA_KeSMSwDltTrgtPos_Val183/1 -> Bus Creator63/3  "BkReclnUpwdDnwdPosMin"
  PA_KeSMSwFamilyMdThdRwLtStFrwdBkwdPosMax_Val/1 -> Bus Creator63/8  "FrwdBkwdPosMax"
  PA_KeSMSwDltTrgtPos_Val185/1 -> Bus Creator63/4  "CshnFldUpwdDnwdPos"
  PA_KeSMSwDltTrgtPos_Val181/1 -> Bus Creator63/2  "BkReclnUpwdDnwdPosMax"
  PA_KeSMSwDltTrgtPos_Val186/1 -> Bus Creator63/6  "CshnFldUpwdDnwdPosMin"
  PA_KeSMSwDltTrgtPos_Val182/1 -> Bus Creator63/1  "BkReclnUpwdDnwdPos"
  PA_KeSMSwFamilyMdThdRwLtStFrwdBkwdPos_Val/1 -> Bus Creator63/7  "FrwdBkwdPos"
  PA_KeSMSwDltTrgtPos_Val188/1 -> Bus Creator64/1  "BkReclnUpwdDnwdPos"
  PA_KeSMSwDltTrgtPos_Val192/1 -> Bus Creator64/6  "CshnFldUpwdDnwdPosMin"
  Bus Creator64/1 -> Bus Creator25/5  "FamlyLThdRwRtSt"
  PA_KeSMSwFamilyMdThdRwRtStFrwdBkwdPosMax_Val/1 -> Bus Creator64/8  "FrwdBkwdPosMax"
  PA_KeSMSwDltTrgtPos_Val189/1 -> Bus Creator64/3  "BkReclnUpwdDnwdPosMin"
  PA_KeSMSwDltTrgtPos_Val191/1 -> Bus Creator64/4  "CshnFldUpwdDnwdPos"
  PA_KeSMSwFamilyMdThdRwRtStFrwdBkwdPos_Val/1 -> Bus Creator64/7  "FrwdBkwdPos"
  PA_KeSMSwDltTrgtPos_Val187/1 -> Bus Creator64/2  "BkReclnUpwdDnwdPosMax"
  PA_KeSMSwFamilyMdThdRwRtStFrwdBkwdPosMin_Val/1 -> Bus Creator64/9  "FrwdBkwdPosMin"
  PA_KeSMSwDltTrgtPos_Val190/1 -> Bus Creator64/5  "CshnFldUpwdDnwdPosMax"
  PA_KeSMSwDltTrgtPos_Val147/1 -> Bus Creator71/3  "BkReclnUpwdDnwdPosMin"
  PA_KeSMSw6sFamilyMdThdRwLtStFrwdBkwdPos_Val/1 -> Bus Creator71/7  "FrwdBkwdPos"
  PA_KeSMSw6sFamilyMdThdRwLtStFrwdBkwdPosMax_Val/1 -> Bus Creator71/8  "FrwdBkwdPosMax"
  PA_KeSMSw6sFamilyMdThdRwLtStFrwdBkwdPosMin_Val/1 -> Bus Creator71/9  "FrwdBkwdPosMin"
  PA_KeSMSwDltTrgtPos_Val149/1 -> Bus Creator71/4  "CshnFldUpwdDnwdPos"
  PA_KeSMSwDltTrgtPos_Val145/1 -> Bus Creator71/2  "BkReclnUpwdDnwdPosMax"
  PA_KeSMSwDltTrgtPos_Val148/1 -> Bus Creator71/5  "CshnFldUpwdDnwdPosMax"
  PA_KeSMSwDltTrgtPos_Val150/1 -> Bus Creator71/6  "CshnFldUpwdDnwdPosMin"
  Bus Creator71/1 -> Bus Creator47/5  "FamlyRThdRwLtSt"
  PA_KeSMSwDltTrgtPos_Val146/1 -> Bus Creator71/1  "BkReclnUpwdDnwdPos"
  PA_KeSMSwDltTrgtPos_Val154/1 -> Bus Creator72/5  "CshnFldUpwdDnwdPosMax"
  PA_KeSMSwDltTrgtPos_Val151/1 -> Bus Creator72/2  "BkReclnUpwdDnwdPosMax"
  PA_KeSMSwDltTrgtPos_Val155/1 -> Bus Creator72/4  "CshnFldUpwdDnwdPos"
  PA_KeSMSwDltTrgtPos_Val153/1 -> Bus Creator72/3  "BkReclnUpwdDnwdPosMin"
  PA_KeSMSw6sFamilyMdThdRwRtStFrwdBkwdPos_Val/1 -> Bus Creator72/7  "FrwdBkwdPos"
  PA_KeSMSwDltTrgtPos_Val156/1 -> Bus Creator72/6  "CshnFldUpwdDnwdPosMin"
  PA_KeSMSw6sFamilyMdThdRwRtStFrwdBkwdPosMax_Val/1 -> Bus Creator72/8  "FrwdBkwdPosMax"
  PA_KeSMSw6sFamilyMdThdRwRtStFrwdBkwdPosMin_Val/1 -> Bus Creator72/9  "FrwdBkwdPosMin"
  PA_KeSMSwDltTrgtPos_Val152/1 -> Bus Creator72/1  "BkReclnUpwdDnwdPos"
  Bus Creator72/1 -> Bus Creator52/5  "FamlyLThdRwRtSt"
  PA_KeSMSw4sLyingMDSecRwLtStBkReclnUpwdDnwdPosMin_Val/1 -> Bus Creator73/3  "BkReclnUpwdDnwdPosMin"
  PA_KeSMSw4sLyingMDSecRwLtStHdrstUpwdDnwdPosMin_Val/1 -> Bus Creator73/6  "HdrstUpwdPosMin"
  PA_KeSMSw4sLyingMDSecRwLtStLgrstUpwdDnwdPos_Val/1 -> Bus Creator73/7  "LgrstUpwdPos"
  PA_KeSMSw4sLyingMDSecRwLtStLgrstUpwdDnwdPosMax_Val/1 -> Bus Creator73/8  "LgrstUpwdPosMax"
  PA_KeSMSw4sLyingMDSecRwLtStHdrstUpwdDnwdPos_Val/1 -> Bus Creator73/4  "HdrstUpwdPos"
  PA_KeSMSw4sLyingMDSecRwLtStBkReclnUpwdDnwdPos_Val/1 -> Bus Creator73/1  "BkReclnUpwdDnwdPos"
  PA_KeSMSw4sLyingMDSecRwLtStBkReclnUpwdDnwdPosMax_Val/1 -> Bus Creator73/2  "BkReclnUpwdDnwdPosMax"
  PA_KeSMSw4sLyingMDSecRwLtStHdrstUpwdDnwdPosMax_Val/1 -> Bus Creator73/5  "HdrstUpwdPosMax"
  PA_KeSMSw4sLyingMDSecRwLtStLgrstUpwdDnwdPosMin_Val/1 -> Bus Creator73/9  "LgrstUpwdPosMin"
  PA_KeSMSw4sLyingMDSecRwLtStLgrstOtwdInwdPosMax_Val/1 -> Bus Creator73/11  "LgrstOtwdInwdPosMax"
  PA_KeSMSw4sLyingMDSecRwLtStLgrstOtwdInwdPosMin_Val/1 -> Bus Creator73/12  "LgrstOtwdInwdPosMin"
  PA_KeSMSw4sLyingMDSecRwLtStLgrstOtwdInwdPos_Val/1 -> Bus Creator73/10  "LgrstOtwdInwdPos"
  PA_KeSMSw4sLyingMDSecRwLtStFtrstUpwdDnwdPosMax_Val/1 -> Bus Creator73/14  "FtrstUpwdDnwdPosMax"
  PA_KeSMSw4sLyingMDSecRwLtStFtrstUpwdDnwdPosMin_Val/1 -> Bus Creator73/15  "FtrstUpwdDnwdPosMin"
  PA_KeSMSw4sLyingMDSecRwLtStFtrstUpwdDnwdPos_Val/1 -> Bus Creator73/13  "FtrstUpwdDnwdPos"
  PA_KeSMSw4sLyingMDSecRwRtStLgrstUpwdPos_Val/1 -> Bus Creator74/7  "LgrstUpwdPos"
  PA_KeSMSw4sLyingMDSecRwRtStLgrstOtwdInwdPos_Val/1 -> Bus Creator74/10  "LgrstOtwdInwdPos"
  PA_KeSMSw4sLyingMDSecRwRtStLgrstOtwdInwdPosMin_Val/1 -> Bus Creator74/12  "LgrstOtwdInwdPosMin"
  PA_KeSMSw4sLyingMDSecRwRtStBkReclnUpwdDnwdPosMin_Val/1 -> Bus Creator74/3  "BkReclnUpwdDnwdPosMin"
